simulink model "RB_KAIROS_ImpControl_OpSpace_quat_2020b_safety"  (R2020b)
(part 4 of 17)

t4722 = t17.*(t71-t391).*(-5.48359106408232e-4);
t4725 = t8.*(t71-t391).*(-5.187945860934245e-5);
t4740 = t16.*(t71-t391).*(-4.67845486573025e-5);
t4762 = t8.*t17.*(t71-t391).*(-2.74179553204116e-4);
t4779 = t3296.*(t386+t16.*(t69-t347)).*(-1.0./4.0);
t4788 = ((t395+t9.*(t48-t349)).*(t689-t740))./4.0;
t4790 = -t4761;
t4794 = t3286.*(t386+t16.*(t69-t347)).*(-1.0./4.0);
t4798 = t155+t255+t480+t841+t1384;
t4802 = t618.*(-8.36241330891889e-4);
t4803 = (t3296.*(t386+t16.*(t69-t347)))./4.0;
t4804 = t16.*(t71-t391).*(-2.454825983680473e-3);
t4807 = -t4789;
t4813 = (t3286.*(t386+t16.*(t69-t347)))./4.0;
t4817 = (t395+t9.*(t48-t349)).*(t1130-t16.*t17.*1.2516e-2).*(-1.0./4.0);
t4821 = t618.*8.36241330891889e-4;
t4829 = -t4815;
t4831 = -t4816;
t4832 = ((t395+t9.*(t48-t349)).*(t1130-t16.*t17.*1.2516e-2))./4.0;
t4837 = t1073+t1266+t2236;
t4848 = -t4839;
t4849 = t479+t534+t941+t1285;
t4883 = t1475+t3915;
t4888 = -t4878;
t4889 = t17.*(t380-t392).*(-2.74179553204116e-4);
t4901 = -t4886;
t4903 = t9.*(t380-t392).*(-8.36241330891889e-4);
t4904 = t17.*(t380-t392).*2.74179553204116e-4;
t4909 = -t4895;
t4910 = -t4897;
t4911 = -t4898;
t4921 = t3239.*(t383+t9.*(t380-t392)).*(-1.0./4.0);
t4929 = -t4915;
t4933 = -t4919;
t4935 = (t3239.*(t383+t9.*(t380-t392)))./4.0;
t4963 = (t454.*t4415)./4.0;
t4965 = -t4954;
t4967 = (t440.*t4432)./4.0;
t4968 = -t4957;
t4969 = -t4958;
t4971 = -t4961;
t4975 = t439.*t4533;
t4977 = t6.*t3270.*2.46255173325e-2;
t4985 = (t454.*t4495)./4.0;
t4988 = (t439.*t4476)./4.0;
t4991 = -t4979;
t4995 = t4383.*(t71-t391).*(-1.0./4.0);
t5000 = t4410.*(t77-t390).*(-1.0./4.0);
t5007 = t469+t897+t1178+t1491;
t5013 = -t4993;
t5017 = (t4383.*(t71-t391))./4.0;
t5020 = (t440.*t4515)./4.0;
t5032 = t3624.*(-3.867742437e-3);
t5035 = (t540.*t4410)./4.0;
t5036 = (t440.*t4551)./4.0;
t5037 = t4471.*(t71-t391).*(-1.0./4.0);
t5040 = (t439.*t4527)./4.0;
t5049 = (t439.*t4532)./4.0;
t5055 = t3624.*3.867742437e-3;
t5057 = (t4471.*(t71-t391))./4.0;
t5058 = t439.*t4689;
t5063 = t4477.*(t60-t394).*(-1.0./4.0);
t5071 = t4510.*(t71-t391).*(-1.0./4.0);
t5075 = (t4477.*(t60-t394))./4.0;
t5084 = t4506.*3.587895;
t5085 = t4507.*3.587895;
t5089 = (t4510.*(t71-t391))./4.0;
t5090 = (t539.*t4477)./4.0;
t5091 = (t439.*t4635)./4.0;
t5094 = t16.*t4477.*(t71-t391).*(-1.0./2.0);
t5096 = t4506.*3.228604;
t5097 = t4507.*3.228604;
t5102 = t4531.*(t71-t391).*(-1.0./4.0);
t5103 = t4534.*(t60-t394).*(-1.0./4.0);
t5109 = t4537.*1.225946;
t5110 = t4542.*1.225946;
t5112 = t4544.*1.225946;
t5114 = (t4531.*(t71-t391))./4.0;
t5120 = t4537.*3.587895;
t5123 = t4541.*3.587895;
t5124 = t4542.*3.587895;
t5126 = t4544.*3.587895;
t5129 = t8.*t4527.*(t71-t391).*(-1.0./4.0);
t5133 = (t539.*t4534)./4.0;
t5134 = (t439.*t4711)./4.0;
t5136 = t16.*t4534.*(t71-t391).*(-1.0./4.0);
t5143 = t4619.*(t71-t391).*(-1.0./4.0);
t5144 = t4582.*1.666555;
t5148 = t4716.*(t71-t391);
t5149 = t4581.*1.225946;
t5150 = t4582.*1.225946;
t5152 = t4586.*1.225946;
t5157 = t4723.*(t71-t391);
t5159 = t4578.*3.587895;
t5162 = t4581.*3.587895;
t5171 = (t4619.*(t71-t391))./4.0;
t5216 = t611+t2361+t2731;
t5218 = t613+t2365+t2733;
t5222 = (t6.*t5118)./4.0;
t5239 = (t14.*t5139)./4.0;
t5241 = -t5229;
t5244 = (t7.*t5163)./4.0;
t5256 = (t13.*t14.*t5118)./2.0;
t5263 = t4541.*1.8732399795e-1;
t5264 = t4544.*1.8732399795e-1;
t5265 = t4537.*9.5384188575e-2;
t5266 = t4542.*9.5384188575e-2;
t5269 = (t6.*t13.*t5139)./4.0;
t5271 = (t14.*t15.*t5163)./4.0;
t5276 = t4527.*(t380-t392).*(-1.0./2.0);
t5278 = t5.*t14.*t5139.*(-1.0./4.0);
t5280 = t4578.*1.8732399795e-1;
t5284 = t4581.*9.5384188575e-2;
t5288 = (t13.*t42.*t5139)./2.0;
t5294 = (t17.*t5233)./4.0;
t5298 = -t5282;
t5300 = -t5285;
t5306 = (t15.*t5254)./4.0;
t5310 = (t9.*t16.*t5233)./4.0;
t5317 = t16.*t4024.*4.38178973375e-3;
t5328 = (t5.*t5270)./4.0;
t5329 = t1097+t4772;
t5333 = t4432.*(t395+t9.*(t48-t349)).*(-1.0./4.0);
t5335 = (t7.*t14.*t5254)./4.0;
t5339 = -t5326;
t5341 = (t223.*t5118)./2.0;
t5346 = (t4432.*(t395+t9.*(t48-t349)))./4.0;
t5349 = (t12.*t13.*t5270)./2.0;
t5350 = (t9.*t5291)./4.0;
t5356 = t4477.*(t386+t16.*(t69-t347)).*(-1.0./4.0);
t5367 = -t5355;
t5368 = (t4477.*(t386+t16.*(t69-t347)))./4.0;
t5372 = (t7.*t5307)./4.0;
t5373 = (t16.*t17.*t5291)./4.0;
t5374 = (t6.*t5309)./4.0;
t5377 = (t319.*t5139)./2.0;
t5378 = (t320.*t5139)./2.0;
t5380 = t4515.*(t395+t9.*(t48-t349)).*(-1.0./4.0);
t5383 = -t5370;
t5387 = t4551.*(t395+t9.*(t48-t349)).*(-1.0./4.0);
t5389 = (t321.*t5163)./2.0;
t5394 = (t4515.*(t395+t9.*(t48-t349)))./4.0;
t5397 = t4534.*(t386+t16.*(t69-t347)).*(-1.0./4.0);
t5400 = (t14.*t15.*t5307)./2.0;
t5401 = (t13.*t14.*t5309)./2.0;
t5402 = (t4551.*(t395+t9.*(t48-t349)))./4.0;
t5406 = (t4534.*(t386+t16.*(t69-t347)))./4.0;
t5407 = -t5399;
t5410 = t6.*t4252.*2.46255173325e-2;
t5413 = -t5392;
t5414 = -t5393;
t5420 = -t5412;
t5426 = -t5416;
t5427 = (t325.*t5233)./2.0;
t5429 = (t225.*t5254)./2.0;
t5435 = -t5421;
t5447 = -t5432;
t5464 = -t5453;
t5473 = t4410.*(t383+t9.*(t380-t392)).*(-1.0./4.0);
t5483 = -t5462;
t5492 = (t4410.*(t383+t9.*(t380-t392)))./4.0;
t5497 = t3757+t3812;
t5504 = (t229.*t5291)./2.0;
t5506 = -t5498;
t5513 = (t223.*t5309)./4.0;
t5514 = t4506.*4.4422362436e-2;
t5515 = t3774+t3836;
t5516 = t4507.*6.3364582104e-2;
t5518 = t1458+t1480+t1953+t2002;
t5523 = t2079+t2253+t3330;
t5529 = -t5521;
t5532 = t744+t1015+t2242+t2264;
t5536 = t12.*t4507.*4.4422362436e-2;
t5542 = t12.*t4506.*6.3364582104e-2;
t5545 = (t321.*t5307)./4.0;
t5548 = t5163.*(t71-t391).*(-1.0./4.0);
t5551 = -t5533;
t5552 = t1576+t1660+t1996+t2021;
t5556 = -t5537;
t5561 = t1141+t1500+t2016+t2266;
t5564 = (t440.*t5233)./4.0;
t5566 = (t5163.*(t71-t391))./4.0;
t5573 = (t7.*t5494)./2.0;
t5580 = t1651+t1698+t2029+t2136;
t5581 = t4586.*2.5171736245e-2;
t5582 = t1371+t1797+t1969+t2179;
t5592 = t4582.*7.326866269e-3;
t5600 = t12.*t583.*t4507.*8.9697375e-1;
t5603 = (t15.*t5508)./2.0;
t5604 = t851+t1215+t2293+t2350;
t5606 = (t6.*t5517)./4.0;
t5609 = t1275+t1634+t2173+t2231;
t5614 = (t14.*t15.*t5494)./4.0;
t5625 = t1426+t1865+t1986+t2171;
t5628 = t1303+t5064;
t5634 = t951+t5095;
t5636 = (t7.*t14.*t5508)./4.0;
t5637 = t14.*t4557.*2.46255173325e-2;
t5640 = t987+t1598+t2244+t2344;
t5644 = t1348+t1686+t2218+t2340;
t5645 = (t13.*t14.*t5517)./4.0;
t5667 = -t5653;
t5680 = -t5669;
t5688 = (t439.*t5312)./4.0;
t5691 = (t439.*t5314)./4.0;
t5693 = t5291.*(t79-t358).*(-1.0./4.0);
t5699 = t571+t886+t1106+t1441+t1467;
t5705 = (t5291.*(t79-t358))./4.0;
t5712 = t5285.*1.225946;
t5720 = t5282.*3.587895;
t5721 = t5285.*3.587895;
t5730 = t17.*t4772.*1.13264871585e-2;
t5731 = -t5722;
t5736 = t5307.*(t71-t391).*(-1.0./4.0);
t5747 = (t225.*t5508)./4.0;
t5757 = (t321.*t5494)./4.0;
t5767 = (t223.*t5517)./2.0;
t5788 = -t5780;
t5793 = t6.*t5780;
t5800 = -t5790;
t5808 = t5282.*1.8732399795e-1;
t5812 = t5285.*9.5384188575e-2;
t5822 = t5392.*1.666555;
t5827 = t5392.*1.225946;
t5828 = t5393.*1.225946;
t5849 = -t5835;
t5850 = -t5836;
t5856 = -t5839;
t5857 = -t5840;
t5861 = t8.*t5835;
t5870 = (t6.*t5783)./4.0;
t5876 = t6.*t5839;
t5878 = -t5868;
t5881 = (t14.*t5807)./4.0;
t5883 = -t5872;
t5891 = (t13.*t14.*t5783)./4.0;
t5898 = -t5885;
t5899 = (t16.*t5810)./4.0;
t5904 = (t6.*t13.*t5807)./2.0;
t5906 = t5233.*(t395+t9.*(t48-t349)).*(-1.0./4.0);
t5917 = (t7.*t5829)./4.0;
t5922 = (t13.*t35.*t5783)./2.0;
t5924 = -t5903;
t5927 = (t5233.*(t395+t9.*(t48-t349)))./4.0;
t5930 = (t7.*t16.*t5810)./2.0;
t5931 = (t8.*t15.*t5810)./2.0;
t5934 = -t5913;
t5937 = -t5918;
t5938 = t5494.*(t71-t391).*(-1.0./2.0);
t5944 = -t5920;
t5945 = -t5921;
t5948 = (t16.*t5866)./4.0;
t5950 = (t15.*t16.*t5821)./2.0;
t5954 = (t14.*t15.*t5829)./2.0;
t5959 = (t5494.*(t71-t391))./2.0;
t5960 = -t5940;
t5962 = -t5942;
t5964 = t8.*t5903;
t5968 = (t8.*t5875)./4.0;
t5970 = (t16.*t5877)./4.0;
t5972 = (t15.*t44.*t5810)./4.0;
t5980 = t223.*t5780;
t5983 = -t5956;
t5984 = -t5957;
t5985 = -t5958;
t5987 = -t5965;
t5989 = (t8.*t5879)./4.0;
t5991 = (t17.*t5888)./4.0;
t6004 = (t8.*t15.*t5866)./4.0;
t6013 = (t15.*t5894)./4.0;
t6017 = -t6000;
t6020 = t7.*t16.*t5866.*(-1.0./4.0);
t6023 = (t15.*t16.*t5879)./4.0;
t6026 = (t3720.*t4681)./4.0;
t6027 = -t6008;
t6034 = -t6015;
t6037 = (t15.*t44.*t5866)./2.0;
t6039 = t7.*t8.*t5879.*(-1.0./4.0);
t6044 = (t7.*t14.*t5894)./2.0;
t6049 = -t6033;
t6051 = t7.*t5064.*1.059103943995e-1;
t6056 = (t15.*t39.*t5879)./2.0;
t6057 = -t6042;
t6061 = t223.*t5839;
t6065 = -t6050;
t6073 = (t223.*t5783)./2.0;
t6074 = (t224.*t5783)./2.0;
t6076 = t323.*t5835;
t6081 = (t8.*(t1254+t1943+t9.*t439.*1.196e-3+t439.*t1083))./4.0;
t6082 = t15.*t5095.*1.059103943995e-1;
t6086 = (t227.*t5810)./4.0;
t6087 = (t6.*t5988)./2.0;
t6089 = (t9.*t5990)./4.0;
t6100 = (t15.*t16.*(t1254+t1943+t9.*t439.*1.196e-3+t439.*t1083))./4.0;
t6111 = (t319.*t5807)./2.0;
t6113 = (t15.*t16.*t5981)./4.0;
t6115 = -t6098;
t6118 = (t13.*t14.*t5988)./4.0;
t6120 = -t6099;
t6121 = (t454.*t5709)./2.0;
t6122 = (t8.*t6029)./4.0;
t6128 = (t14.*t15.*t6005)./4.0;
t6129 = (t321.*t5829)./4.0;
t6132 = -t6119;
t6141 = (t227.*t5866)./2.0;
t6142 = (t228.*t5866)./2.0;
t6144 = (t323.*t5821)./4.0;
t6147 = t1422+t1647+t1671+t1848+t2236;
t6151 = t223.*t5942;
t6156 = -t6136;
t6161 = -t6139;
t6162 = -t6140;
t6164 = (t227.*t5877)./2.0;
t6165 = (t16.*t6064)./4.0;
t6171 = -t6152;
t6174 = t9.*t5213.*1.13264871585e-2;
t6176 = t323.*t5903;
t6179 = -t6163;
t6180 = t17.*t5217.*1.13264871585e-2;
t6184 = t16.*t321.*t5810.*(-1.0./4.0);
t6186 = (t225.*t5894)./4.0;
t6189 = -t6172;
t6192 = t5723.*(t71-t391).*(-1.0./4.0);
t6194 = (t323.*t5875)./2.0;
t6200 = -t6181;
t6201 = (t440.*t5761)./4.0;
t6202 = -t6185;
t6208 = (t325.*t5888)./4.0;
t6209 = (t323.*t5879)./2.0;
t6210 = (t324.*t5879)./2.0;
t6212 = -t6199;
t6219 = t16.*t321.*t5866.*(-1.0./4.0);
t6220 = t439.*t5835;
t6229 = -t6215;
t6232 = (t404.*t5866)./4.0;
t6235 = (t370.*t5879)./4.0;
t6238 = t9.*t439.*t5763.*(-1.0./4.0);
t6245 = -t6233;
t6247 = -t6234;
t6254 = t5777.*(t71-t391).*(-1.0./4.0);
t6258 = -t6249;
t6260 = (t223.*t5988)./2.0;
t6262 = (t229.*t5990)./4.0;
t6264 = (t323.*(t1254+t1943+t9.*t439.*1.196e-3+t439.*t1083))./4.0;
t6265 = (t440.*t5837)./4.0;
t6266 = (t5777.*(t71-t391))./4.0;
t6267 = t12.*t3350.*t4507.*8.07151e-1;
t6269 = (t323.*t5981)./2.0;
t6272 = (t439.*t5821)./4.0;
t6287 = t12.*t3405.*t4506.*8.07151e-1;
t6290 = t5810.*(t48-t349).*(-1.0./4.0);
t6291 = (t454.*t5847)./4.0;
t6293 = -t6277;
t6295 = t439.*t5903;
t6298 = (t3270.*t5137)./2.0;
t6303 = (t321.*t6005)./2.0;
t6307 = -t6292;
t6308 = -t6294;
t6311 = t17.*t439.*t5837.*(-1.0./4.0);
t6313 = (t323.*t6029)./4.0;
t6314 = (t439.*t5875)./4.0;
t6315 = (t227.*t6064)./4.0;
t6320 = t5810.*(t60-t394).*(-1.0./4.0);
t6332 = t5866.*(t48-t349).*(-1.0./4.0);
t6334 = (t440.*t5888)./2.0;
t6335 = -t6318;
t6336 = (t439.*t5879)./4.0;
t6340 = (t2008.*t5509)./4.0;
t6343 = t5829.*(t71-t391).*(-1.0./2.0);
t6348 = (t5866.*(t48-t349))./4.0;
t6349 = (t539.*t5810)./4.0;
t6351 = t5877.*(t48-t349).*(-1.0./4.0);
t6353 = t3720+t5080;
t6354 = t16.*t5810.*(t71-t391).*(-1.0./4.0);
t6358 = (t2087.*t5509)./4.0;
t6361 = t5845.*(t71-t391).*(-1.0./4.0);
t6362 = (t5829.*(t71-t391))./2.0;
t6365 = t5393.*2.5171736245e-2;
t6366 = (t5877.*(t48-t349))./4.0;
t6373 = t5392.*7.326866269e-3;
t6381 = (t5845.*(t71-t391))./4.0;
t6385 = t1023+t2359+t3051+t3184;
t6401 = t16.*t5866.*(t71-t391).*(-1.0./4.0);
t6408 = t1570+t2432+t2918+t3015;
t6410 = (t539.*t5866)./2.0;
t6413 = (t439.*t5981)./4.0;
t6417 = (t439.*(t1254+t1943+t9.*t439.*1.196e-3+t439.*t1083))./2.0;
t6422 = t8.*t5879.*(t71-t391).*(-1.0./4.0);
t6427 = t12.*t4507.*(t85+t338+t362+t375+t408+t5.*t12.*(7.9e+1./2.5e+2)).*8.9697375e-1;
t6430 = t4506+t4588;
t6433 = t5879.*(t113-t409).*(-1.0./2.0);
t6436 = t5990.*(t79-t358).*(-1.0./2.0);
t6438 = (t439.*t6029)./2.0;
t6441 = (t5879.*(t113-t409))./2.0;
t6442 = t4537+t4581;
t6447 = t4507+t4656;
t6454 = t6005.*(t71-t391).*(-1.0./4.0);
t6455 = t4541+t4651;
t6463 = (t6005.*(t71-t391))./4.0;
t6473 = t6064.*(t48-t349).*(-1.0./2.0);
t6503 = (t12.*t4507.*t4681)./4.0;
t6509 = t5879.*(t380-t392).*(-1.0./4.0);
t6511 = t5761.*(t395+t9.*(t48-t349)).*(-1.0./4.0);
t6518 = (t5879.*(t380-t392))./4.0;
t6522 = (t5761.*(t395+t9.*(t48-t349)))./4.0;
t6523 = -t6512;
t6527 = (t4024.*t5083)./2.0;
t6546 = t2436+t2455+t2857+t2929;
t6558 = -t6551;
t6563 = t5810.*(t386+t16.*(t69-t347)).*(-1.0./4.0);
t6566 = t5837.*(t395+t9.*(t48-t349)).*(-1.0./4.0);
t6567 = t7.*t5613.*1.059103943995e-1;
t6570 = -t6560;
t6571 = (t5810.*(t386+t16.*(t69-t347)))./4.0;
t6577 = -t6569;
t6581 = t15.*t5648.*1.059103943995e-1;
t6584 = t5866.*(t386+t16.*(t69-t347)).*(-1.0./4.0);
t6590 = t655+t1385+t1708+t1730+t1883+t2023;
t6594 = (t5866.*(t386+t16.*(t69-t347)))./4.0;
t6598 = -t6591;
t6600 = -t6592;
t6605 = t5888.*(t395+t9.*(t48-t349)).*(-1.0./4.0);
t6615 = t946+t1120+t1676+t1696+t1911+t2015;
t6617 = (t5888.*(t395+t9.*(t48-t349)))./4.0;
t6624 = (t12.*t4507.*t4916)./4.0;
t6625 = (t12.*t4506.*t4936)./4.0;
t6631 = t5763.*(t383+t9.*(t380-t392)).*(-1.0./2.0);
t6633 = t1185+t1248+t1522+t1561+t1945+t2035;
t6649 = t6.*t6223.*6.8635e-3;
t6656 = t15.*t6175.*8.639075e-2;
t6659 = t7.*t6196.*8.639075e-2;
t6663 = -t6651;
t6673 = t1025+t1195+t1726+t1732+t2037+t2117;
t6675 = t836+t1398+t1617+t1705+t2042+t2103;
t6687 = t1413+t1536+t1622+t1642+t2006+t2055;
t6726 = t7.*t5806.*1.059103943995e-1;
t6735 = (t4774.*(t2821-t2864))./4.0;
t6767 = t1902+t6223;
t6772 = t15.*t5860.*1.059103943995e-1;
t6781 = t724+t1606+t2375+t2945+t3128;
t6803 = t1324+t1498+t1852+t1856+t2081+t2326;
t6821 = (t4557.*t5115)./4.0;
t6822 = (t3270.*t5755)./2.0;
t6850 = -t6823;
t6873 = (t4024.*t5441)./2.0;
t6890 = -t6861;
t6951 = t1213+t1742+t1859+t1870+t2346+t2378;
t6983 = t1755+t1790+t1829+t1842+t2322+t2352;
t6992 = (t3270.*t5826)./4.0;
t7001 = (t3275.*t5843)./4.0;
t7113 = t722+t2456+t2481+t2925+t2947;
t7124 = t849+t2478+t2484+t2828+t2942;
t7132 = t5012+t5065;
t7133 = t6.*t7108;
t7134 = t14.*t7108;
t7178 = (t4517.*t5433)./4.0;
t7186 = (t536.*t6713)./4.0;
t7200 = -t7191;
t7215 = t3095+t3159+t3371+t3376;
t7217 = t3049+t3183+t3382+t3417;
t7220 = (t554.*t6713)./4.0;
t7238 = (t583.*t6693)./4.0;
t7242 = -t7228;
t7253 = (t3270.*t6222)./4.0;
t7255 = (t3275.*t6223)./4.0;
t7262 = (t4772.*t5433)./4.0;
t7265 = (t4252.*t5750)./4.0;
t7268 = -t7256;
t7276 = -t7254;
t7289 = t14.*t6750.*6.8635e-3;
t7303 = -t7275;
t7305 = -t7278;
t7306 = -t7279;
t7317 = -t7293;
t7320 = t5168+t5219;
t7323 = -t7302;
t7393 = (t1490.*t6713)./4.0;
t7423 = -t7399;
t7424 = -t7401;
t7436 = -t7429;
t7450 = (t1920.*t6713)./2.0;
t7453 = (t4557.*t5739)./4.0;
t7454 = t298+t7252;
t7459 = -t7452;
t7466 = (t4884.*t5543)./4.0;
t7477 = (t4959.*t5478)./4.0;
t7481 = -t7.*(t263-t7252);
t7483 = -t15.*(t263-t7252);
t7493 = t5478.*(t2959-t2967).*(-1.0./4.0);
t7504 = (t5478.*(t2959-t2967))./4.0;
t7519 = t5509.*(t2959-t2967).*(-1.0./4.0);
t7527 = -t7.*(-t262+t5078+t5282);
t7528 = -t15.*(-t262+t5078+t5282);
t7532 = (t5509.*(t2959-t2967))./4.0;
t7543 = (t3738.*t6397)./4.0;
t7558 = t7.*(-t262+t5078+t5282);
t7559 = t15.*(-t262+t5078+t5282);
t7563 = (t4557.*t5843)./2.0;
t7573 = (t5062.*t5478)./4.0;
t7591 = t189+t248+t7254;
t7604 = (t4896.*t5696)./4.0;
t7625 = (t4879.*t5713)./4.0;
t7628 = -t7606;
t7639 = t188+t247+t5044+t5285;
t7651 = -t7632;
t7655 = -t7637;
t7657 = (t4938.*t5696)./4.0;
t7668 = (t5696.*(t2889-t2921))./4.0;
t7674 = (t4917.*t5713)./4.0;
t7676 = t2354+t2896+t2939+t3103+t3145;
t7687 = (t5713.*(t2812-t2860))./4.0;
t7694 = (t2561.*t6750)./4.0;
t7697 = t7254.*1.225946;
t7699 = -t7680;
t7703 = t7252.*3.587895;
t7705 = t7254.*3.587895;
t7708 = (t2701.*t6713)./2.0;
t7709 = (t2701.*t6713)./4.0;
t7731 = t7275.*1.225946;
t7732 = t7277.*1.225946;
t7735 = t7278.*1.225946;
t7736 = t7279.*1.225946;
t7743 = t7275.*3.587895;
t7745 = t7278.*3.587895;
t7748 = t7277.*1.666555;
t7831 = t7399.*1.666555;
t7832 = t7401.*1.666555;
t7833 = t7399.*1.225946;
t7834 = t7254.*9.5384188575e-2;
t7835 = t7401.*1.225946;
t7845 = t7252.*1.8732399795e-1;
t7888 = (t3254.*t6750)./4.0;
t7907 = (t4557.*t6223)./2.0;
t7943 = -t7927;
t7952 = t5439+t5461;
t7955 = t15.*(t263-t7252).*(-1.666555);
t7959 = t7.*(t263-t7252).*(-1.225946);
t7960 = t15.*(t263-t7252).*(-1.225946);
t7970 = (t5365.*t5524)./4.0;
t8002 = t6750.*(t263-t283-t310+t1265).*(-1.0./2.0);
t8007 = (t5450.*t5478)./4.0;
t8008 = (t6693.*(t85+t338+t362+t375+t408+t5.*t12.*(7.9e+1./2.5e+2)))./2.0;
t8009 = (t3720.*t6713)./2.0;
t8020 = (t6750.*(t263-t283-t310+t1265))./2.0;
t8033 = (t4884.*(-t1272-t1479+t1647+t1848+t2236))./4.0;
t8035 = -t8019;
t8046 = t5.*t7108.*2.01382560198e-1;
t8047 = t721+t2454+t2483+t2911+t2924+t2948;
t8048 = -t8036;
t8053 = t823+t2477+t2485+t2814+t2856+t2951;
t8072 = t917+t1776+t2469+t2475+t3495+t3591;
t8081 = -t8061;
t8082 = -t8064;
t8084 = (t5331.*t5716)./4.0;
t8089 = -t8069;
t8095 = t9.*t7538.*1.539925e-2;
t8096 = t17.*t7540.*1.539925e-2;
t8110 = -t8093;
t8142 = -t8125;
t8147 = -t8130;
t8153 = -t8137;
t8204 = t7277.*7.326866269e-3;
t8217 = t7279.*2.5171736245e-2;
t8231 = -t8206;
t8232 = -t8210;
t8233 = -t8211;
t8256 = t1004+t2355+t2882+t2931+t3036+t3178;
t8261 = (t5064.*t6175)./4.0;
t8267 = (t5509.*t5681)./4.0;
t8272 = t248+t364+t1259+t7254;
t8278 = t4660+t6538;
t8297 = t3742+t4992+t5045;
t8299 = (t5331.*t5884)./4.0;
t8303 = t4721+t6539;
t8305 = (t5095.*t6196)./4.0;
t8333 = (t4252.*t6750)./2.0;
t8349 = -t8337;
t8394 = t7.*(t263-t7252).*(-2.5171736245e-2);
t8398 = t15.*(t263-t7252).*(-7.326866269e-3);
t8412 = t15.*(t263-t7252).*7.326866269e-3;
t8431 = (t12.*t4507.*t6713)./4.0;
t8441 = -t8435;
t8447 = t12.*t13.*t6713.*(t2425-t2468).*(-1.0./4.0);
t8448 = t583.*(t5453+t5.*(t2959-t2967).*3.587895).*(-1.0./4.0);
t8454 = (t12.*t13.*t6713.*(t2425-t2468))./4.0;
t8455 = (t583.*(t5453+t5.*(t2959-t2967).*3.587895))./4.0;
t8468 = t13.*(t5462+t5.*(t2959-t2967).*3.228604).*(-6.23745e-2);
t8475 = -t8465;
t8478 = -t8466;
t8482 = t13.*(t5462+t5.*(t2959-t2967).*3.228604).*6.23745e-2;
t8484 = (t4569.*t6750)./2.0;
t8485 = (t4557.*t6762)./2.0;
t8491 = -t8479;
t8492 = -t8480;
t8537 = t1572.*(t5453+t5.*(t2959-t2967).*3.587895).*(-1.0./4.0);
t8548 = (t1572.*(t5453+t5.*(t2959-t2967).*3.587895))./4.0;
t8606 = t2433+t2449+t3153+t3171+t3223+t3232;
t8634 = t8331.*(-7.35522e-1);
t8638 = t8331.*(-1.666555);
t8643 = t8331.*7.35522e-1;
t8646 = t8331.*1.666555;
t8651 = t8350.*(-7.35522e-1);
t8658 = t8350.*7.35522e-1;
t8670 = (t5696.*t6104)./2.0;
t8674 = (t5713.*t6092)./2.0;
t8675 = t7.*t8285.*8.639075e-2;
t8690 = t297+t309+t1056+t1250+t5078+t5282;
t8692 = t15.*t8310.*8.639075e-2;
t8784 = -t8768;
t8836 = -t8819;
t8841 = -t8823;
t8842 = -t8824;
t8874 = t5713.*(t985+t3399-t13.*t42.*1.01140545e-1-t7.*t223.*5.034347249e-2).*(-1.0./4.0);
t8898 = (t5713.*(t985+t3399-t13.*t42.*1.01140545e-1-t7.*t223.*5.034347249e-2))./4.0;
t8917 = t5193+t6984;
t8922 = t5210+t6985;
t8927 = t5201+t6981;
t8928 = -t8921;
t8942 = (t3489.*t7980)./4.0;
t8952 = t8331.*(-5.01208083475e-2);
t8962 = t8331.*5.01208083475e-2;
t8971 = t8350.*(-3.867742437e-3);
t8995 = t5490+t6693;
t9016 = (t3752.*(t917-t1669+t2469+t2475+t3495+t3591))./4.0;
t9055 = t5.*t8728.*6.23745e-2;
t9061 = t13.*t8734.*6.23745e-2;
t9072 = t264+t5048+t7278;
t9095 = (t3266.*t8437)./4.0;
t9099 = -t7.*(-t211+t5081+t7275);
t9101 = -t8.*(-t211+t5081+t7275);
t9102 = -t15.*(-t211+t5081+t7275);
t9103 = -t16.*(-t211+t5081+t7275);
t9119 = t7.*(-t211+t5081+t7275);
t9121 = t15.*(-t211+t5081+t7275);
t9122 = (t3362.*t8437)./4.0;
t9130 = (t8437.*(t923-t1076))./4.0;
t9133 = t8477.*(t701-t775).*(-1.0./4.0);
t9135 = (t3424.*t8438)./4.0;
t9141 = (t8477.*(t701-t775))./4.0;
t9143 = (t5696.*t6966)./2.0;
t9146 = (t5713.*t6928)./2.0;
t9157 = (t3365.*t8477)./4.0;
t9161 = (t3455.*t8477)./4.0;
t9168 = (t3249.*(t2433+t2449-t3048-t3102+t3223+t3232))./4.0;
t9184 = t6.*(-t262+t1056+t1250+t5078+t5282+t4.*t13.*1.0442e-1).*2.46255173325e-2;
t9201 = (t3424.*t8609)./4.0;
t9228 = t4936+t5438+t5482;
t9303 = (t4265.*t8437)./2.0;
t9315 = (t4152.*t8477)./2.0;
t9316 = t8.*(-t211+t5081+t7275).*(-7.35522e-1);
t9318 = t8.*(-t211+t5081+t7275).*(-1.666555);
t9320 = t16.*(-t211+t5081+t7275).*(-1.666555);
t9380 = (t3350.*t8734)./4.0;
t9384 = (t3405.*t8728)./4.0;
t9515 = t12.*t4507.*t8156.*8.07151e-1;
t9523 = t12.*t4506.*(-t3405+t4994+t5076).*(-8.07151e-1);
t9526 = t6750.*(t4650+t34.*(t2425-t2468)).*(-1.0./4.0);
t9527 = (t4774.*t8437)./4.0;
t9531 = (t6750.*(t4650+t34.*(t2425-t2468)))./4.0;
t9571 = t5.*t9218.*6.23745e-2;
t9583 = t12.*t13.*t9218.*6.23745e-2;
t9586 = t13.*(t2720-t8734).*6.23745e-2;
t9602 = t5.*t12.*(t2720-t8734).*6.23745e-2;
t9611 = t8.*(-t211+t5081+t7275).*(-5.01208083475e-2);
t9616 = (t1572.*t9215)./4.0;
t9619 = t16.*(-t211+t5081+t7275).*(-1.17633784675e-2);
t9621 = t8.*(-t211+t5081+t7275).*5.01208083475e-2;
t9628 = t16.*(-t211+t5081+t7275).*1.17633784675e-2;
t9643 = -t9638;
t9644 = -t9639;
t9686 = t269+t865+t1258+t5081+t7275;
t9702 = (t5696.*t7980)./2.0;
t9755 = (t5277.*t8437)./2.0;
t9812 = (t5290.*t8477)./2.0;
t9912 = (t3396.*t9218)./4.0;
t9914 = t5750.*(t263+t1265-t7252-t5.*t12.*1.0442e-1).*(-1.0./4.0);
t9915 = (t3356.*(t2720-t8734))./4.0;
t9934 = (t5524.*t8477)./2.0;
t9940 = (t9215.*(t85+t338+t362+t375+t408+t5.*t12.*(7.9e+1./2.5e+2)))./4.0;
t9976 = (t5713.*t8438)./2.0;
t9977 = (t5716.*t8437)./2.0;
t10108 = t6175.*(t7.*(t4650+t34.*(t2425-t2468))+t47.*(t2425-t2468)).*(-1.0./4.0);
t10109 = (t5713.*t8609)./4.0;
t10110 = (t5884.*t8437)./4.0;
t10114 = (t6175.*(t7.*(t4650+t34.*(t2425-t2468))+t47.*(t2425-t2468)))./4.0;
t10123 = t6196.*(t4654+t15.*(t4650+t34.*(t2425-t2468))).*(-1.0./4.0);
t10129 = (t6196.*(t4654+t15.*(t4650+t34.*(t2425-t2468))))./4.0;
t10143 = (t6713.*t7734)./4.0;
t10151 = (t12.*t4507.*t9218)./4.0;
t10156 = t12.*t13.*t9218.*(t2425-t2468).*(-1.0./4.0);
t10162 = (t12.*t4506.*(t2720-t8734))./4.0;
t10165 = (t12.*t13.*t9218.*(t2425-t2468))./4.0;
t10175 = t5.*t12.*(t2425-t2468).*(t2720-t8734).*(-1.0./4.0);
t10181 = (t5.*t12.*(t2425-t2468).*(t2720-t8734))./4.0;
t10201 = t5423+t5465+t6713;
t10249 = t6515+t8312;
t10270 = t6514+t8331;
t10406 = t6750.*(t263+t1265-t7252-t5.*t12.*1.0442e-1).*(-1.0./4.0);
t10411 = (t6750.*(t263+t1265-t7252-t5.*t12.*1.0442e-1))./4.0;
t10566 = -t8.*(-t244+t7279+t15.*(t257+t269)+t7.*(t263-t7252));
t10568 = -t16.*(-t244+t7279+t15.*(t257+t269)+t7.*(t263-t7252));
t10703 = t6955+t8635;
t10722 = (t6750.*(-t262+t1056+t1250+t5078+t5282+t4.*t13.*1.0442e-1))./4.0;
t10750 = t16.*(t8315+t8.*(t30.*(t2425-t2468)+t68.*(t2425-t2468))).*(-4.38178973375e-3);
t10752 = t16.*(t8315+t8.*(t30.*(t2425-t2468)+t68.*(t2425-t2468))).*4.38178973375e-3;
t10794 = t16.*(-t244+t7279+t15.*(t257+t269)+t7.*(t263-t7252)).*(-7.35522e-1);
t10797 = t8.*(-t244+t7279+t15.*(t257+t269)+t7.*(t263-t7252)).*(-1.666555);
t10798 = t16.*(-t244+t7279+t15.*(t257+t269)+t7.*(t263-t7252)).*(-1.666555);
t10840 = (t6216.*t9218)./2.0;
t10842 = (t6205.*(t2720-t8734))./2.0;
t10862 = t8156.*(t5462+t5.*(t2959-t2967).*3.228604).*(-1.0./2.0);
t10868 = (t8156.*(t5462+t5.*(t2959-t2967).*3.228604))./2.0;
t10940 = t16.*(-t244+t7279+t15.*(t257+t269)+t7.*(t263-t7252)).*(-5.01208083475e-2);
t10946 = t16.*(-t244+t7279+t15.*(t257+t269)+t7.*(t263-t7252)).*5.01208083475e-2;
t10950 = t8.*(-t244+t7279+t15.*(t257+t269)+t7.*(t263-t7252)).*(-1.17633784675e-2);
t10954 = t8.*(-t244+t7279+t15.*(t257+t269)+t7.*(t263-t7252)).*1.17633784675e-2;
t11140 = (t2904-t2927).*(t8315+t8.*(t30.*(t2425-t2468)+t68.*(t2425-t2468))).*(-1.0./4.0);
t11146 = ((t2904-t2927).*(t8315+t8.*(t30.*(t2425-t2468)+t68.*(t2425-t2468))))./4.0;
t11227 = t9218.*(t5026+t5.*(t2959-t2967)).*(-1.0./2.0);
t11231 = (t7108.*(t2720-t8734))./2.0;
t11237 = (t9218.*(t5026+t5.*(t2959-t2967)))./2.0;
t11262 = t4024.*(t16.*(t30.*(t2425-t2468)+t68.*(t2425-t2468)).*1.666555+t8.*(t7.*(t4650+t34.*(t2425-t2468))+t47.*(t2425-t2468)).*1.666555).*(-1.0./4.0);
t11301 = t3398+t3403+t3536+t3550+t6154+t6533;
t11315 = (t8156.*t8734)./2.0;
t11333 = t8728.*(-t3405+t4994+t5076).*(-1.0./2.0);
t11346 = t5365.*(t8315+t8.*(t30.*(t2425-t2468)+t68.*(t2425-t2468))).*(-1.0./4.0);
t11478 = (t7620.*(t2720-t8734))./2.0;
t11480 = (t7656.*t9218)./2.0;
t11620 = t6069.*(t8315+t8.*(t30.*(t2425-t2468)+t68.*(t2425-t2468))).*(-1.0./4.0);
t11622 = (t6069.*(t8315+t8.*(t30.*(t2425-t2468)+t68.*(t2425-t2468))))./4.0;
t12382 = t8332+t10271;
t12386 = t8350+t10272;
t12445 = t8477.*(t8315+t8.*(t30.*(t2425-t2468)+t68.*(t2425-t2468))).*(-1.0./4.0);
t12450 = (t8477.*(t8315+t8.*(t30.*(t2425-t2468)+t68.*(t2425-t2468))))./4.0;
t12562 = t8653+t10488;
t12569 = t17.*(t8329+t17.*(t16.*(t30.*(t2425-t2468)+t68.*(t2425-t2468))+t8.*(t7.*(t4650+t34.*(t2425-t2468))+t47.*(t2425-t2468)))).*(-1.13264871585e-2);
t13022 = t5433.*(t8329+t17.*(t16.*(t30.*(t2425-t2468)+t68.*(t2425-t2468))+t8.*(t7.*(t4650+t34.*(t2425-t2468))+t47.*(t2425-t2468)))).*(-1.0./4.0);
t13029 = (t5433.*(t8329+t17.*(t16.*(t30.*(t2425-t2468)+t68.*(t2425-t2468))+t8.*(t7.*(t4650+t34.*(t2425-t2468))+t47.*(t2425-t2468)))))./4.0;
t14553 = t3709+t3714+t3788+t4573+t4755+t5781+t5784+t6182+t6183+t6253+t6278;
t15781 = t3620+t3645+t3651+t3671+t4572+t4608+t4649+t4657+t4714+t4737+t6024+t6025+t6197+t6198+t6698+t6699+t6715+t6716;
t15891 = t2963+t3167+t3446+t3512+t3617+t3632+t3653+t3702+t3744+t4080+t4094+t4130+t4504+t4508+t4533+t4689+t5021+t5028+t5180+t5181+t5971+t5975+t6116+t6117+t6203+t6554;
t15892 = t3026+t3220+t3446+t3512+t3617+t3632+t3653+t3702+t3744+t4071+t4103+t4163+t4504+t4508+t4533+t4689+t5021+t5028+t5180+t5181+t5971+t5975+t6116+t6117+t6203+t6554;
t425 = -t415;
t460 = -t448;
t519 = t9.*t483;
t520 = t8.*t470;
t522 = t9.*t470;
t524 = t17.*t483;
t525 = t16.*t470;
t526 = t17.*t470;
t560 = t8.*t542;
t561 = t8.*t543;
t582 = -t563;
t605 = t356+t412;
t688 = -t598;
t718 = t9.*t586;
t729 = t17.*t586;
t753 = t392+t411;
t767 = t9.*t614;
t771 = t17.*t614;
t778 = t9.*t622;
t786 = t8.*t599;
t787 = t9.*t598;
t792 = -t616;
t793 = t17.*t598;
t797 = -t623;
t799 = t279+t451;
t1217 = -t9.*(t236-t451);
t1237 = -t17.*(t236-t451);
t1625 = t17.*(t236-t451);
t1818 = t9.*t1309;
t1824 = t17.*t1309;
t1913 = t443+t447;
t1933 = t417+t521;
t1934 = t418+t523;
t1940 = -t1919;
t1961 = t9.*t1904;
t1965 = t17.*t1904;
t2030 = -t1966;
t2069 = -t1981;
t2072 = -t1984;
t2082 = t412.*1.2516e-2;
t2129 = -t2061;
t2131 = -t2064;
t2144 = -t2073;
t2153 = -t2080;
t2226 = -t2121;
t2234 = -t2128;
t2245 = -t2141;
t2246 = -t2148;
t2248 = -t2151;
t2249 = -t2152;
t2250 = -t2155;
t2252 = -t2158;
t2256 = -t2165;
t2260 = -t2174;
t2265 = -t2185;
t2268 = -t2189;
t2269 = -t2191;
t2273 = -t2196;
t2275 = -t2199;
t2276 = -t2201;
t2277 = -t2204;
t2278 = -t2205;
t2282 = -t2209;
t2283 = -t2210;
t2285 = -t2212;
t2286 = t412.*6.1597e-2;
t2288 = -t2107;
t2289 = -t2108;
t2296 = t415.*6.1597e-2;
t2298 = -t2114;
t2299 = -t2115;
t2302 = -t2220;
t2303 = -t2221;
t2306 = -t2232;
t2311 = -t2235;
t2317 = -t2241;
t2318 = -t2243;
t2324 = t412.*4.28e-4;
t2329 = t412.*1.196e-3;
t2330 = t415.*4.28e-4;
t2332 = -t2251;
t2337 = t415.*1.0517e-2;
t2348 = -t2272;
t2356 = t415.*1.0027e-2;
t2358 = -t2300;
t2368 = -t2314;
t2369 = t412.*4.252e-3;
t2371 = -t2323;
t2381 = -t2341;
t2382 = -t2345;
t2392 = t415.*7.41e-4;
t2415 = -t2386;
t2428 = -t2372;
t2429 = -t2400;
t2435 = -t2412;
t2444 = t486.*1.2516e-2;
t2482 = t382+t1316;
t2490 = t532.*7.35522e-1;
t2494 = t485.*6.1597e-2;
t2495 = t486.*6.1597e-2;
t2504 = t531.*7.35522e-1;
t2506 = t485.*1.0517e-2;
t2507 = t486.*1.196e-3;
t2512 = t485.*1.0027e-2;
t2519 = t416+t1302;
t2524 = t486.*4.252e-3;
t2527 = t485.*4.28e-4;
t2528 = t486.*4.28e-4;
t2542 = -t9.*(t448+t16.*(t69-t347).*(1.1e+1./1.25e+2));
t2548 = -t17.*(t448+t16.*(t69-t347).*(1.1e+1./1.25e+2));
t2553 = t485.*7.41e-4;
t2646 = t9.*(t448+t16.*(t69-t347).*(1.1e+1./1.25e+2));
t2649 = t17.*(t448+t16.*(t69-t347).*(1.1e+1./1.25e+2));
t2660 = t562.*7.35522e-1;
t2663 = t563.*7.35522e-1;
t2665 = t578.*(-1.2516e-2);
t2698 = t578.*(-6.1597e-2);
t2699 = t8.*t2650;
t2717 = t578.*6.1597e-2;
t2718 = t8.*t2679;
t2724 = t578.*(-4.252e-3);
t2732 = t578.*(-4.28e-4);
t2734 = t578.*(-1.196e-3);
t2735 = t8.*t2670;
t2742 = t615.*7.35522e-1;
t2745 = t616.*7.35522e-1;
t2746 = t617.*7.35522e-1;
t2750 = t622.*7.35522e-1;
t2751 = t623.*7.35522e-1;
t2753 = t598.*7.35522e-1;
t2754 = t599.*7.35522e-1;
t2756 = t614.*1.666555;
t2758 = t616.*1.666555;
t2760 = t8.*t2704;
t2763 = t622.*1.666555;
t2767 = t598.*1.666555;
t2770 = t578.*4.252e-3;
t2783 = t578.*1.196e-3;
t2804 = -t2752;
t2815 = -t2764;
t3168 = t9.*(t236-t451).*(-7.35522e-1);
t3231 = -t3195;
t3234 = -t3205;
t3237 = -t3213;
t3384 = -t3333;
t3391 = -t3336;
t3428 = t9.*t3341;
t3429 = t587.*t1904;
t3433 = t17.*t3341;
t3439 = -t3341;
t3440 = -t3342;
t3500 = -t3436;
t3548 = -t3461;
t3549 = -t3464;
t3551 = -t3468;
t3552 = -t3471;
t3555 = -t3479;
t3559 = t412.*4.5305948634e-2;
t3562 = t2107.*1.666555;
t3563 = t2108.*1.666555;
t3565 = -t3486;
t3566 = t415.*4.5305948634e-2;
t3567 = t2114.*1.666555;
t3571 = -t3496;
t3574 = t2107.*1.225946;
t3575 = t2108.*1.225946;
t3577 = t2114.*1.225946;
t3578 = t2115.*1.225946;
t3583 = -t3517;
t3585 = -t3522;
t3590 = -t3528;
t3593 = -t3533;
t3594 = -t3535;
t3595 = -t3539;
t3596 = -t3543;
t3598 = -t3546;
t3607 = t798.*t1904;
t3613 = t687.*t1904;
t3616 = t689.*t1904;
t3623 = t701.*t1904;
t3626 = -t3573;
t3635 = t751.*t1904;
t3649 = t412.*3.127439544e-3;
t3657 = t775.*t1904;
t3658 = t415.*7.735484874e-3;
t3670 = t510+t2427;
t3680 = t906.*t1904;
t3682 = t8.*t3519;
t3686 = t16.*t3519;
t3693 = -t3666;
t3715 = t2372.*7.35522e-1;
t3718 = t2374.*7.35522e-1;
t3724 = -t9.*(t547+t2287);
t3728 = -t17.*(t547+t2287);
t3762 = t2467.*(-7.35522e-1);
t3768 = t2467.*(-1.666555);
t3785 = t2467.*7.35522e-1;
t3786 = -t3764;
t3790 = t2467.*1.666555;
t3793 = t485.*4.5305948634e-2;
t3796 = t486.*4.5305948634e-2;
t3803 = -t3775;
t3807 = t486.*3.127439544e-3;
t3809 = t485.*7.735484874e-3;
t3855 = -t3825;
t3902 = -t3853;
t3970 = t578.*(-4.5305948634e-2);
t3972 = t8.*t3901;
t3978 = t578.*(-3.127439544e-3);
t3991 = t578.*4.5305948634e-2;
t3995 = t562.*3.867742437e-3;
t4006 = t578.*3.127439544e-3;
t4013 = t563.*1.563719772e-3;
t4055 = t623.*3.867742437e-3;
t4059 = t616.*5.01208083475e-2;
t4068 = -t4048;
t4070 = t614.*1.17633784675e-2;
t4075 = t599.*1.563719772e-3;
t4089 = (t470.*t3173)./4.0;
t4134 = (t470.*t3230)./4.0;
t4205 = t9.*(t236-t451).*(-3.867742437e-3);
t4219 = t484.*(t689-t740).*(-1.0./4.0);
t4230 = -t4201;
t4236 = -t4204;
t4247 = (t484.*(t689-t740))./4.0;
t4250 = t470.*(t733-t806).*(-1.0./2.0);
t4254 = -t4226;
t4256 = (t483.*t3307)./4.0;
t4276 = (t470.*(t1165-t14.*t15.*3.5549e-2))./4.0;
t4282 = -t4258;
t4289 = -t4269;
t4299 = -t4277;
t4317 = -t4309;
t4327 = t3343.*7.35522e-1;
t4328 = t3347.*7.35522e-1;
t4329 = t3348.*7.35522e-1;
t4330 = t3349.*7.35522e-1;
t4332 = t3341.*1.666555;
t4333 = t3342.*1.666555;
t4334 = t3347.*1.666555;
t4335 = t3348.*1.666555;
t4385 = t3502.*7.35522e-1;
t4386 = t3503.*7.35522e-1;
t4389 = t3507.*7.35522e-1;
t4390 = t3508.*7.35522e-1;
t4400 = t3502.*1.666555;
t4402 = t3507.*1.666555;
t4404 = -t4373;
t4405 = t2107.*5.034347249e-2;
t4408 = -t4379;
t4409 = -t4380;
t4427 = -t4399;
t4431 = t2115.*2.5171736245e-2;
t4435 = -t4414;
t4439 = t2108.*7.326866269e-3;
t4440 = -t4416;
t4441 = -t4417;
t4442 = t412.*8.36241330891889e-4;
t4444 = t2114.*1.4653732538e-2;
t4449 = t415.*2.74179553204116e-4;
t4454 = -t4430;
t4458 = (t604.*t3296)./4.0;
t4463 = -t4438;
t4468 = (t604.*t3286)./4.0;
t4489 = t616+t1078+t1545;
t4498 = t622+t1333+t1544;
t4500 = t9.*(t547+t2287).*(-7.35522e-1);
t4501 = t17.*(t547+t2287).*(-7.35522e-1);
t4503 = -t4484;
t4505 = t620+t3507;
t4509 = t614+t1105+t1718;
t4520 = t2372.*3.867742437e-3;
t4539 = t2374.*1.563719772e-3;
t4545 = t800+t3502;
t4564 = t2467.*(-5.01208083475e-2);
t4574 = t243+t515+t548+t2115;
t4576 = t486.*8.36241330891889e-4;
t4580 = t485.*2.74179553204116e-4;
t4585 = t292+t499+t552+t2114;
t4589 = -t4540;
t4599 = t2467.*5.01208083475e-2;
t4618 = t210+t495+t572+t2107;
t4620 = -t4593;
t4629 = -t9.*(t624-t3502);
t4633 = -t17.*(t624-t3502);
t4639 = (t1907.*t3239)./4.0;
t4640 = t3887.*7.35522e-1;
t4643 = t3890.*7.35522e-1;
t4704 = t17.*(t624-t3502);
t4717 = (t1907.*t3280)./4.0;
t4757 = t578.*(-8.36241330891889e-4);
t4766 = (t1904.*t3307)./4.0;
t4785 = t578.*8.36241330891889e-4;
t4806 = -t4788;
t4823 = (t1907.*t3447)./4.0;
t4880 = (t2458.*t3239)./4.0;
t4902 = t2418.*(t689-t740).*(-1.0./4.0);
t4913 = (t2418.*(t689-t740))./4.0;
t4918 = t7.*t2966.*1.059103943995e-1;
t4920 = t15.*t2980.*1.059103943995e-1;
t4927 = t9.*t4883;
t4928 = t17.*t4883;
t4964 = t622+t2206+t2247;
t4972 = -t4963;
t4973 = t3347.*5.01208083475e-2;
t4974 = t3348.*5.01208083475e-2;
t4976 = -t4967;
t4982 = (t470.*t4415)./4.0;
t4984 = (t470.*t4451)./4.0;
t4986 = -t4977;
t4989 = t3341.*1.17633784675e-2;
t4990 = t3342.*1.17633784675e-2;
t4999 = -t4985;
t5003 = -t4988;
t5019 = (t470.*t4495)./4.0;
t5031 = t3503.*3.867742437e-3;
t5041 = -t5020;
t5050 = t497+t1104+t1154+t1513;
t5053 = t3508.*1.563719772e-3;
t5056 = -t5036;
t5060 = (t484.*t4515)./4.0;
t5061 = -t5040;
t5067 = -t5049;
t5073 = (t483.*t4527)./4.0;
t5098 = (t470.*t4587)./4.0;
t5100 = t9.*(t547+t2287).*(-3.867742437e-3);
t5108 = t17.*(t547+t2287).*(-1.563719772e-3);
t5116 = t4536.*3.228604;
t5117 = t4540.*3.228604;
t5119 = t4536.*3.587895;
t5122 = t4540.*3.587895;
t5131 = -t5110;
t5142 = -t5124;
t5155 = -t5134;
t5172 = -t5144;
t5176 = t9.*(t624-t3502).*(-7.35522e-1);
t5177 = -t5150;
t5183 = -t5159;
t5202 = (t604.*t4477)./4.0;
t5206 = t3887.*3.867742437e-3;
t5225 = t3890.*1.563719772e-3;
t5237 = -t5222;
t5246 = -t5239;
t5251 = (t604.*t4534)./2.0;
t5258 = -t5244;
t5268 = t5.*t5239;
t5272 = -t5264;
t5273 = -t5266;
t5279 = -t5269;
t5289 = -t5280;
t5302 = -t5294;
t5303 = (t1907.*t4410)./4.0;
t5316 = -t5306;
t5327 = -t5317;
t5340 = -t5328;
t5344 = (t1907.*t4499)./4.0;
t5345 = t955+t4798;
t5358 = -t5349;
t5363 = -t5350;
t5364 = (t1904.*t4527)./4.0;
t5388 = -t5374;
t5391 = -t5377;
t5404 = -t5389;
t5418 = (t1907.*t4701)./4.0;
t5419 = -t5410;
t5425 = (t2458.*t4410)./4.0;
t5474 = (t2418.*t4515)./4.0;
t5481 = t932+t1536+t1939+t2006;
t5511 = -t5504;
t5520 = -t5513;
t5522 = -t5514;
t5527 = -t5516;
t5534 = t4540.*4.4422362436e-2;
t5541 = t4536.*6.3364582104e-2;
t5553 = t1396+t1505+t2052+t2090;
t5555 = -t5536;
t5560 = -t5542;
t5563 = -t5545;
t5578 = -t5564;
t5583 = t1455+t1502+t2088+t2142;
t5586 = t1366+t1722+t2048+t2195;
t5605 = -t5581;
t5612 = -t5592;
t5619 = -t5600;
t5623 = -t5603;
t5626 = -t5606;
t5627 = (t470.*t5254)./4.0;
t5631 = -t5614;
t5635 = t2394+t2728+t2730;
t5646 = t2388+t2727+t2747;
t5654 = (t8.*t5532)./4.0;
t5655 = -t5636;
t5656 = -t5637;
t5660 = -t5645;
t5672 = t6.*t4611.*2.46255173325e-2;
t5678 = (t15.*t16.*t5532)./4.0;
t5689 = (t7.*t5604)./4.0;
t5690 = (t8.*t5580)./4.0;
t5692 = (t8.*t5582)./4.0;
t5697 = (t9.*t16.*t5561)./4.0;
t5704 = -t5691;
t5710 = (t14.*t15.*t5604)./4.0;
t5711 = (t15.*t16.*t5580)./4.0;
t5714 = (t15.*t16.*t5582)./4.0;
t5715 = (t16.*t5625)./4.0;
t5725 = -t5712;
t5726 = (t16.*t17.*t5609)./4.0;
t5729 = -t5721;
t5732 = (t8.*t15.*t5640)./4.0;
t5733 = (t8.*t15.*t5625)./4.0;
t5737 = t9.*t4798.*1.13264871585e-2;
t5741 = -t5730;
t5743 = t15.*t5218.*8.639075e-2;
t5746 = (t15.*t16.*t5644)./4.0;
t5753 = t7.*t5216.*8.639075e-2;
t5762 = -t5747;
t5771 = -t5757;
t5774 = -t5767;
t5796 = (t323.*t5532)./2.0;
t5816 = (t325.*t5561)./4.0;
t5817 = (t229.*t5609)./4.0;
t5819 = -t5808;
t5825 = -t5812;
t5848 = (t227.*t5640)./4.0;
t5851 = (t321.*t5604)./2.0;
t5852 = (t323.*t5580)./2.0;
t5854 = (t227.*t5625)./4.0;
t5855 = (t323.*t5582)./4.0;
t5880 = -t5870;
t5886 = (t323.*t5644)./4.0;
t5890 = t5.*t5870;
t5892 = -t5881;
t5905 = (t470.*t5508)./2.0;
t5907 = -t5891;
t5910 = -t5899;
t5925 = -t5904;
t5928 = t1124+t1306+t1950+t3519;
t5929 = t895+t1270+t2190+t3347;
t5936 = -t5917;
t5941 = (t439.*t5532)./4.0;
t5946 = -t5922;
t5949 = (t440.*t5561)./2.0;
t5951 = t508+t1293+t1542+t1779+t2467;
t5955 = t1711+t2011+t2445+t2509;
t5969 = -t5948;
t5973 = t1254+t1943+t2508+t2610;
t5974 = -t5950;
t5979 = -t5954;
t5992 = -t5972;
t5993 = t16.*t5007.*4.38178973375e-3;
t5995 = (t439.*t5580)./4.0;
t5996 = (t439.*t5582)./2.0;
t5999 = t547+t1070+t1648+t1929+t2287;
t6001 = (t1907.*t5291)./4.0;
t6003 = t7.*t5948;
t6006 = -t5989;
t6007 = -t5991;
t6021 = -t6004;
t6022 = t7.*t5989;
t6040 = -t6023;
t6041 = t1649+t2238+t2515+t2529;
t6043 = -t6026;
t6047 = (t439.*t5644)./2.0;
t6052 = t5609.*(t79-t358).*(-1.0./2.0);
t6055 = -t6037;
t6058 = t5640.*(t48-t349).*(-1.0./2.0);
t6059 = t5604.*(t71-t391).*(-1.0./4.0);
t6060 = -t6044;
t6063 = t5625.*(t48-t349).*(-1.0./2.0);
t6068 = -t6051;
t6070 = (t5609.*(t79-t358))./2.0;
t6077 = (t5640.*(t48-t349))./2.0;
t6078 = (t5604.*(t71-t391))./4.0;
t6080 = (t5625.*(t48-t349))./2.0;
t6083 = -t6073;
t6095 = -t6082;
t6114 = t156+t285+t332+t1318+t1418+t1991+t2003;
t6127 = -t6113;
t6134 = -t6121;
t6143 = t1244+t2124+t2677+t2697;
t6148 = -t6128;
t6153 = -t6129;
t6157 = (t470.*t5709)./4.0;
t6166 = t321.*t5899;
t6167 = -t6144;
t6188 = t1962+t2185+t2493+t2667;
t6191 = -t6174;
t6195 = -t6180;
t6207 = t321.*t5948;
t6211 = t1373+t2214+t2681+t2738;
t6214 = -t6201;
t6221 = -t6208;
t6224 = -t6209;
t6227 = t1720+t2270+t2642+t2786;
t6231 = (t470.*t5776)./4.0;
t6237 = t321.*t5989;
t6244 = -t6232;
t6248 = -t6235;
t6276 = t2172+t2230+t2567+t2644;
t6279 = -t6262;
t6282 = -t6264;
t6283 = -t6265;
t6286 = -t6269;
t6289 = -t6272;
t6305 = -t6291;
t6322 = (t470.*t5847)./4.0;
t6329 = -t6313;
t6330 = -t6314;
t6331 = -t6315;
t6339 = t17.*t5329.*1.13264871585e-2;
t6352 = -t6336;
t6356 = (t2008.*t5515)./4.0;
t6357 = -t6340;
t6368 = t5561.*(t395+t9.*(t48-t349)).*(-1.0./4.0);
t6369 = t5899.*(t71-t391);
t6371 = (t2087.*t5515)./4.0;
t6372 = -t6358;
t6383 = -t6365;
t6388 = (t5561.*(t395+t9.*(t48-t349)))./4.0;
t6391 = -t6373;
t6393 = (t470.*t5894)./2.0;
t6398 = (t1907.*t5609)./4.0;
t6407 = t8.*(-t2182+t2241+t696.*(t48-t349)+t891.*(t48-t349)).*(-1.0./4.0);
t6415 = t5948.*(t71-t391);
t6419 = (t8.*(-t2182+t2241+t696.*(t48-t349)+t891.*(t48-t349)))./4.0;
t6421 = -t6413;
t6425 = t15.*t16.*(-t2182+t2241+t696.*(t48-t349)+t891.*(t48-t349)).*(-1.0./4.0);
t6428 = t5989.*(t71-t391);
t6431 = t4536+t4547;
t6432 = (t604.*t5810)./2.0;
t6445 = -t6438;
t6449 = t15.*t6430;
t6452 = t7.*t6430;
t6458 = (t604.*t5866)./4.0;
t6460 = t14.*t6447;
t6461 = -t15.*(t4540+t5.*(t2425-t2468));
t6462 = t15.*t6447;
t6466 = t8.*t6442;
t6469 = t16.*t6442;
t6472 = t39.*t6430;
t6474 = t44.*t6430;
t6475 = t6.*t6447;
t6476 = -t7.*(t4540+t5.*(t2425-t2468));
t6477 = t7.*t6447;
t6491 = (t1907.*t5763)./4.0;
t6492 = t7.*t6455;
t6497 = t15.*t6455;
t6501 = -t39.*(t4540+t5.*(t2425-t2468));
t6504 = -t44.*(t4540+t5.*(t2425-t2468));
t6505 = t7.*(t4540+t5.*(t2425-t2468));
t6510 = -t6503;
t6517 = t39.*(t4540+t5.*(t2425-t2468));
t6525 = t323.*(-t2182+t2241+t696.*(t48-t349)+t891.*(t48-t349)).*(-1.0./4.0);
t6526 = t462+t493+t504+t1154+t1391+t1513+t2123;
t6534 = (t323.*(-t2182+t2241+t696.*(t48-t349)+t891.*(t48-t349)))./4.0;
t6540 = t466+t506+t535+t1085+t1197+t1433+t2127;
t6548 = (t1907.*t5834)./4.0;
t6552 = t2439+t2479+t2819+t2933;
t6574 = t7.*t5628.*1.059103943995e-1;
t6579 = t15.*t5634.*1.059103943995e-1;
t6585 = (t1904.*t5879)./4.0;
t6589 = t1288+t1494+t1957+t2084+t3268;
t6604 = (t2458.*t5763)./4.0;
t6607 = t439.*(-t2182+t2241+t696.*(t48-t349)+t891.*(t48-t349)).*(-1.0./2.0);
t6637 = t1113+t1142+t1485+t1499+t1964+t2187;
t6644 = (t2418.*t5837)./4.0;
t6645 = (t1907.*t5990)./4.0;
t6648 = (t7.*t6590)./4.0;
t6653 = t736+t1246+t1560+t1643+t2012+t2137;
t6662 = -t6649;
t6665 = -t6656;
t6667 = -t6659;
t6669 = (t14.*t15.*t6590)./4.0;
t6671 = (t9.*t6615)./4.0;
t6679 = (t4255.*t5216)./2.0;
t6681 = t2416+t2936+t2998+t3031;
t6686 = (t15.*t6633)./4.0;
t6690 = (t16.*t17.*t6615)./4.0;
t6697 = (t4286.*t5218)./2.0;
t6703 = t8.*t9.*t6615.*(-1.0./4.0);
t6709 = t852+t1214+t1364+t1805+t2216+t2281;
t6720 = t1192+t1363+t1444+t1797+t2071+t2179;
t6722 = (t16.*t41.*t6615)./4.0;
t6727 = t1334+t1359+t1808+t1814+t1972+t2259;
t6728 = (t7.*t14.*t6633)./4.0;
t6745 = (t6.*t6673)./4.0;
t6746 = (t15.*t6675)./4.0;
t6749 = -t6735;
t6773 = (t17.*t6687)./4.0;
t6776 = (t13.*t14.*t6673)./2.0;
t6778 = (t7.*t14.*t6675)./4.0;
t6780 = t712+t1593+t2408+t2838+t3121;
t6790 = t6.*t15.*t6675.*(-1.0./4.0);
t6797 = (t9.*t16.*t6687)./4.0;
t6814 = (t14.*t43.*t6675)./2.0;
t6816 = (t229.*t6615)./4.0;
t6817 = (t230.*t6615)./4.0;
t6819 = t8.*t17.*t6687.*(-1.0./4.0);
t6827 = (t321.*t6590)./2.0;
t6842 = (t16.*t45.*t6687)./4.0;
t6845 = -t6821;
t6849 = -t6822;
t6855 = t15.*(t4540+t5.*(t2425-t2468)).*(-1.666555);
t6863 = t15.*(t4540+t5.*(t2425-t2468)).*(-1.225946);
t6886 = (t225.*t6633)./2.0;
t6897 = (t4298.*t5329)./4.0;
t6909 = (t4611.*t5137)./4.0;
t6910 = t44.*(t4540+t5.*(t2425-t2468)).*(-1.666555);
t6917 = t1013+t1623+t1802+t1843+t2325+t2421;
t6924 = (t9.*t323.*t6615)./2.0;
t6961 = (t17.*t6803)./4.0;
t6967 = t515+t548+t939+t1484+t1830+t1951+t2115;
t6970 = t1646+t1770+t2312+t2370+t3784;
t6971 = (t223.*t6673)./2.0;
t6972 = (t225.*t6675)./2.0;
t6973 = (t226.*t6675)./2.0;
t6978 = (t405.*t6615)./2.0;
t6989 = (t9.*t16.*t6803)./4.0;
t6999 = t6.*t6430.*1.8732399795e-1;
t7004 = t14.*t6430.*9.5384188575e-2;
t7010 = t1737+t1761+t1819+t1885+t2391+t2399;
t7013 = t15.*t223.*t6675.*(-1.0./4.0);
t7022 = t1684+t1715+t1887+t1888+t2267+t2426;
t7024 = (t325.*t6687)./4.0;
t7025 = (t326.*t6687)./4.0;
t7036 = t6.*(t4540+t5.*(t2425-t2468)).*(-1.8732399795e-1);
t7041 = t14.*(t4540+t5.*(t2425-t2468)).*(-9.5384188575e-2);
t7048 = (t7.*t6951)./4.0;
t7054 = t6.*(t4540+t5.*(t2425-t2468)).*1.8732399795e-1;
t7056 = t14.*(t4540+t5.*(t2425-t2468)).*9.5384188575e-2;
t7059 = (t403.*t6675)./4.0;
t7060 = (t371.*t6687)./2.0;
t7061 = (t17.*t323.*t6687)./2.0;
t7065 = (t14.*t15.*t6951)./2.0;
t7068 = t6590.*(t71-t391).*(-1.0./2.0);
t7070 = (t9.*t6983)./4.0;
t7074 = t6615.*(t79-t358).*(-1.0./2.0);
t7086 = t9.*t439.*t6615.*(-1.0./4.0);
t7092 = (t470.*t6633)./2.0;
t7095 = (t16.*t17.*t6983)./4.0;
t7098 = t6615.*(t77-t390).*(-1.0./2.0);
t7115 = (t454.*t6675)./2.0;
t7119 = (t540.*t6615)./4.0;
t7130 = t207+t508+t1766+t1793+t2366+t2377+t2467;
t7136 = (t470.*t6675)./4.0;
t7138 = (t440.*t6687)./2.0;
t7146 = (t4453.*t5443)./4.0;
t7157 = (t484.*t6687)./2.0;
t7167 = t17.*t439.*t6687.*(-1.0./4.0);
t7170 = (t2966.*t6175)./2.0;
t7175 = (t2980.*t6196)./2.0;
t7184 = (t321.*t6951)./4.0;
t7193 = -t7186;
t7202 = t6687.*(t106-t414).*(-1.0./4.0);
t7209 = (t440.*t6803)./4.0;
t7212 = (t6687.*(t106-t414))./4.0;
t7223 = t5096+t5161;
t7226 = t5084+t5167;
t7234 = -t7220;
t7236 = t5097+t5182;
t7241 = t5085+t5185;
t7245 = t3021+t3084+t3425+t3513;
t7246 = t5109+t5149;
t7247 = t5120+t5162;
t7250 = -t7238;
t7266 = -t7253;
t7267 = -t7255;
t7271 = (t4798.*t5434)./4.0;
t7272 = -t7262;
t7273 = -t7265;
t7295 = (t1907.*t6615)./4.0;
t7301 = -t7289;
t7307 = t6.*t6767.*6.8635e-3;
t7309 = t15.*(t4540+t5.*(t2425-t2468)).*(-2.5171736245e-2);
t7316 = t14.*t6442.*2.46255173325e-2;
t7328 = t15.*(t4540+t5.*(t2425-t2468)).*2.5171736245e-2;
t7332 = t13.*t6430.*2.01382560198e-1;
t7337 = t17.*t6781.*1.539925e-2;
t7350 = t6951.*(t71-t391).*(-1.0./2.0);
t7359 = t6983.*(t79-t358).*(-1.0./4.0);
t7361 = t6.*t15.*(t4540+t5.*(t2425-t2468)).*(-7.326866269e-3);
t7363 = t6.*t6455.*2.46255173325e-2;
t7368 = t44.*(t4540+t5.*(t2425-t2468)).*(-1.17633784675e-2);
t7374 = t5.*t6447.*2.01382560198e-1;
t7376 = t13.*(t4540+t5.*(t2425-t2468)).*(-2.01382560198e-1);
t7378 = (t6983.*(t79-t358))./4.0;
t7381 = t44.*(t4540+t5.*(t2425-t2468)).*1.17633784675e-2;
t7385 = t12.*t13.*t6430.*(-2.01382560198e-1);
t7388 = t13.*(t4540+t5.*(t2425-t2468)).*2.01382560198e-1;
t7402 = t1268+t1462+t1760+t1807+t2373+t3841;
t7406 = -t7393;
t7434 = t1666+t1767+t1778+t1791+t2335+t3839;
t7446 = t1031+t1948+t2200+t2315+t2633+t2658;
t7451 = t6687.*(t395+t9.*(t48-t349)).*(-1.0./4.0);
t7457 = (t6687.*(t395+t9.*(t48-t349)))./4.0;
t7460 = (t4884.*t5518)./4.0;
t7462 = (t2458.*t6615)./2.0;
t7463 = -t7453;
t7478 = (t4611.*t5755)./4.0;
t7479 = t9.*(t1528+t1966+t2026-t2172+t587.*(t48-t349)+t689.*(t48-t349)).*(-1.0./4.0);
t7488 = t6615.*(t383+t9.*(t380-t392)).*(-1.0./4.0);
t7489 = t262+t5047+t5298;
t7492 = (t4959.*t5497)./4.0;
t7494 = (t9.*(t1528+t1966+t2026-t2172+t587.*(t48-t349)+t689.*(t48-t349)))./4.0;
t7500 = (t6615.*(t383+t9.*(t380-t392)))./4.0;
t7503 = t5497.*(t2959-t2967).*(-1.0./4.0);
t7506 = t16.*t17.*(t1528+t1966+t2026-t2172+t587.*(t48-t349)+t689.*(t48-t349)).*(-1.0./4.0);
t7507 = t1683+t2101+t2105+t2343+t2585+t2688;
t7512 = t7133.*3.587895;
t7513 = t7134.*3.587895;
t7516 = (t16.*t17.*(t1528+t1966+t2026-t2172+t587.*(t48-t349)+t689.*(t48-t349)))./4.0;
t7518 = (t4035.*t6175)./2.0;
t7520 = t7134.*1.225946;
t7521 = t1736+t2118+t2146+t2339+t2609+t2708;
t7522 = t6803.*(t395+t9.*(t48-t349)).*(-1.0./2.0);
t7524 = (t2418.*t6687)./2.0;
t7526 = t16.*t41.*(t1528+t1966+t2026-t2172+t587.*(t48-t349)+t689.*(t48-t349)).*(-1.0./4.0);
t7531 = t5515.*(t2959-t2967).*(-1.0./4.0);
t7535 = (t5552.*(t2904-t2927))./4.0;
t7539 = (t16.*t41.*(t1528+t1966+t2026-t2172+t587.*(t48-t349)+t689.*(t48-t349)))./4.0;
t7544 = (t4064.*t6196)./2.0;
t7548 = t7.*(t1212+t1980-t2222+t2272+t726.*(t69-t347)+t818.*(t69-t347)).*(-1.0./4.0);
t7560 = (t3752.*t6385)./4.0;
t7562 = (t3743.*t6408)./4.0;
t7564 = (t7.*(t1212+t1980-t2222+t2272+t726.*(t69-t347)+t818.*(t69-t347)))./4.0;
t7567 = (t4611.*t5826)./2.0;
t7579 = -t7563;
t7589 = (t5062.*t5497)./4.0;
t7590 = -t7573;
t7593 = t14.*t15.*(t1212+t1980-t2222+t2272+t726.*(t69-t347)+t818.*(t69-t347)).*(-1.0./4.0);
t7607 = (t14.*t15.*(t1212+t1980-t2222+t2272+t726.*(t69-t347)+t818.*(t69-t347)))./4.0;
t7608 = (t1907.*t6983)./2.0;
t7614 = (t4900.*t5699)./4.0;
t7616 = (t16.*(-t1595+t2118+t2146+t2339+t16.*(t69-t347).*1.09e-4-t768.*(t69-t347)))./4.0;
t7621 = t7.*t7113.*8.639075e-2;
t7623 = t6430.*(t1748-t1821).*(-1.0./4.0);
t7624 = -t7604;
t7633 = t229.*(t1528+t1966+t2026-t2172+t587.*(t48-t349)+t689.*(t48-t349)).*(-1.0./4.0);
t7634 = t230.*(t1528+t1966+t2026-t2172+t587.*(t48-t349)+t689.*(t48-t349)).*(-1.0./4.0);
t7641 = t15.*t7124.*8.639075e-2;
t7642 = t8.*t7591;
t7643 = -t7625;
t7645 = t16.*t7591;
t7648 = t7134.*9.5384188575e-2;
t7649 = (t8.*t15.*(-t1595+t2118+t2146+t2339+t16.*(t69-t347).*1.09e-4-t768.*(t69-t347)))./4.0;
t7652 = (t229.*(t1528+t1966+t2026-t2172+t587.*(t48-t349)+t689.*(t48-t349)))./4.0;
t7653 = (t230.*(t1528+t1966+t2026-t2172+t587.*(t48-t349)+t689.*(t48-t349)))./4.0;
t7658 = ((t4540+t5.*(t2425-t2468)).*(t1748-t1821))./4.0;
t7661 = t7133.*1.8732399795e-1;
t7666 = (t3833.*t6430)./4.0;
t7672 = -t7657;
t7678 = (t4939.*t5699)./4.0;
t7688 = -t7674;
t7690 = t8.*t7639;
t7693 = t16.*t7639;
t7700 = t3833.*(t4540+t5.*(t2425-t2468)).*(-1.0./4.0);
t7704 = -t7687;
t7714 = -t7694;
t7715 = -t7697;
t7718 = (t2568.*t6767)./4.0;
t7720 = (t3833.*(t4540+t5.*(t2425-t2468)))./4.0;
t7726 = -t7709;
t7733 = t405.*(t1528+t1966+t2026-t2172+t587.*(t48-t349)+t689.*(t48-t349)).*(-1.0./4.0);
t7749 = -t7731;
t7750 = -t7735;
t7751 = -t7736;
t7764 = t321.*(t1212+t1980-t2222+t2272+t726.*(t69-t347)+t818.*(t69-t347)).*(-1.0./2.0);
t7779 = (t321.*(t1212+t1980-t2222+t2272+t726.*(t69-t347)+t818.*(t69-t347)))./2.0;
t7793 = (t227.*(-t1595+t2118+t2146+t2339+t16.*(t69-t347).*1.09e-4-t768.*(t69-t347)))./4.0;
t7796 = t2912+t6781;
t7800 = t1394+t2224+t2404+t2442+t2871+t2932;
t7841 = t9.*t439.*(t1528+t1966+t2026-t2172+t587.*(t48-t349)+t689.*(t48-t349)).*(-1.0./2.0);
t7844 = ((t79-t358).*(t1528+t1966+t2026-t2172+t587.*(t48-t349)+t689.*(t48-t349)))./4.0;
t7846 = -t7833;
t7847 = -t7834;
t7848 = -t7835;
t7853 = (t9.*t439.*(t1528+t1966+t2026-t2172+t587.*(t48-t349)+t689.*(t48-t349)))./2.0;
t7854 = (t5329.*t5449)./4.0;
t7861 = t17.*(t1788+t2251+t2331-t2398+t587.*(t113-t409)+t689.*(t113-t409)).*(-1.0./4.0);
t7862 = (t5218.*t5628)./4.0;
t7863 = (t5216.*t5634)./4.0;
t7864 = t6.*t7320.*6.8635e-3;
t7866 = ((t77-t390).*(t1528+t1966+t2026-t2172+t587.*(t48-t349)+t689.*(t48-t349)))./4.0;
t7873 = (t17.*(t1788+t2251+t2331-t2398+t587.*(t113-t409)+t689.*(t113-t409)))./4.0;
t7886 = t9.*t16.*(t1788+t2251+t2331-t2398+t587.*(t113-t409)+t689.*(t113-t409)).*(-1.0./4.0);
t7893 = t540.*(t1528+t1966+t2026-t2172+t587.*(t48-t349)+t689.*(t48-t349)).*(-1.0./2.0);
t7902 = (t9.*t16.*(t1788+t2251+t2331-t2398+t587.*(t113-t409)+t689.*(t113-t409)))./4.0;
t7904 = -t7888;
t7917 = t6.*t3275.*t6430.*8.9697375e-1;
t7918 = t14.*t3270.*t6430.*8.9697375e-1;
t7926 = (t4611.*t6222)./2.0;
t7930 = (t3292.*t6767)./4.0;
t7932 = t2007+t2157+t2163+t2180+t3166+t3258;
t7938 = t9.*(t618.*4.28e-4-t1841-t2389+t2400-t2414+t17.*(t113-t409).*1.0027e-2).*(-1.0./4.0);
t7939 = ((t71-t391).*(t1212+t1980-t2222+t2272+t726.*(t69-t347)+t818.*(t69-t347)))./2.0;
t7944 = t6.*t3275.*(t4540+t5.*(t2425-t2468)).*(-8.9697375e-1);
t7945 = t14.*t3270.*(t4540+t5.*(t2425-t2468)).*(-8.9697375e-1);
t7950 = (t9.*(t618.*4.28e-4-t1841-t2389+t2400-t2414+t17.*(t113-t409).*1.0027e-2))./4.0;
t7957 = t6.*t3275.*(t4540+t5.*(t2425-t2468)).*8.9697375e-1;
t7958 = t14.*t3270.*(t4540+t5.*(t2425-t2468)).*8.9697375e-1;
t7962 = t16.*t17.*(t618.*4.28e-4-t1841-t2389+t2400-t2414+t17.*(t113-t409).*1.0027e-2).*(-1.0./4.0);
t7963 = t5452+t5483;
t7967 = (t48-t349).*(-t1595+t2118+t2146+t2339+t16.*(t69-t347).*1.09e-4-t768.*(t69-t347)).*(-1.0./2.0);
t7968 = t5440+t5464;
t7973 = (t16.*t17.*(t618.*4.28e-4-t1841-t2389+t2400-t2414+t17.*(t113-t409).*1.0027e-2))./4.0;
t7978 = ((t48-t349).*(-t1595+t2118+t2146+t2339+t16.*(t69-t347).*1.09e-4-t768.*(t69-t347)))./2.0;
t7983 = -t7970;
t7985 = t14.*t3424.*t6430.*3.064865e-1;
t7992 = (t5365.*t5552)./4.0;
t7996 = t7559.*(-1.666555);
t7998 = t7558.*(-1.225946);
t8000 = t7559.*(-1.225946);
t8003 = t2053+t2059+t2263+t2363+t3257+t3287;
t8006 = t14.*t3424.*(t4540+t5.*(t2425-t2468)).*(-3.064865e-1);
t8011 = (t4849.*t6175)./4.0;
t8012 = (t4837.*t6196)./4.0;
t8013 = t7559.*1.666555;
t8016 = t7559.*1.225946;
t8022 = t14.*t3424.*(t4540+t5.*(t2425-t2468)).*3.064865e-1;
t8023 = (t5450.*t5497)./4.0;
t8024 = -t8007;
t8025 = (t3643.*t6767)./2.0;
t8026 = -t8008;
t8027 = -t8009;
t8038 = t325.*(t1788+t2251+t2331-t2398+t587.*(t113-t409)+t689.*(t113-t409)).*(-1.0./4.0);
t8043 = -t8033;
t8044 = t2541+t2909+t2982+t3312+t3576;
t8050 = t2825+t7124;
t8051 = (t325.*(t1788+t2251+t2331-t2398+t587.*(t113-t409)+t689.*(t113-t409)))./4.0;
t8054 = t2964+t7113;
t8055 = t2164+t2294+t2308+t2313+t3278+t3282;
t8056 = (t5443.*t5523)./4.0;
t8057 = -t8046;
t8058 = (t5443.*t5518)./4.0;
t8060 = (t4681.*t6353)./4.0;
t8062 = t2473+t3064+t3151+t3207+t3766;
t8078 = (t8.*(t2053+t2059-t2177+t2363+t3257+t3287))./4.0;
t8088 = (t4286.*t6546)./4.0;
t8091 = t229.*(t618.*4.28e-4-t1841-t2389+t2400-t2414+t17.*(t113-t409).*1.0027e-2).*(-1.0./4.0);
t8103 = (t3743.*t6781)./4.0;
t8111 = -t8095;
t8112 = -t8096;
t8124 = (t15.*t16.*(t2053+t2059-t2177+t2363+t3257+t3287))./2.0;
t8127 = t1907.*(t1528+t1966+t2026-t2172+t587.*(t48-t349)+t689.*(t48-t349)).*(-1.0./2.0);
t8144 = (t1907.*(t1528+t1966+t2026-t2172+t587.*(t48-t349)+t689.*(t48-t349)))./2.0;
t8161 = (t4681.*t6430)./4.0;
t8163 = t440.*(t1788+t2251+t2331-t2398+t587.*(t113-t409)+t689.*(t113-t409)).*(-1.0./2.0);
t8175 = (t440.*(t1788+t2251+t2331-t2398+t587.*(t113-t409)+t689.*(t113-t409)))./2.0;
t8193 = t4681.*(t4540+t5.*(t2425-t2468)).*(-1.0./4.0);
t8207 = (t4681.*(t4540+t5.*(t2425-t2468)))./4.0;
t8228 = -t8204;
t8235 = (t5442.*t5699)./4.0;
t8236 = -t8217;
t8249 = (t2904-t2927).*(-t2149+t2205+t693.*(t48-t349)+t784.*(t48-t349)).*(-1.0./4.0);
t8265 = ((t2904-t2927).*(-t2149+t2205+t693.*(t48-t349)+t784.*(t48-t349)))./4.0;
t8273 = t310+t1415+t7454;
t8279 = (t4841.*t6430)./4.0;
t8280 = (t5515.*t5681)./4.0;
t8281 = -t8267;
t8282 = (t4843.*t6430)./4.0;
t8287 = ((t79-t358).*(t618.*4.28e-4-t1841-t2389+t2400-t2414+t17.*(t113-t409).*1.0027e-2))./2.0;
t8291 = (t323.*(t2053+t2059-t2177+t2363+t3257+t3287))./4.0;
t8304 = t4841.*(t4540+t5.*(t2425-t2468)).*(-1.0./4.0);
t8306 = t4843.*(t4540+t5.*(t2425-t2468)).*(-1.0./4.0);
t8307 = (t4843.*t6447)./4.0;
t8311 = t2458.*(t1528+t1966+t2026-t2172+t587.*(t48-t349)+t689.*(t48-t349)).*(-1.0./4.0);
t8313 = (t4843.*(t4540+t5.*(t2425-t2468)))./4.0;
t8322 = (t2458.*(t1528+t1966+t2026-t2172+t587.*(t48-t349)+t689.*(t48-t349)))./4.0;
t8335 = ((t383+t9.*(t380-t392)).*(t1528+t1966+t2026-t2172+t587.*(t48-t349)+t689.*(t48-t349)))./4.0;
t8336 = (t4905.*t6430)./4.0;
t8339 = (t3249.*t7217)./4.0;
t8340 = (t4916.*t6430)./4.0;
t8344 = (t4251.*t6767)./2.0;
t8353 = (t4930.*t6430)./4.0;
t8356 = (t4936.*t6430)./4.0;
t8358 = t4905.*(t4540+t5.*(t2425-t2468)).*(-1.0./4.0);
t8363 = t4916.*(t4540+t5.*(t2425-t2468)).*(-1.0./4.0);
t8364 = (t4916.*t6447)./4.0;
t8367 = (t4922.*t6447)./4.0;
t8368 = (t4905.*(t4540+t5.*(t2425-t2468)))./4.0;
t8372 = (t4916.*(t4540+t5.*(t2425-t2468)))./4.0;
t8374 = t4930.*(t4540+t5.*(t2425-t2468)).*(-1.0./4.0);
t8375 = (t439.*(t2053+t2059-t2177+t2363+t3257+t3287))./4.0;
t8378 = (t2904-t2927).*(t624+t2511-t3502-t9.*t439.*4.252e-3).*(-1.0./4.0);
t8379 = t4936.*(t4540+t5.*(t2425-t2468)).*(-1.0./4.0);
t8380 = (t4936.*t6447)./4.0;
t8381 = (t6442.*(t2821-t2864))./4.0;
t8382 = (t4930.*(t4540+t5.*(t2425-t2468)))./4.0;
t8386 = (t4936.*(t4540+t5.*(t2425-t2468)))./4.0;
t8397 = (t3421.*t7215)./4.0;
t8404 = (t3489.*t7215)./4.0;
t8430 = t7558.*(-2.5171736245e-2);
t8432 = t7559.*(-7.326866269e-3);
t8436 = t7558.*2.5171736245e-2;
t8456 = ((t395+t9.*(t48-t349)).*(t1788+t2251+t2331-t2398+t587.*(t113-t409)+t689.*(t113-t409)))./4.0;
t8457 = t5.*t7952.*6.23745e-2;
t8459 = (t3752.*t7217)./4.0;
t8490 = t6.*t4557.*t6430.*8.9697375e-1;
t8499 = -t8484;
t8500 = -t8485;
t8503 = t1907.*(t618.*4.28e-4-t1841-t2389+t2400-t2414+t17.*(t113-t409).*1.0027e-2).*(-1.0./4.0);
t8508 = (t4604.*t6767)./2.0;
t8509 = (t4611.*t6763)./2.0;
t8513 = t6.*t4557.*(t4540+t5.*(t2425-t2468)).*(-8.9697375e-1);
t8514 = t14.*t4611.*t6430.*8.9697375e-1;
t8534 = t14.*t4611.*(t4540+t5.*(t2425-t2468)).*(-8.9697375e-1);
t8541 = t7.*t8047.*8.639075e-2;
t8556 = t15.*t8053.*8.639075e-2;
t8565 = (t4255.*t7113)./4.0;
t8573 = t5365.*(-t2149+t2205+t693.*(t48-t349)+t784.*(t48-t349)).*(-1.0./4.0);
t8581 = (t4286.*t7124)./4.0;
t8596 = (t5365.*(-t2149+t2205+t693.*(t48-t349)+t784.*(t48-t349)))./4.0;
t8619 = (t5329.*t6397)./2.0;
t8628 = t233+t359+t1462+t2395+t2401+t2837+t2894+t3841;
t8660 = (t5331.*t6442)./4.0;
t8661 = (t14.*t5331.*t6430)./4.0;
t8665 = (t3249.*t7676)./4.0;
t8672 = t14.*t5331.*(t4540+t5.*(t2425-t2468)).*(-1.0./4.0);
t8678 = (t14.*t5331.*(t4540+t5.*(t2425-t2468)))./4.0;
t8689 = t757+t1209+t1252+t2989+t3132+t3366+t3400;
t8697 = t285+t339+t882+t1241+t5077+t5300;
t8769 = (t5598.*t6430)./4.0;
t8799 = t5598.*(t4540+t5.*(t2425-t2468)).*(-1.0./4.0);
t8803 = t3421.*(t3479-t3544+t2772.*(t48-t349)+t2775.*(t48-t349)).*(-1.0./4.0);
t8809 = (t5699.*t6385)./2.0;
t8818 = (t3421.*(t3479-t3544+t2772.*(t48-t349)+t2775.*(t48-t349)))./4.0;
t8825 = t3489.*(t3479-t3544+t2772.*(t48-t349)+t2775.*(t48-t349)).*(-1.0./4.0);
t8843 = (t3489.*(t3479-t3544+t2772.*(t48-t349)+t2775.*(t48-t349)))./4.0;
t8849 = (t4557.*t7320)./4.0;
t8869 = t4611.*(t30.*(t2425-t2468).*3.587895+t68.*(t2425-t2468).*3.587895).*(-1.0./4.0);
t8931 = t5029+t7133;
t8946 = (t14.*t5740.*t6430)./4.0;
t8948 = -t8942;
t8950 = t5066+t7134;
t8954 = (t6.*t5750.*t6430)./4.0;
t8968 = t14.*t5740.*(t4540+t5.*(t2425-t2468)).*(-1.0./4.0);
t8974 = t6.*t5750.*(t4540+t5.*(t2425-t2468)).*(-1.0./4.0);
t8977 = (t14.*t5740.*(t4540+t5.*(t2425-t2468)))./4.0;
t8978 = (t5628.*t6546)./2.0;
t8982 = -t8.*(t5027-t7134);
t8985 = -t16.*(t5027-t7134);
t8987 = (t6.*t5750.*(t4540+t5.*(t2425-t2468)))./4.0;
t8998 = t16.*(t5027-t7134);
t9015 = (t3265.*t8256)./4.0;
t9020 = -t9016;
t9027 = (t3360.*t8256)./4.0;
t9048 = t2406+t2463+t2465+t2900+t3006+t3055+t3445;
t9049 = t2402+t2447+t2489+t2916+t3076+t3126+t3438;
t9065 = (t3771.*t8256)./4.0;
t9082 = t14.*t5713.*t6430.*3.064865e-1;
t9083 = t8297.*(t1748-t1821).*(-1.0./4.0);
t9086 = t211+t5052+t7303;
t9087 = (t8297.*(t1748-t1821))./4.0;
t9090 = t7.*t9072;
t9091 = t15.*t9072;
t9092 = t14.*t5713.*(t4540+t5.*(t2425-t2468)).*(-3.064865e-1);
t9105 = (t3833.*t8297)./4.0;
t9108 = -t9095;
t9132 = -t9122;
t9137 = -t9130;
t9140 = t8.*(t5027-t7134).*(-1.666555);
t9144 = t8.*(t5027-t7134).*(-7.35522e-1);
t9150 = (t5699.*t6969)./2.0;
t9152 = -t9146;
t9156 = t197+t9072;
t9159 = t15.*t8922.*8.639075e-2;
t9163 = -t9157;
t9169 = (t5634.*t7113)./2.0;
t9170 = (t583.*t8995)./4.0;
t9176 = -t9168;
t9181 = (t5628.*t7124)./2.0;
t9190 = -t9184;
t9232 = (t4453.*t8256)./2.0;
t9263 = t1772+t1899+t2970+t7705;
t9270 = (t5329.*t7538)./2.0;
t9271 = (t5696.*t7215)./4.0;
t9273 = t1854+t1892+t3037+t7703;
t9275 = t3098+t3199+t3211+t3241+t3678+t4612;
t9278 = t935+t1664+t2450+t2472+t3065+t3109+t3389+t3457;
t9279 = (t5699.*t7217)./4.0;
t9285 = t157+t286+t1319+t1419+t1663+t1846+t7276;
t9317 = t9119.*(-1.666555);
t9319 = t9121.*(-1.666555);
t9322 = t9119.*(-1.225946);
t9323 = t9121.*(-1.225946);
t9327 = t9119.*1.666555;
t9331 = t9119.*1.225946;
t9332 = t9121.*1.225946;
t9350 = (t6353.*t6713)./4.0;
t9387 = t8.*(t5027-t7134).*(-5.01208083475e-2);
t9393 = t14.*(t5027-t7134).*(-2.46255173325e-2);
t9397 = t8.*(t5027-t7134).*5.01208083475e-2;
t9410 = t14.*(t5027-t7134).*2.46255173325e-2;
t9417 = (t6430.*t6693)./4.0;
t9435 = (t6430.*t6713)./4.0;
t9439 = (t4841.*t8297)./4.0;
t9450 = t6693.*(t4540+t5.*(t2425-t2468)).*(-1.0./4.0);
t9464 = t6713.*(t4540+t5.*(t2425-t2468)).*(-1.0./4.0);
t9465 = (t6447.*t6713)./4.0;
t9477 = (t6713.*(t4540+t5.*(t2425-t2468)))./4.0;
t9494 = (t6.*t6430.*t6750)./4.0;
t9496 = (t4905.*t8297)./4.0;
t9499 = t156+t285+t1318+t1418+t1991+t2003+t5077+t5300;
t9500 = (t3249.*t8927)./4.0;
t9502 = (t6442.*t6767)./4.0;
t9504 = (t14.*t6430.*t6767)./4.0;
t9509 = (t6455.*t6750)./4.0;
t9510 = t6.*t6750.*(t4540+t5.*(t2425-t2468)).*(-1.0./4.0);
t9514 = t14.*t6767.*(t4540+t5.*(t2425-t2468)).*(-1.0./4.0);
t9520 = t6767.*(t30.*(t2425-t2468)+t68.*(t2425-t2468)).*(-1.0./4.0);
t9525 = t1314+t1847+t2578+t2581+t3208+t3222+t3603+t3677;
t9536 = -t9527;
t9569 = t12.*t4507.*t8297.*8.9697375e-1;
t9573 = (t3752.*t8927)./4.0;
t9574 = t12.*t13.*t8297.*(t2425-t2468).*(-8.9697375e-1);
t9576 = (t5699.*t7676)./2.0;
t9577 = -t9571;
t9578 = t12.*t13.*t8297.*(t2425-t2468).*8.9697375e-1;
t9604 = t16.*(t3098+t3199+t3211-t3221+t3678+t4612).*2.62925e-3;
t9618 = (t8995.*(t85+t338+t362+t375+t408+t5.*t12.*(7.9e+1./2.5e+2)))./4.0;
t9637 = (t5275.*t8256)./2.0;
t9677 = t5696.*(t3479-t3544+t2772.*(t48-t349)+t2775.*(t48-t349)).*(-1.0./4.0);
t9685 = t872+t1404+t9072;
t9693 = (t4286.*t8922)./4.0;
t9712 = -t9702;
t9713 = (t5634.*t8047)./2.0;
t9722 = (t5628.*t8053)./2.0;
t9764 = -t9755;
t9774 = (t5699.*(t917-t1669+t2469+t2475+t3495+t3591))./4.0;
t9785 = (t5523.*t8256)./4.0;
t9792 = (t5518.*t8256)./4.0;
t9801 = t6430.*(-t2715+t3105+t5080.*3.228604).*(-1.0./4.0);
t9805 = (t5543.*t8256)./2.0;
t9815 = (t6430.*(-t2715+t3105+t5080.*3.228604))./4.0;
t9817 = (t6447.*t7422)./4.0;
t9825 = ((t4540+t5.*(t2425-t2468)).*(-t2715+t3105+t5080.*3.228604))./4.0;
t9830 = t314+t9686;
t9848 = t291+t2108+t5413+t7528;
t9855 = t243+t2115+t5414+t7558;
t9863 = (t5598.*t8297)./2.0;
t9864 = (t5598.*t8297)./4.0;
t9872 = (t5634.*t8285)./4.0;
t9898 = (t5628.*t8310)./4.0;
t9909 = (t5740.*t8272)./4.0;
t9919 = t3275.*(t1786+t2973-t7703-t5.*t12.*3.746479959e-1).*(-1.0./4.0);
t9939 = -t9934;
t9944 = (t5552.*t8477)./4.0;
t9959 = (t2821-t2864).*(t5027-t7134).*(-1.0./4.0);
t9965 = ((t2821-t2864).*(t5027-t7134))./4.0;
t10071 = t6430.*(t5462+t5.*(t2959-t2967).*3.228604).*(-1.0./4.0);
t10072 = (t8256.*(-t1272-t1479+t1647+t1848+t2236))./4.0;
t10074 = t6430.*(t5453+t5.*(t2959-t2967).*3.587895).*(-1.0./4.0);
t10075 = (t4021.*(t3098+t3199+t3211-t3221+t3678+t4612))./4.0;
t10083 = (t6430.*(t5462+t5.*(t2959-t2967).*3.228604))./4.0;
t10085 = (t6447.*t7952)./4.0;
t10088 = (t6430.*(t5453+t5.*(t2959-t2967).*3.587895))./4.0;
t10092 = t1853+t1891+t2869+t2960+t5489+t5720;
t10093 = (t5699.*(t2433+t2449-t3048-t3102+t3223+t3232))./4.0;
t10100 = ((t4540+t5.*(t2425-t2468)).*(t5462+t5.*(t2959-t2967).*3.228604))./4.0;
t10104 = ((t4540+t5.*(t2425-t2468)).*(t5453+t5.*(t2959-t2967).*3.587895))./4.0;
t10146 = t5331.*(t5027-t7134).*(-1.0./4.0);
t10148 = (t5331.*(t5027-t7134))./4.0;
t10157 = t14.*t9686.*2.46255173325e-2;
t10210 = t4557.*(t1786+t2973-t7703-t5.*t12.*3.746479959e-1).*(-1.0./4.0);
t10214 = (t4557.*(t1786+t2973-t7703-t5.*t12.*3.746479959e-1))./4.0;
t10258 = t8477.*(-t2149+t2205+t693.*(t48-t349)+t784.*(t48-t349)).*(-1.0./4.0);
t10302 = (t5699.*t8927)./4.0;
t10308 = (t14.*t6430.*t8437)./4.0;
t10313 = t6.*(-t1785+t2869+t2960+t5489+t5720+t4.*t13.*3.746479959e-1).*6.8635e-3;
t10319 = t14.*t8437.*(t4540+t5.*(t2425-t2468)).*(-1.0./4.0);
t10328 = t8477.*(t624+t2511-t3502-t9.*t439.*4.252e-3).*(-1.0./4.0);
t10337 = t5740.*(t5027-t7134).*(-1.0./4.0);
t10346 = (t5740.*(t5027-t7134))./4.0;
t10397 = (t6693.*t8297)./4.0;
t10398 = t1566+t1867+t3228+t3700+t3703+t4023+t4038+t4602;
t10416 = (t6767.*t8272)./4.0;
t10437 = (t536.*t10201)./4.0;
t10453 = (t554.*t10201)./4.0;
t10498 = (t1490.*t10201)./4.0;
t10519 = (t6430.*t8734)./4.0;
t10526 = (t6447.*t8728)./4.0;
t10532 = t8734.*(t4540+t5.*(t2425-t2468)).*(-1.0./4.0);
t10537 = (t1920.*t10201)./4.0;
t10538 = (t8734.*(t4540+t5.*(t2425-t2468)))./4.0;
t10542 = t259+t564+t7277+t7483;
t10543 = t244+t546+t7306+t7481;
t10695 = (t6430.*t8995)./4.0;
t10700 = (t2701.*t10201)./2.0;
t10701 = (t2701.*t10201)./4.0;
t10711 = t6952+t8646;
t10712 = t8995.*(t4540+t5.*(t2425-t2468)).*(-1.0./4.0);
t10716 = t6950+t8643;
t10729 = -t10722;
t10754 = t1787+t2799+t3025+t5468+t7745;
t10759 = t1864+t2794+t2969+t5491+t7743;
t10802 = (t3720.*t10201)./4.0;
t10854 = (t4557.*(-t1785+t2869+t2960+t5489+t5720+t4.*t13.*3.746479959e-1))./4.0;
t10870 = t16.*(t8646-t8.*(t30.*(t2425-t2468)+t68.*(t2425-t2468)).*1.666555).*2.62925e-3;
t10873 = t7952.*(-t3405+t4994+t5076).*(-1.0./2.0);
t10892 = (t6430.*t9218)./4.0;
t10898 = (t6430.*t9215)./4.0;
t10901 = t8297.*(t5453+t5.*(t2959-t2967).*3.587895).*(-1.0./2.0);
t10904 = t9218.*(t4540+t5.*(t2425-t2468)).*(-1.0./4.0);
t10905 = (t6447.*t9218)./4.0;
t10906 = (t8297.*(t5453+t5.*(t2959-t2967).*3.587895))./2.0;
t10908 = (t6430.*(t2720-t8734))./4.0;
t10911 = t9215.*(t4540+t5.*(t2425-t2468)).*(-1.0./4.0);
t10913 = (t9218.*(t4540+t5.*(t2425-t2468)))./4.0;
t10919 = (t9215.*(t4540+t5.*(t2425-t2468)))./4.0;
t10924 = (t4540+t5.*(t2425-t2468)).*(t2720-t8734).*(-1.0./4.0);
t10925 = (t6447.*(t2720-t8734))./4.0;
t10934 = ((t4540+t5.*(t2425-t2468)).*(t2720-t8734))./4.0;
t10957 = (t12.*t4507.*t10201)./4.0;
t10976 = t12.*t13.*t10201.*(t2425-t2468).*(-1.0./4.0);
t10985 = (t12.*t13.*t10201.*(t2425-t2468))./4.0;
t10993 = (t5740.*t9686)./4.0;
t11041 = t8256.*(t4654+t15.*(t4650+t34.*(t2425-t2468))).*(-1.0./4.0);
t11046 = (t8256.*(t4654+t15.*(t4650+t34.*(t2425-t2468))))./4.0;
t11154 = (t3421.*(t8643-t8.*(t30.*(t2425-t2468)+t68.*(t2425-t2468)).*7.35522e-1))./4.0;
t11170 = (t3489.*(t8643-t8.*(t30.*(t2425-t2468)+t68.*(t2425-t2468)).*7.35522e-1))./4.0;
t11228 = t546+t1328+t1409+t1831+t7306+t7481;
t11247 = t564+t1629+t1661+t1834+t7277+t7483;
t11279 = (t4021.*(t8646-t8.*(t30.*(t2425-t2468)+t68.*(t2425-t2468)).*1.666555))./4.0;
t11331 = (t943-t1091).*(-t1053-t3327+t5081.*1.225946+t7731+t15.*t223.*1.4653732538e-2).*(-1.0./4.0);
t11335 = ((t943-t1091).*(-t1053-t3327+t5081.*1.225946+t7731+t15.*t223.*1.4653732538e-2))./4.0;
t11461 = (t6767.*t9686)./4.0;
t11473 = (t8297.*t8995)./2.0;
t11519 = t8437.*(t5027-t7134).*(-1.0./4.0);
t11522 = (t8437.*(t5027-t7134))./4.0;
t11651 = -t8.*(t210+t2107+t7423+t9121);
t11652 = -t9.*(t210+t2107+t7423+t9121);
t11653 = -t16.*(t210+t2107+t7423+t9121);
t11654 = -t17.*(t210+t2107+t7423+t9121);
t11671 = t16.*(t210+t2107+t7423+t9121);
t11672 = t17.*(t210+t2107+t7423+t9121);
t11683 = (t6353.*t10201)./2.0;
t11708 = (t6430.*t10201)./4.0;
t11721 = t10201.*(t4540+t5.*(t2425-t2468)).*(-1.0./4.0);
t11722 = (t6447.*t10201)./4.0;
t11730 = (t10201.*(t4540+t5.*(t2425-t2468)))./4.0;
t11759 = (t8297.*t9215)./2.0;
t11846 = t8.*(t210+t2107+t7423+t9121).*(-1.666555);
t11851 = (t5696.*(t8643-t8.*(t30.*(t2425-t2468)+t68.*(t2425-t2468)).*7.35522e-1))./4.0;
t11852 = t9.*(t210+t2107+t7423+t9121).*(-7.35522e-1);
t11980 = t5713.*(-t1053-t3327+t5081.*1.225946+t7731+t15.*t223.*1.4653732538e-2).*(-1.0./4.0);
t11983 = (t5713.*(-t1053-t3327+t5081.*1.225946+t7731+t15.*t223.*1.4653732538e-2))./4.0;
t11988 = t10201.*(t5026+t5.*(t2959-t2967)).*(-1.0./2.0);
t11993 = (t10201.*(t5026+t5.*(t2959-t2967)))./2.0;
t12007 = t8.*(t210+t2107+t7423+t9121).*(-1.17633784675e-2);
t12018 = t8.*t9.*(t210+t2107+t7423+t9121).*(-1.563719772e-3);
t12023 = t8.*t9.*(t210+t2107+t7423+t9121).*1.563719772e-3;
t12146 = (t7734.*t10201)./2.0;
t12185 = t2600+t3092+t3124+t3141+t7732+t7960;
t12563 = t8658+t10489;
t12669 = t1314+t2581+t3208+t3222+t3603+t3677+t7748+t7955;
t13186 = t5329.*(t9.*(t16.*(t30.*(t2425-t2468)+t68.*(t2425-t2468))+t8.*(t7.*(t4650+t34.*(t2425-t2468))+t47.*(t2425-t2468))).*7.35522e-1+t17.*(t4654+t15.*(t4650+t34.*(t2425-t2468))).*7.35522e-1).*(-1.0./4.0);
t14558 = q5d.*t14553;
t15782 = q5d.*t15781;
t15893 = q5d.*t15892;
t579 = t520.*(1.1e+1./1.25e+2);
t581 = t525.*(1.1e+1./1.25e+2);
t754 = t350+t425;
t1108 = -t778;
t1123 = t9.*t688;
t1837 = t351+t524;
t1840 = t354+t520;
t1905 = t396+t519;
t1906 = t387+t525;
t2043 = t9.*t1913;
t2049 = t17.*t1913;
t2096 = -t1965;
t2351 = -t2286;
t2357 = -t2296;
t2380 = -t2337;
t2423 = -t2392;
t2466 = t460+t580;
t2492 = t526.*1.2516e-2;
t2505 = t519.*1.2516e-2;
t2513 = -t2494;
t2514 = -t2495;
t2516 = t520.*4.815e-3;
t2518 = t525.*4.815e-3;
t2522 = t522+t561;
t2534 = t520.*4.354e-3;
t2537 = t525.*4.354e-3;
t2538 = -t2512;
t2539 = t519.*6.1597e-2;
t2543 = t522.*6.1597e-2;
t2545 = t524.*6.1597e-2;
t2550 = t526.*6.1597e-2;
t2557 = t520.*6.0149e-2;
t2559 = t525.*6.0149e-2;
t2560 = -t2527;
t2563 = t520.*1.196e-3;
t2566 = t526.*4.28e-4;
t2569 = t520.*1.0517e-2;
t2571 = t522.*1.0517e-2;
t2573 = t524.*1.0517e-2;
t2574 = t525.*1.196e-3;
t2575 = t526.*1.196e-3;
t2579 = t525.*1.0517e-2;
t2589 = t520.*1.158e-3;
t2593 = t525.*1.158e-3;
t2597 = t522.*1.0027e-2;
t2599 = t524.*1.0027e-2;
t2611 = t520.*1.964e-3;
t2612 = t526+t578;
t2613 = t519.*4.252e-3;
t2615 = t525.*1.964e-3;
t2616 = t520.*4.252e-3;
t2621 = t525.*4.252e-3;
t2622 = t526.*4.252e-3;
t2624 = t520.*1.4117e-2;
t2625 = t519.*4.28e-4;
t2626 = t525.*1.4117e-2;
t2627 = t519.*1.196e-3;
t2628 = t522.*4.28e-4;
t2630 = t524.*4.28e-4;
t2636 = t520.*3.41e-4;
t2640 = t525.*3.41e-4;
t2652 = t520.*7.41e-4;
t2654 = t522.*7.41e-4;
t2656 = t524.*7.41e-4;
t2657 = t525.*7.41e-4;
t2668 = t525.*1.09e-4;
t2683 = -t2663;
t2689 = t520.*1.09e-4;
t2796 = -t2745;
t2803 = -t2751;
t2807 = -t2753;
t2824 = -t2767;
t2850 = t767.*7.35522e-1;
t2853 = t771.*7.35522e-1;
t2862 = t778.*7.35522e-1;
t2865 = t786.*7.35522e-1;
t2866 = t787.*7.35522e-1;
t2867 = t793.*7.35522e-1;
t2923 = t718.*7.35522e-1;
t2928 = t729.*7.35522e-1;
t3175 = t1625.*(-7.35522e-1);
t3225 = t1625.*7.35522e-1;
t3251 = t1818.*7.35522e-1;
t3253 = t1824.*7.35522e-1;
t3284 = t486+t1961;
t3434 = t9.*(t348-t525).*(-1.2516e-2);
t3560 = -t3428;
t3580 = t1961.*6.1597e-2;
t3581 = t9.*(t348-t525).*(-6.1597e-2);
t3582 = t1965.*6.1597e-2;
t3584 = t17.*(t348-t525).*(-6.1597e-2);
t3600 = t9.*(t348-t525).*(-4.252e-3);
t3610 = -t3559;
t3611 = -t3562;
t3612 = -t3563;
t3615 = t9.*(t348-t525).*(-4.28e-4);
t3618 = -t3566;
t3619 = -t3567;
t3621 = t9.*(t348-t525).*(-1.196e-3);
t3622 = t17.*(t348-t525).*(-4.28e-4);
t3625 = t17.*(t348-t525).*(-1.0517e-2);
t3627 = -t3574;
t3628 = -t3575;
t3630 = -t3577;
t3631 = -t3578;
t3638 = t17.*(t348-t525).*(-1.0027e-2);
t3660 = t775.*(t348-t525);
t3668 = t798.*(t348-t525);
t3669 = t1965.*(-1.0517e-2);
t3672 = t701.*(t348-t525);
t3676 = t751.*(t348-t525);
t3684 = t17.*(t348-t525).*(-7.41e-4);
t3688 = -t3658;
t3701 = t1965.*(-7.41e-4);
t3706 = t906.*(t348-t525);
t3723 = -t3682;
t3735 = t9.*t3670;
t3736 = -t3715;
t3739 = t17.*t3670;
t3820 = -t3793;
t3822 = -t3796;
t3823 = t526.*4.5305948634e-2;
t3848 = t519.*4.5305948634e-2;
t3849 = t522.*4.5305948634e-2;
t3851 = t524.*4.5305948634e-2;
t3870 = t520.*2.3526756935e-2;
t3871 = t519.*3.127439544e-3;
t3872 = t520.*1.7527158935e-2;
t3874 = t525.*2.3526756935e-2;
t3875 = t520.*3.127439544e-3;
t3878 = t525.*1.7527158935e-2;
t3879 = t525.*3.127439544e-3;
t3880 = t526.*3.127439544e-3;
t3882 = t520.*7.735484874e-3;
t3884 = t522.*7.735484874e-3;
t3886 = t524.*7.735484874e-3;
t3888 = t525.*7.735484874e-3;
t3894 = t520.*1.00241616695e-1;
t3897 = t525.*1.00241616695e-1;
t3916 = t2646.*(-7.35522e-1);
t3921 = t2649.*(-7.35522e-1);
t3942 = t2646.*7.35522e-1;
t3949 = t2649.*7.35522e-1;
t4014 = -t3995;
t4034 = -t4013;
t4076 = -t4055;
t4083 = -t4059;
t4093 = t771.*3.867742437e-3;
t4099 = t793.*3.867742437e-3;
t4101 = -t4075;
t4112 = -t4089;
t4116 = t767.*1.563719772e-3;
t4125 = t787.*1.563719772e-3;
t4166 = -t4134;
t4237 = t1625.*(-1.563719772e-3);
t4279 = t1818.*3.867742437e-3;
t4280 = -t4256;
t4297 = -t4276;
t4301 = t1824.*1.563719772e-3;
t4351 = -t4332;
t4352 = -t4333;
t4358 = t1961.*4.5305948634e-2;
t4359 = t9.*(t348-t525).*(-4.5305948634e-2);
t4360 = t1965.*4.5305948634e-2;
t4361 = t17.*(t348-t525).*(-4.5305948634e-2);
t4362 = t3428.*7.35522e-1;
t4363 = t3433.*7.35522e-1;
t4382 = (t605.*t3239)./4.0;
t4392 = t1961.*3.127439544e-3;
t4395 = t9.*(t348-t525).*(-3.127439544e-3);
t4398 = t1965.*7.735484874e-3;
t4401 = t17.*(t348-t525).*(-7.735484874e-3);
t4424 = t2769.*(t348-t525);
t4428 = t2778.*(t348-t525);
t4455 = -t4431;
t4457 = t3686.*7.35522e-1;
t4459 = t3682.*1.666555;
t4461 = t3686.*1.666555;
t4464 = -t4439;
t4465 = -t4442;
t4478 = -t4458;
t4492 = -t4468;
t4493 = t603+t3440;
t4514 = t688+t1153+t1514;
t4543 = -t4520;
t4554 = -t9.*(t3682+t16.*(t295-t13.*t42.*(3.3e+1./4.0e+2)));
t4555 = -t17.*(t3682+t16.*(t295-t13.*t42.*(3.3e+1./4.0e+2)));
t4560 = -t4539;
t4565 = t9.*t4505;
t4566 = t17.*t4505;
t4575 = t258+t478+t550+t2289;
t4605 = t17.*(t3682+t16.*(t295-t13.*t42.*(3.3e+1./4.0e+2)));
t4613 = -t4576;
t4616 = -t4580;
t4623 = t525.*1.037589172186849e-4;
t4648 = t519.*8.36241330891889e-4;
t4652 = t526.*8.36241330891889e-4;
t4658 = t522.*2.74179553204116e-4;
t4659 = t524.*2.74179553204116e-4;
t4669 = t3239.*(t357-t519).*(-1.0./4.0);
t4675 = -t4639;
t4684 = t520.*9.3569097314605e-5;
t4692 = t8.*t4574;
t4696 = t16.*t4574;
t4699 = -t8.*(t260+t468+t570+t2298);
t4700 = -t9.*(t260+t468+t570+t2298);
t4702 = -t16.*(t260+t468+t570+t2298);
t4703 = -t17.*(t260+t468+t570+t2298);
t4727 = t8.*t4618;
t4728 = t9.*t4618;
t4729 = t16.*t4618;
t4730 = t17.*t4618;
t4731 = t9.*t3239.*(t348-t525).*(-1.0./2.0);
t4732 = t2646.*(-3.867742437e-3);
t4741 = -t4717;
t4747 = t2649.*(-1.563719772e-3);
t4748 = t16.*(t260+t468+t570+t2298);
t4749 = t2646.*3.867742437e-3;
t4754 = t3317.*(t348-t525).*(-1.0./4.0);
t4758 = t520.*2.454825983680473e-3;
t4768 = t3304.*(t348-t525).*(-1.0./4.0);
t4770 = t3307.*(t348-t525).*(-1.0./4.0);
t4773 = t2649.*1.563719772e-3;
t4783 = (t3317.*(t348-t525))./4.0;
t4787 = (t17.*(t348-t525).*(t689-t740))./2.0;
t4795 = -t4766;
t4796 = (t3304.*(t348-t525))./4.0;
t4797 = (t3307.*(t348-t525))./4.0;
t4825 = t3453.*(t348-t525).*(-1.0./4.0);
t4836 = t3441.*(t348-t525).*(-1.0./4.0);
t4838 = -t4823;
t4840 = (t3453.*(t348-t525))./4.0;
t4846 = (t3441.*(t348-t525))./4.0;
t4893 = -t4880;
t4932 = -t4918;
t4934 = -t4920;
t4940 = t2482.*(t689-t740).*(-1.0./4.0);
t4950 = (t2482.*(t689-t740))./4.0;
t4952 = -t4927;
t4983 = -t4973;
t4996 = -t4982;
t4997 = -t4984;
t5002 = t1961.*8.36241330891889e-4;
t5004 = t9.*(t348-t525).*(-8.36241330891889e-4);
t5005 = -t4989;
t5006 = -t4990;
t5008 = t3433.*3.867742437e-3;
t5010 = t1965.*2.74179553204116e-4;
t5014 = t17.*(t348-t525).*(-2.74179553204116e-4);
t5022 = t3428.*1.563719772e-3;
t5033 = t17.*(t348-t525).*2.74179553204116e-4;
t5038 = -t5019;
t5074 = t3686.*5.01208083475e-2;
t5086 = t3682.*1.17633784675e-2;
t5104 = -t5098;
t5132 = t9.*(t3682+t16.*(t295-t13.*t42.*(3.3e+1./4.0e+2))).*(-7.35522e-1);
t5138 = -t5117;
t5141 = -t5122;
t5178 = t4704.*(-7.35522e-1);
t5192 = t4704.*7.35522e-1;
t5203 = t8.*(t260+t468+t570+t2298).*(-7.35522e-1);
t5204 = t9.*(t260+t468+t570+t2298).*(-7.35522e-1);
t5208 = t17.*(t260+t468+t570+t2298).*(-7.35522e-1);
t5211 = t8.*(t260+t468+t570+t2298).*(-1.666555);
t5223 = -t5202;
t5235 = t1117+t4498;
t5261 = -t5251;
t5301 = t4410.*(t357-t519).*(-1.0./4.0);
t5311 = (t4410.*(t357-t519))./4.0;
t5313 = -t5303;
t5318 = t9.*t4410.*(t348-t525).*(-1.0./4.0);
t5330 = t4533.*(t348-t525);
t5336 = t4476.*(t348-t525).*(-1.0./4.0);
t5347 = (t4476.*(t348-t525))./4.0;
t5354 = -t5344;
t5361 = t4927.*7.35522e-1;
t5362 = t4928.*7.35522e-1;
t5366 = t4527.*(t348-t525).*(-1.0./4.0);
t5369 = t4532.*(t348-t525).*(-1.0./4.0);
t5375 = -t5364;
t5376 = t17.*t4515.*(t348-t525).*(-1.0./4.0);
t5379 = (t4527.*(t348-t525))./4.0;
t5381 = (t4532.*(t348-t525))./4.0;
t5390 = t4689.*(t348-t525);
t5403 = t4635.*(t348-t525).*(-1.0./4.0);
t5411 = (t4635.*(t348-t525))./4.0;
t5428 = -t5418;
t5431 = t4711.*(t348-t525).*(-1.0./4.0);
t5444 = (t4711.*(t348-t525))./4.0;
t5472 = t675+t1554+t1914+t2282;
t5493 = -t5474;
t5512 = (t2482.*t4515)./4.0;
t5546 = t1035+t1580+t2131+t2196;
t5547 = (t17.*t5481)./4.0;
t5554 = -t5534;
t5559 = -t5541;
t5590 = t9.*(t3682+t16.*(t295-t13.*t42.*(3.3e+1./4.0e+2))).*(-1.563719772e-3);
t5595 = t16.*t4498.*4.38178973375e-3;
t5602 = (t9.*t16.*t5481)./4.0;
t5647 = -t5627;
t5649 = t9.*(t260+t468+t570+t2298).*(-3.867742437e-3);
t5661 = t17.*(t260+t468+t570+t2298).*(-1.563719772e-3);
t5668 = t1586+t1614+t2285+t2291;
t5670 = -t5654;
t5671 = (t9.*t5553)./4.0;
t5679 = t531+t615+t786+t1238+t1975;
t5683 = -t5672;
t5694 = (t7.*t5586)./4.0;
t5695 = (t16.*t17.*t5553)./4.0;
t5702 = -t5689;
t5703 = -t5690;
t5708 = -t5697;
t5718 = (t14.*t15.*t5586)./4.0;
t5724 = -t5711;
t5735 = -t5726;
t5742 = -t5732;
t5744 = -t5733;
t5748 = (t325.*t5481)./4.0;
t5751 = -t5737;
t5756 = -t5743;
t5758 = -t5746;
t5760 = t503+t793+t1153+t1514+t2227;
t5769 = -t5753;
t5786 = (t229.*t5553)./4.0;
t5813 = t4928.*3.867742437e-3;
t5824 = t4927.*1.563719772e-3;
t5838 = t464+t555+t1881+t1981+t2288;
t5841 = (t321.*t5586)./2.0;
t5853 = t468+t570+t1835+t1984+t2298;
t5859 = (t440.*t5481)./2.0;
t5863 = -t5848;
t5864 = -t5851;
t5865 = -t5854;
t5867 = -t5855;
t5912 = t2756+t2881+t3162;
t5914 = t2763+t2984+t3061;
t5919 = t2758+t3010+t3062;
t5923 = t1574+t2092+t4505;
t5926 = -t5905;
t5947 = t1543+t2032+t4545;
t5952 = t1493+t1681+t1792+t3670;
t5961 = -t5941;
t6002 = t5553.*(t79-t358).*(-1.0./2.0);
t6010 = -t5993;
t6012 = -t5995;
t6014 = t1102+t1466+t2203+t3439;
t6016 = t361+t599+t767+t1198+t1612+t1668;
t6018 = -t6001;
t6019 = (t5553.*(t79-t358))./2.0;
t6028 = t8.*t5050.*4.38178973375e-3;
t6030 = t5312.*(t348-t525).*(-1.0./4.0);
t6032 = t5314.*(t348-t525).*(-1.0./4.0);
t6038 = t330+t771+t797+t1219+t1575+t1828;
t6045 = (t5312.*(t348-t525))./4.0;
t6048 = (t5314.*(t348-t525))./4.0;
t6062 = -t6047;
t6075 = t5586.*(t71-t391).*(-1.0./4.0);
t6096 = t143+t792+t1450+t1516+t1794+t1845;
t6097 = (t9.*t16.*t5955)./4.0;
t6158 = t142+t469+t1449+t1515+t2207+t2248;
t6173 = (t16.*t17.*t6041)./4.0;
t6177 = -t6157;
t6190 = t169+t299+t303+t1329+t1437+t2085+t2249;
t6228 = (t7.*t6143)./4.0;
t6252 = (t14.*t15.*t6143)./4.0;
t6255 = (t325.*t5955)./4.0;
t6268 = t5481.*(t395+t9.*(t48-t349)).*(-1.0./4.0);
t6270 = (t17.*t6188)./4.0;
t6275 = t2149+t2278+t2572+t2623;
t6281 = (t16.*t6211)./2.0;
t6285 = (t5481.*(t395+t9.*(t48-t349)))./4.0;
t6297 = (t8.*t6227)./2.0;
t6299 = (t9.*t16.*t6188)./4.0;
t6301 = t2182+t2317+t2576+t2655;
t6302 = t162+t688+t1470+t1546+t1989+t2099;
t6304 = t2750+t3480+t3597;
t6306 = (t229.*t6041)./4.0;
t6310 = t5532.*(t348-t525).*(-1.0./4.0);
t6321 = (t8.*t15.*t6211)./4.0;
t6325 = (t5532.*(t348-t525))./4.0;
t6327 = (t1907.*t5553)./4.0;
t6328 = (t15.*t16.*t6227)./4.0;
t6344 = -t6322;
t6355 = -t6339;
t6359 = t9.*t5345.*1.13264871585e-2;
t6364 = (t9.*t6276)./4.0;
t6374 = t5580.*(t348-t525).*(-1.0./4.0);
t6379 = t5582.*(t348-t525).*(-1.0./4.0);
t6386 = (t605.*t5763)./4.0;
t6392 = (t5580.*(t348-t525))./4.0;
t6399 = (t440.*t5955)./4.0;
t6400 = (t16.*t17.*t6276)./4.0;
t6406 = -t6393;
t6409 = -t6398;
t6418 = t5644.*(t348-t525).*(-1.0./4.0);
t6424 = (t321.*t6143)./4.0;
t6426 = (t5644.*(t348-t525))./4.0;
t6434 = (t227.*t6211)./4.0;
t6435 = t2525+t2532+t4545;
t6439 = (t325.*t6188)./4.0;
t6440 = -t6432;
t6446 = t4546+t4589;
t6448 = t14.*t6431;
t6450 = t15.*t6431;
t6451 = t6.*t6431;
t6453 = t7.*t6431;
t6456 = t6041.*(t79-t358).*(-1.0./4.0);
t6459 = (t323.*t6227)./4.0;
t6464 = (t6041.*(t79-t358))./4.0;
t6467 = -t6458;
t6470 = t6.*t6452;
t6471 = t6.*t6449;
t6478 = -t6452;
t6487 = (t229.*t6276)./4.0;
t6490 = t5763.*(t357-t519).*(-1.0./4.0);
t6498 = t6.*t6476;
t6500 = t6.*t6461;
t6502 = -t6472;
t6507 = -t6491;
t6516 = t6.*t6505;
t6521 = t9.*t5763.*(t348-t525).*(-1.0./4.0);
t6532 = t5835.*(t348-t525);
t6535 = t260+t468+t570+t2298+t2684+t2687;
t6537 = (t440.*t6188)./4.0;
t6543 = t6143.*(t71-t391).*(-1.0./2.0);
t6547 = (t6143.*(t71-t391))./2.0;
t6549 = (t439.*t6227)./4.0;
t6553 = t5821.*(t348-t525).*(-1.0./4.0);
t6555 = t6211.*(t48-t349).*(-1.0./4.0);
t6556 = -t6548;
t6562 = (t5821.*(t348-t525))./4.0;
t6564 = (t6211.*(t48-t349))./4.0;
t6565 = t17.*t5837.*(t348-t525).*(-1.0./4.0);
t6573 = t1915+t2082+t2086+t2274+t2330;
t6575 = t5903.*(t348-t525);
t6576 = t5875.*(t348-t525).*(-1.0./4.0);
t6582 = -t6574;
t6583 = (t5875.*(t348-t525))./4.0;
t6587 = t5879.*(t348-t525).*(-1.0./4.0);
t6588 = -t6579;
t6596 = -t6585;
t6601 = t6276.*(t79-t358).*(-1.0./4.0);
t6612 = (t6276.*(t79-t358))./4.0;
t6616 = -t6604;
t6619 = t2057+t2197+t2257+t2271+t2303;
t6628 = t5981.*(t348-t525).*(-1.0./4.0);
t6629 = t2013+t2120+t2239+t2324+t2356;
t6635 = (t348-t525).*(t1254+t1943+t9.*t439.*1.196e-3+t439.*t1083).*(-1.0./4.0);
t6636 = t667+t1190+t1607+t1725+t1940+t2273;
t6638 = t5955.*(t395+t9.*(t48-t349)).*(-1.0./2.0);
t6639 = (t5981.*(t348-t525))./4.0;
t6641 = t2098+t2104+t2208+t2342+t2371;
t6642 = t2045+t2145+t2311+t2328+t2338;
t6650 = (t5955.*(t395+t9.*(t48-t349)))./2.0;
t6654 = t1271+t1478+t2153+t2160+t3331;
t6657 = -t6645;
t6661 = -t6648;
t6666 = t6029.*(t348-t525).*(-1.0./4.0);
t6672 = (t2482.*t5837)./2.0;
t6674 = (t1907.*t6041)./2.0;
t6676 = (t6029.*(t348-t525))./4.0;
t6677 = t2435+t2880+t2891+t3043;
t6678 = -t6669;
t6683 = t1170+t1257+t1554+t1583+t2129+t2282;
t6689 = t8.*t6671;
t6700 = -t6686;
t6702 = (t15.*(t667+t1190-t1580+t1607-t1919+t2273))./4.0;
t6704 = t745+t1014+t1697+t1756+t2184+t2318;
t6705 = (t17.*t6637)./4.0;
t6706 = -t6690;
t6718 = -t6697;
t6729 = t553+t1954+t2161+t2276+t3686;
t6730 = (t16.*t6653)./4.0;
t6734 = (t7.*t14.*(t667+t1190-t1580+t1607-t1919+t2273))./4.0;
t6736 = (t9.*t16.*t6637)./4.0;
t6737 = -t6722;
t6741 = -t6728;
t6743 = t828+t1216+t1608+t1738+t2283+t2358;
t6747 = t6.*t15.*(t667+t1190-t1580+t1607-t1919+t2273).*(-1.0./4.0);
t6752 = t7.*(t495+t572+t1838+t2069+t2107).*(-1.059103943995e-1);
t6754 = (t8.*t15.*t6653)./4.0;
t6755 = -t6745;
t6756 = t988+t1424+t1597+t1780+t2140+t2382;
t6758 = t1276+t1503+t1618+t1633+t2260+t2306;
t6759 = -t6746;
t6760 = (t14.*t43.*(t667+t1190-t1580+t1607-t1919+t2273))./4.0;
t6764 = t7.*(t495+t572+t1838+t2069+t2107).*1.059103943995e-1;
t6765 = t7.*t16.*t6653.*(-1.0./4.0);
t6774 = (t15.*t44.*t6653)./2.0;
t6777 = t6.*t6746;
t6784 = t1349+t1582+t1685+t1861+t2110+t2381;
t6788 = -t6776;
t6789 = (t7.*t6709)./4.0;
t6791 = -t6778;
t6793 = (t16.*t6727)./4.0;
t6796 = t8.*t6773;
t6798 = (t8.*t6720)./4.0;
t6801 = t6452.*1.666555;
t6804 = t6449.*1.666555;
t6806 = t6452.*1.225946;
t6809 = t6449.*1.225946;
t6818 = (t14.*(t828+t1216-t1603+t1608-t2210+t2358))./4.0;
t6820 = -t6797;
t6825 = t6227.*(t348-t525).*(-1.0./2.0);
t6828 = t6188.*(t395+t9.*(t48-t349)).*(-1.0./2.0);
t6830 = -t6814;
t6831 = t6466.*7.35522e-1;
t6832 = -t6816;
t6833 = -t6817;
t6834 = t6472.*7.35522e-1;
t6837 = t6475.*3.587895;
t6838 = t6466.*1.666555;
t6840 = t6460.*3.587895;
t6841 = t6469.*1.666555;
t6843 = (t15.*t16.*t6720)./4.0;
t6847 = t6472.*1.666555;
t6848 = t6474.*1.666555;
t6851 = t6505.*(-1.666555);
t6852 = t6477.*1.666555;
t6854 = (t6227.*(t348-t525))./2.0;
t6857 = t6475.*1.225946;
t6858 = t6505.*(-1.225946);
t6859 = t6477.*1.225946;
t6862 = t6460.*1.225946;
t6864 = t6462.*1.225946;
t6866 = (t6188.*(t395+t9.*(t48-t349)))./2.0;
t6869 = (t8.*t15.*t6727)./4.0;
t6871 = (t6.*t13.*(t828+t1216-t1603+t1608-t2210+t2358))./4.0;
t6877 = t7.*t8.*t6720.*(-1.0./4.0);
t6881 = -t6842;
t6885 = t6505.*1.666555;
t6889 = t6505.*1.225946;
t6892 = t7.*t16.*t6727.*(-1.0./4.0);
t6894 = t5.*t14.*(t828+t1216-t1603+t1608-t2210+t2358).*(-1.0./4.0);
t6898 = (t15.*t39.*t6720)./4.0;
t6900 = t6517.*(-7.35522e-1);
t6902 = t6497.*1.666555;
t6906 = t6.*t6855;
t6907 = t6517.*(-1.666555);
t6908 = t6492.*1.225946;
t6911 = t6497.*1.225946;
t6912 = -t6886;
t6915 = t6.*t6863;
t6918 = (t15.*t44.*t6727)./4.0;
t6920 = (t225.*(t667+t1190-t1580+t1607-t1919+t2273))./4.0;
t6921 = (t226.*(t667+t1190-t1580+t1607-t1919+t2273))./4.0;
t6923 = t16.*t5951.*4.38178973375e-3;
t6927 = t6517.*7.35522e-1;
t6931 = (t227.*t6653)./2.0;
t6932 = (t228.*t6653)./2.0;
t6934 = t6517.*1.666555;
t6935 = (t4300.*t5345)./4.0;
t6936 = -t6909;
t6939 = (t1907.*t6276)./2.0;
t6948 = (t13.*t42.*(t828+t1216-t1603+t1608-t2210+t2358))./2.0;
t6949 = -t6924;
t6962 = (t15.*t223.*(t667+t1190-t1580+t1607-t1919+t2273))./2.0;
t6965 = ((t348-t525).*(-t2182+t2241+t696.*(t48-t349)+t891.*(t48-t349)))./4.0;
t6975 = -t6961;
t6982 = t499+t552+t921+t1317+t1880+t2072+t2114;
t6987 = -t6971;
t6988 = t478+t550+t1296+t1416+t1833+t1930+t2289;
t6991 = -t6972;
t6994 = -t6978;
t6998 = t223.*t6746;
t7009 = t16.*t321.*t6653.*(-1.0./4.0);
t7016 = -t6999;
t7018 = (t403.*(t667+t1190-t1580+t1607-t1919+t2273))./2.0;
t7019 = (t4964.*(t2904-t2927))./4.0;
t7020 = -t7004;
t7023 = (t8.*t6917)./4.0;
t7028 = (t404.*t6653)./4.0;
t7033 = (t227.*t6727)./4.0;
t7034 = (t228.*t6727)./4.0;
t7037 = t6475.*1.8732399795e-1;
t7039 = t495+t572+t1062+t1436+t1838+t2069+t2107;
t7042 = t6460.*9.5384188575e-2;
t7043 = -t7024;
t7044 = -t7025;
t7051 = (t321.*t6709)./2.0;
t7062 = (t323.*t6720)./4.0;
t7063 = (t324.*t6720)./4.0;
t7066 = t602+t896+t1269+t1701+t2269+t3348;
t7071 = t439.*t6671;
t7072 = (t319.*(t828+t1216-t1603+t1608-t2210+t2358))./2.0;
t7073 = (t320.*(t828+t1216-t1603+t1608-t2210+t2358))./2.0;
t7075 = -t7061;
t7080 = t2065+t2074+t2166+t2245+t3637;
t7083 = (t454.*(t667+t1190-t1580+t1607-t1919+t2273))./2.0;
t7084 = (t16.*t321.*t6727)./2.0;
t7085 = -t7070;
t7087 = (t440.*t6637)./2.0;
t7089 = (t370.*t6720)./2.0;
t7090 = (t8.*t321.*t6720)./2.0;
t7093 = (t8.*t7022)./4.0;
t7096 = (t16.*t7010)./4.0;
t7104 = (t404.*t6727)./2.0;
t7106 = (t470.*(t667+t1190-t1580+t1607-t1919+t2273))./2.0;
t7109 = t6653.*(t48-t349).*(-1.0./4.0);
t7112 = (t15.*t16.*t7022)./4.0;
t7118 = (t8.*t15.*t7010)./4.0;
t7122 = (t6653.*(t48-t349))./4.0;
t7127 = -t7119;
t7143 = -t7136;
t7144 = -t7138;
t7155 = t439.*t6773;
t7156 = (t439.*t6720)./2.0;
t7159 = (t539.*t6653)./2.0;
t7162 = -t7146;
t7164 = t16.*t6653.*(t71-t391).*(-1.0./4.0);
t7168 = (t323.*t6917)./4.0;
t7172 = t6727.*(t48-t349).*(-1.0./2.0);
t7174 = (t4255.*t5635)./2.0;
t7176 = (t483.*t6720)./2.0;
t7179 = t6709.*(t71-t391).*(-1.0./4.0);
t7180 = (t605.*t6615)./4.0;
t7181 = -t7175;
t7187 = t6727.*(t60-t394).*(-1.0./2.0);
t7188 = (t4286.*t5646)./2.0;
t7192 = (t227.*t7010)./2.0;
t7201 = t16.*t6727.*(t71-t391).*(-1.0./4.0);
t7203 = t8.*t6720.*(t71-t391).*(-1.0./4.0);
t7208 = (t539.*t6727)./4.0;
t7216 = (t604.*t6653)./4.0;
t7219 = (t323.*t7022)./2.0;
t7221 = -t7209;
t7224 = t5116+t5125;
t7225 = t6720.*(t113-t409).*(-1.0./4.0);
t7227 = t5107+t5119;
t7231 = t16.*t6681.*2.62925e-3;
t7239 = (t6720.*(t113-t409))./4.0;
t7251 = (t439.*t6917)./2.0;
t7259 = t5123+t5183;
t7280 = t6449.*2.5171736245e-2;
t7283 = t6452.*7.326866269e-3;
t7291 = (t604.*t6727)./4.0;
t7304 = t6466.*5.01208083475e-2;
t7310 = t6462.*2.5171736245e-2;
t7311 = t6472.*5.01208083475e-2;
t7314 = t6505.*(-7.326866269e-3);
t7315 = t6477.*7.326866269e-3;
t7318 = t6469.*1.17633784675e-2;
t7319 = -t7295;
t7321 = t6474.*1.17633784675e-2;
t7326 = -t7307;
t7330 = t5.*t6431.*2.01382560198e-1;
t7335 = t9.*t6780.*1.539925e-2;
t7338 = t6505.*7.326866269e-3;
t7339 = -t7316;
t7340 = t6720.*(t380-t392).*(-1.0./4.0);
t7342 = t6492.*2.5171736245e-2;
t7349 = (t439.*t7022)./4.0;
t7351 = t6517.*(-5.01208083475e-2);
t7355 = -t7332;
t7358 = t6497.*7.326866269e-3;
t7360 = -t7337;
t7364 = t9.*t6615.*(t348-t525).*(-1.0./4.0);
t7365 = (t6720.*(t380-t392))./4.0;
t7372 = t12.*t7332;
t7373 = t6517.*5.01208083475e-2;
t7379 = -t7363;
t7387 = -t7374;
t7390 = t7010.*(t48-t349).*(-1.0./4.0);
t7398 = t12.*t7374;
t7400 = t12.*t7376;
t7403 = (t7010.*(t48-t349))./4.0;
t7404 = t6637.*(t395+t9.*(t48-t349)).*(-1.0./4.0);
t7410 = t6653.*(t386+t16.*(t69-t347)).*(-1.0./4.0);
t7412 = t12.*t7388;
t7416 = (t6637.*(t395+t9.*(t48-t349)))./4.0;
t7421 = (t6653.*(t386+t16.*(t69-t347)))./4.0;
t7431 = t17.*t6526.*1.13264871585e-2;
t7433 = t1695+t2030+t2097+t2172+t2491+t2567;
t7441 = t9.*t6540.*1.13264871585e-2;
t7445 = (t1904.*t6720)./2.0;
t7448 = t17.*t6687.*(t348-t525).*(-1.0./4.0);
t7449 = t6720.*(t348-t525).*(-1.0./4.0);
t7461 = t6727.*(t386+t16.*(t69-t347)).*(-1.0./2.0);
t7470 = (t6727.*(t386+t16.*(t69-t347)))./2.0;
t7475 = t1641+t2067+t2225+t2265+t2604+t2629;
t7482 = t1390+t2058+t2222+t2348+t2584+t2637;
t7498 = (t16.*t7446)./4.0;
t7502 = -t7492;
t7505 = t8.*t7479;
t7515 = t8.*t7494;
t7530 = (t8.*t15.*t7446)./4.0;
t7536 = -t7524;
t7545 = t7.*t16.*t7446.*(-1.0./4.0);
t7553 = -t7535;
t7554 = t6917.*(t348-t525).*(-1.0./4.0);
t7555 = (t5583.*(t2821-t2864))./4.0;
t7561 = (t15.*t44.*t7446)./4.0;
t7569 = (t2482.*t6687)./4.0;
t7571 = (t6917.*(t348-t525))./4.0;
t7577 = -t7560;
t7581 = -t7567;
t7592 = (t8.*t7507)./4.0;
t7602 = -t7589;
t7612 = t2815+t3060+t3364+t4400;
t7613 = t2759+t3082+t3459+t4402;
t7622 = t2934+t3100+t3534+t4334;
t7626 = (t15.*t16.*t7507)./4.0;
t7630 = -t7614;
t7635 = -t7616;
t7638 = -t7621;
t7659 = t7022.*(t348-t525).*(-1.0./2.0);
t7660 = -t7641;
t7663 = -t7648;
t7664 = -t7649;
t7669 = (t227.*t7446)./4.0;
t7670 = (t228.*t7446)./4.0;
t7671 = (t536.*t7226)./4.0;
t7673 = (t7022.*(t348-t525))./2.0;
t7675 = -t7661;
t7677 = -t7645;
t7682 = -t7666;
t7686 = t536.*(t5122+t5.*(t2425-t2468).*3.587895).*(-1.0./4.0);
t7695 = -t7678;
t7698 = t323.*t7479;
t7707 = (t4509.*t6046)./4.0;
t7713 = (t4489.*t6069)./4.0;
t7716 = (t4498.*t6069)./4.0;
t7717 = t323.*t7494;
t7719 = (t554.*t7226)./4.0;
t7728 = -t7693;
t7737 = -t7718;
t7740 = t554.*(t5122+t5.*(t2425-t2468).*3.587895).*(-1.0./4.0);
t7741 = (t16.*t321.*t7446)./2.0;
t7753 = (t554.*(t5122+t5.*(t2425-t2468).*3.587895))./4.0;
t7761 = (t404.*t7446)./2.0;
t7763 = (t583.*t7226)./4.0;
t7771 = t1855+t2332+t2376+t2398+t2705+t2833;
t7778 = t583.*(t5122+t5.*(t2425-t2468).*3.587895).*(-1.0./4.0);
t7787 = (t323.*t7507)./4.0;
t7789 = (t583.*(t5122+t5.*(t2425-t2468).*3.587895))./4.0;
t7790 = t14.*t7247.*6.8635e-3;
t7792 = t13.*t7223.*6.23745e-2;
t7797 = t2926+t6780;
t7805 = t5.*t7236.*6.23745e-2;
t7808 = t13.*(t5117+t5.*(t2425-t2468).*3.228604).*(-6.23745e-2);
t7811 = -t7793;
t7823 = t13.*(t5117+t5.*(t2425-t2468).*3.228604).*6.23745e-2;
t7839 = t12.*t13.*t7223.*(-6.23745e-2);
t7855 = -t7844;
t7857 = (t5345.*t5448)./4.0;
t7858 = t7446.*(t48-t349).*(-1.0./2.0);
t7867 = -t7854;
t7868 = t1841+t2389+t2414+t2429+t2790+t2830;
t7874 = (t1490.*t7226)./4.0;
t7876 = (t1572.*t7226)./4.0;
t7879 = -t7864;
t7881 = -t7866;
t7882 = t3544+t3555+t3881+t3885;
t7883 = t7446.*(t60-t394).*(-1.0./2.0);
t7885 = t7.*t6967.*1.059103943995e-1;
t7891 = t1490.*(t5122+t5.*(t2425-t2468).*3.587895).*(-1.0./4.0);
t7892 = (t8.*t7800)./4.0;
t7895 = t1572.*(t5122+t5.*(t2425-t2468).*3.587895).*(-1.0./4.0);
t7896 = (t1572.*t7241)./4.0;
t7908 = (t1572.*(t5122+t5.*(t2425-t2468).*3.587895))./4.0;
t7914 = t16.*t7446.*(t71-t391).*(-1.0./4.0);
t7915 = (t439.*t7507)./2.0;
t7919 = (t15.*t16.*t7800)./4.0;
t7923 = (t539.*t7446)./4.0;
t7928 = -t7917;
t7929 = -t7918;
t7940 = t729+t2226+t2606+t3349+t4629;
t7942 = -t7926;
t7949 = t718+t2125+t2603+t3343+t4704;
t7951 = -t7939;
t7954 = (t1920.*t7226)./4.0;
t7965 = t1920.*(t5122+t5.*(t2425-t2468).*3.587895).*(-1.0./4.0);
t7974 = (t5331.*t5583)./4.0;
t7976 = (t1920.*(t5122+t5.*(t2425-t2468).*3.587895))./4.0;
t7977 = t605.*(t1528+t1966+t2026-t2172+t587.*(t48-t349)+t689.*(t48-t349)).*(-1.0./2.0);
t7995 = -t7985;
t7999 = -t7992;
t8001 = (t604.*t7446)./4.0;
t8005 = (t17.*t7932)./4.0;
t8030 = -t8011;
t8031 = -t8012;
t8037 = (t9.*t16.*t7932)./4.0;
t8039 = -t8023;
t8040 = -t8025;
t8052 = (t323.*t7800)./2.0;
t8065 = t2547+t2854+t3189+t3290+t3626;
t8066 = (t4255.*t6552)./4.0;
t8067 = (t6114.*(t2821-t2864))./4.0;
t8068 = -t8056;
t8070 = t2470+t3059+t3117+t3200+t3790;
t8075 = t2804+t3808+t3840+t4385;
t8079 = -t8060;
t8097 = -t8078;
t8100 = (t3738.*t6780)./4.0;
t8101 = t7642.*7.35522e-1;
t8102 = t7642.*1.666555;
t8106 = -t8088;
t8107 = t7645.*1.666555;
t8116 = -t8103;
t8126 = ((t357-t519).*(t1528+t1966+t2026-t2172+t587.*(t48-t349)+t689.*(t48-t349)))./2.0;
t8140 = -t8124;
t8141 = t4591+t6460;
t8143 = t7690.*7.35522e-1;
t8148 = t7690.*1.666555;
t8149 = t7693.*1.666555;
t8150 = (t9.*t8055)./4.0;
t8165 = t7494.*(t348-t525);
t8166 = t4664+t6475;
t8172 = -t8161;
t8176 = (t16.*t17.*t8055)./4.0;
t8177 = t4586+t6492;
t8184 = t7479.*(t348-t525);
t8189 = t8.*(t6460-t35.*(t2425-t2468));
t8191 = t130+t288+t2156+t2192+t2580+t2662+t4505;
t8192 = t16.*(t6460-t35.*(t2425-t2468));
t8194 = t7446.*(t386+t16.*(t69-t347)).*(-1.0./2.0);
t8195 = (t325.*t7932)./2.0;
t8197 = (t439.*t7800)./4.0;
t8208 = (t7446.*(t386+t16.*(t69-t347)))./2.0;
t8213 = t4655+t6497;
t8221 = t41.*(t6460-t35.*(t2425-t2468));
t8223 = (t2701.*t7226)./4.0;
t8224 = t45.*(t6460-t35.*(t2425-t2468));
t8240 = t2701.*(t5122+t5.*(t2425-t2468).*3.587895).*(-1.0./4.0);
t8248 = -t8235;
t8259 = t7507.*(t348-t525).*(-1.0./2.0);
t8274 = (t7507.*(t348-t525))./2.0;
t8283 = (t4843.*t6431)./4.0;
t8293 = -t8280;
t8294 = -t8282;
t8298 = -t8287;
t8301 = -t8291;
t8309 = (t229.*t8055)./2.0;
t8314 = -t8307;
t8316 = (t440.*t7932)./4.0;
t8320 = t17.*t7796.*1.539925e-2;
t8323 = (t5634.*t5635)./4.0;
t8330 = (t5628.*t5646)./4.0;
t8341 = (t4916.*t6431)./4.0;
t8342 = t16.*t7402.*4.38178973375e-3;
t8346 = -t8335;
t8347 = (t4922.*t6431)./4.0;
t8348 = -t8336;
t8351 = -t8340;
t8355 = -t8344;
t8357 = (t4936.*t6431)./4.0;
t8362 = -t8353;
t8366 = -t8356;
t8373 = -t8364;
t8377 = t8.*t7434.*4.38178973375e-3;
t8384 = -t8375;
t8387 = -t8380;
t8388 = -t8381;
t8389 = (t3350.*t7223)./4.0;
t8391 = (t3405.*t7223)./4.0;
t8392 = (t3356.*t7236)./4.0;
t8400 = (t3396.*t7223)./4.0;
t8401 = t3350.*(t5117+t5.*(t2425-t2468).*3.228604).*(-1.0./4.0);
t8402 = (t3350.*t7236)./4.0;
t8406 = t3405.*(t5117+t5.*(t2425-t2468).*3.228604).*(-1.0./4.0);
t8407 = (t3405.*t7236)./4.0;
t8410 = (t7245.*(t943-t1091))./4.0;
t8411 = -t8397;
t8414 = (t3350.*(t5117+t5.*(t2425-t2468).*3.228604))./4.0;
t8415 = t3396.*(t5117+t5.*(t2425-t2468).*3.228604).*(-1.0./4.0);
t8417 = (t3424.*t7245)./4.0;
t8418 = -t8404;
t8419 = (t3405.*(t5117+t5.*(t2425-t2468).*3.228604))./4.0;
t8421 = (t7246.*(t943-t1091))./4.0;
t8424 = (t3396.*(t5117+t5.*(t2425-t2468).*3.228604))./4.0;
t8427 = (t3424.*t7246)./4.0;
t8429 = (t5331.*t6114)./4.0;
t8433 = t428+t553+t2143+t2169+t3259+t3274+t3686;
t8434 = t8055.*(t79-t358).*(-1.0./4.0);
t8440 = (t8055.*(t79-t358))./4.0;
t8443 = t7.*(t2437+t2648+t3129+t3384+t3574).*(-8.639075e-2);
t8449 = t7.*(t2437+t2648+t3129+t3384+t3574).*8.639075e-2;
t8452 = (t3720.*t7226)./4.0;
t8458 = t7800.*(t348-t525).*(-1.0./2.0);
t8461 = (t7226.*(t85+t338+t362+t375+t408+t5.*t12.*(7.9e+1./2.5e+2)))./4.0;
t8462 = t3720.*(t5122+t5.*(t2425-t2468).*3.587895).*(-1.0./4.0);
t8467 = -t8457;
t8469 = (t7800.*(t348-t525))./2.0;
t8472 = (t5122+t5.*(t2425-t2468).*3.587895).*(t85+t338+t362+t375+t408+t5.*t12.*(7.9e+1./2.5e+2)).*(-1.0./4.0);
t8473 = (t7241.*(t85+t338+t362+t375+t408+t5.*t12.*(7.9e+1./2.5e+2)))./4.0;
t8487 = ((t5122+t5.*(t2425-t2468).*3.587895).*(t85+t338+t362+t375+t408+t5.*t12.*(7.9e+1./2.5e+2)))./4.0;
t8495 = (t2044.*t7796)./4.0;
t8496 = (t4900.*t6589)./4.0;
t8501 = t7642.*5.01208083475e-2;
t8507 = t7645.*1.17633784675e-2;
t8524 = (t4939.*t6589)./4.0;
t8528 = t7690.*5.01208083475e-2;
t8529 = t8.*t8062.*2.62925e-3;
t8542 = t7693.*1.17633784675e-2;
t8543 = t15.*t8050.*8.639075e-2;
t8547 = t969+t2409+t3069+t3078+t3481+t3598;
t8559 = t7.*t8054.*8.639075e-2;
t8575 = t7932.*(t395+t9.*(t48-t349)).*(-1.0./4.0);
t8598 = (t7932.*(t395+t9.*(t48-t349)))./4.0;
t8623 = (t348-t525).*(t2053+t2059-t2177+t2363+t3257+t3287).*(-1.0./2.0);
t8629 = ((t348-t525).*(t2053+t2059-t2177+t2363+t3257+t3287))./2.0;
t8633 = (t5345.*t6408)./2.0;
t8649 = (t1907.*t8055)./4.0;
t8667 = -t8661;
t8700 = (t4884.*t6970)./4.0;
t8711 = t763+t1225+t1260+t2997+t3137+t3422+t3583;
t8757 = (t5433.*t6526)./4.0;
t8764 = (t5434.*t6540)./4.0;
t8765 = (t5929.*t6069)./4.0;
t8766 = t6175.*(t495+t572+t1838+t2069+t2107).*(-1.0./4.0);
t8778 = (t6175.*(t495+t572+t1838+t2069+t2107))./4.0;
t8796 = (t4611.*t7247)./4.0;
t8837 = t15.*(t6460-t35.*(t2425-t2468)).*7.326866269e-3;
t8839 = (t2966.*t8050)./4.0;
t8844 = t14.*(t6460-t35.*(t2425-t2468)).*2.46255173325e-2;
t8846 = t7.*(t6460-t35.*(t2425-t2468)).*2.5171736245e-2;
t8852 = (t3763.*t7796)./4.0;
t8853 = (t2980.*t8054)./4.0;
t8868 = -t8849;
t8873 = (t5928.*t6175)./4.0;
t8884 = (t5442.*t6589)./4.0;
t8888 = (t7130.*(t2904-t2927))./4.0;
t8937 = (t5999.*t6196)./4.0;
t8956 = -t8946;
t8960 = t7.*t8931;
t8963 = t15.*t8931;
t8966 = -t8954;
t8970 = (t5329.*t6780)./2.0;
t8976 = (t5634.*t6552)./2.0;
t8983 = (t5345.*t6781)./2.0;
t8996 = t3421.*(t2752+t3814-t4385-t9.*t439.*3.127439544e-3).*(-1.0./4.0);
t9019 = -t9015;
t9032 = -t9027;
t9041 = (t5443.*t6970)./4.0;
t9043 = t4255.*(t2437+t2648+t3129+t3384+t3574).*(-1.0./4.0);
t9045 = (t4035.*t8050)./4.0;
t9046 = (t4474.*t7796)./2.0;
t9047 = (t4255.*(t2437+t2648+t3129+t3384+t3574))./4.0;
t9059 = (t4064.*t8054)./4.0;
t9068 = (t5365.*t7130)./4.0;
t9071 = -t9065;
t9093 = (t4255.*t8044)./4.0;
t9098 = t2773+t2935+t3099+t3156+t3594+t4335;
t9100 = -t9091;
t9104 = t2586+t3476+t3487+t3540+t3561+t3585;
t9113 = -t9105;
t9123 = (t4798.*t7796)./2.0;
t9142 = t8998.*(-1.666555);
t9147 = t8998.*1.666555;
t9151 = t15.*t3249.*(t6460-t35.*(t2425-t2468)).*4.1663875e-1;
t9165 = t8.*t9156;
t9166 = t16.*t9156;
t9177 = -t9169;
t9178 = -t9170;
t9195 = t14.*t8697.*2.46255173325e-2;
t9209 = t2459+t2590+t2817+t3066+t3114+t3313+t3578;
t9217 = t2440+t2601+t2810+t2988+t3187+t3391+t3577;
t9233 = t1791+t1818+t2335+t2387+t2789+t3887+t4928;
t9236 = t2437+t2648+t2851+t3129+t3136+t3384+t3574;
t9260 = (t6385.*t6589)./4.0;
t9261 = (t4849.*t8050)./2.0;
t9262 = (t4837.*t8054)./2.0;
t9269 = t3148+t3202+t3206+t3234+t3646+t4609;
t9276 = -t9271;
t9277 = (t5345.*t7540)./2.0;
t9280 = t9.*t9048.*1.539925e-2;
t9282 = t17.*t9049.*1.539925e-2;
t9286 = -t9279;
t9297 = (t5713.*t7245)./4.0;
t9298 = t9091.*1.666555;
t9300 = t9090.*1.225946;
t9301 = t9091.*1.225946;
t9302 = (t8689.*(t943-t1091))./4.0;
t9310 = t1605+t2464+t3212+t3216+t3644+t3685+t3785;
t9312 = (t5213.*t7796)./2.0;
t9313 = (t3424.*t8689)./4.0;
t9325 = t5456+t7512;
t9333 = t1137+t1657+t2448+t2499+t3047+t3101+t3530+t3571;
t9336 = t5476+t7520;
t9337 = t5467+t7513;
t9348 = (t4879.*(t6460-t35.*(t2425-t2468)))./4.0;
t9366 = t6.*t8931.*2.46255173325e-2;
t9367 = -t9350;
t9369 = (t15.*t4884.*(t6460-t35.*(t2425-t2468)))./4.0;
t9381 = (t6175.*t6967)./4.0;
t9389 = t7.*t4255.*(t6460-t35.*(t2425-t2468)).*3.064865e-1;
t9391 = (t4917.*(t6460-t35.*(t2425-t2468)))./4.0;
t9402 = ((t6460-t35.*(t2425-t2468)).*(t2812-t2860))./4.0;
t9406 = ((t6460-t35.*(t2425-t2468)).*(t2821-t2864))./4.0;
t9414 = t8998.*(-1.17633784675e-2);
t9415 = t15.*t4286.*(t6460-t35.*(t2425-t2468)).*3.064865e-1;
t9432 = t8998.*1.17633784675e-2;
t9436 = (t6431.*t6713)./4.0;
t9446 = (t5064.*t8050)./2.0;
t9448 = -t9435;
t9455 = -t9439;
t9478 = -t9465;
t9481 = (t5095.*t8054)./2.0;
t9508 = -t9500;
t9511 = -t9502;
t9521 = t2113+t9090;
t9529 = (t5137.*(t6460-t35.*(t2425-t2468)))./4.0;
t9591 = (t6216.*t7223)./4.0;
t9593 = (t6205.*t7236)./4.0;
t9594 = t9090.*2.5171736245e-2;
t9597 = (t6069.*t7402)./4.0;
t9599 = t9091.*7.326866269e-3;
t9601 = t6216.*(t5117+t5.*(t2425-t2468).*3.228604).*(-1.0./4.0);
t9608 = (t6216.*(t5117+t5.*(t2425-t2468).*3.228604))./4.0;
t9615 = (t6046.*t7434)./4.0;
t9626 = (t5331.*(t6460-t35.*(t2425-t2468)))./4.0;
t9627 = -t9618;
t9646 = (t4964.*t8477)./4.0;
t9657 = (t6353.*t7226)./4.0;
t9660 = (t6589.*t6969)./4.0;
t9661 = t14.*(t5454-t7513).*(-6.8635e-3);
t9666 = t6353.*(t5122+t5.*(t2425-t2468).*3.587895).*(-1.0./4.0);
t9669 = t14.*(t5454-t7513).*6.8635e-3;
t9676 = t5634.*(t2437+t2648+t3129+t3384+t3574).*(-1.0./4.0);
t9682 = (t5634.*(t2437+t2648+t3129+t3384+t3574))./4.0;
t9700 = -t9693;
t9704 = (t5613.*t8050)./2.0;
t9710 = (t5634.*t8044)./4.0;
t9715 = (t8628.*(t2904-t2927))./4.0;
t9731 = (t3738.*t9048)./4.0;
t9734 = (t5648.*t8054)./2.0;
t9735 = (t3743.*t9049)./4.0;
t9773 = t5696.*(t2752+t3814-t4385-t9.*t439.*3.127439544e-3).*(-1.0./4.0);
t9786 = -t9774;
t9791 = (t6431.*t7422)./4.0;
t9798 = -t9785;
t9807 = -t9792;
t9828 = t367+t9685;
t9829 = -t9817;
t9831 = (t6589.*t7217)./2.0;
t9838 = -t9825;
t9860 = (t5806.*t8050)./4.0;
t9862 = (t5740.*(t6460-t35.*(t2425-t2468)))./4.0;
t9873 = (t5750.*(t6460-t35.*(t2425-t2468)))./4.0;
t9875 = -t9864;
t9876 = (t5755.*(t6460-t35.*(t2425-t2468)))./4.0;
t9877 = -t9.*(t258+t2289+t5392+t7559);
t9879 = -t17.*(t258+t2289+t5392+t7559);
t9883 = t8050.*(t495+t572+t1838+t2069+t2107).*(-1.0./4.0);
t9884 = t1958+t2077+t9086;
t9891 = t8.*t9855;
t9892 = t16.*t9855;
t9894 = (t8050.*(t495+t572+t1838+t2069+t2107))./4.0;
t9902 = (t5860.*t8054)./4.0;
t9910 = (t5928.*t8050)./4.0;
t9911 = (t5826.*(t6460-t35.*(t2425-t2468)))./4.0;
t9917 = (t3270.*t9263)./4.0;
t9924 = (t3265.*t9278)./4.0;
t9925 = (t5999.*t8054)./4.0;
t9933 = (t5583.*t8437)./4.0;
t9935 = (t3360.*t9278)./4.0;
t9936 = (t5365.*t8628)./4.0;
t9950 = -t9944;
t9951 = t3270.*(t5454-t7513).*(-1.0./4.0);
t9957 = (t3270.*(t5454-t7513))./4.0;
t9971 = (t943-t1091).*(t5457-t7520).*(-1.0./4.0);
t9974 = ((t943-t1091).*(t5457-t7520))./4.0;
t9975 = t3424.*(t5457-t7520).*(-1.0./4.0);
t9983 = (t3424.*(t5457-t7520))./4.0;
t9988 = (t6092.*(t6460-t35.*(t2425-t2468)))./4.0;
t9993 = t15.*t5628.*(t6460-t35.*(t2425-t2468)).*3.064865e-1;
t9994 = t7.*t5634.*(t6460-t35.*(t2425-t2468)).*3.064865e-1;
t9996 = (t3771.*t9278)./4.0;
t10033 = (t6589.*t7676)./4.0;
t10040 = t15.*t5699.*(t6460-t35.*(t2425-t2468)).*4.1663875e-1;
t10049 = (t7.*t6175.*(t6460-t35.*(t2425-t2468)))./4.0;
t10055 = (t6222.*(t6460-t35.*(t2425-t2468)))./4.0;
t10060 = (t15.*t6196.*(t6460-t35.*(t2425-t2468)))./4.0;
t10064 = (t6431.*t7952)./4.0;
t10070 = (t7108.*t7236)./4.0;
t10078 = t9.*(t258+t2289+t5392+t7559).*(-7.35522e-1);
t10079 = t17.*(t258+t2289+t5392+t7559).*(-7.35522e-1);
t10084 = t7223.*(t5026+t5.*(t2959-t2967)).*(-1.0./4.0);
t10087 = -t10072;
t10089 = t7226.*(t5026+t5.*(t2959-t2967)).*(-1.0./4.0);
t10094 = t1850+t1871+t2805+t2956+t5503+t5729;
t10097 = (t7223.*(t5026+t5.*(t2959-t2967)))./4.0;
t10098 = ((t5026+t5.*(t2959-t2967)).*(t5117+t5.*(t2425-t2468).*3.228604))./4.0;
t10099 = -t10085;
t10102 = (t7226.*(t5026+t5.*(t2959-t2967)))./4.0;
t10103 = ((t5026+t5.*(t2959-t2967)).*(t5122+t5.*(t2425-t2468).*3.587895))./4.0;
t10105 = (t3249.*t9525)./4.0;
t10107 = -t10093;
t10141 = t1175+t1729+t2749+t3469+t3472+t3889+t3912+t4389;
t10142 = (t6460-t35.*(t2425-t2468)).*(t985+t3399-t13.*t42.*1.01140545e-1-t7.*t223.*5.034347249e-2).*(-1.0./4.0);
t10150 = t6.*t9685.*2.46255173325e-2;
t10155 = (t3752.*t9525)./4.0;
t10166 = -t10157;
t10168 = (t4453.*t9278)./4.0;
t10215 = (t4611.*t9263)./4.0;
t10219 = (t6589.*(t917-t1669+t2469+t2475+t3495+t3591))./2.0;
t10269 = t14.*t9830.*2.46255173325e-2;
t10280 = t9.*(t258+t2289+t5392+t7559).*(-3.867742437e-3);
t10284 = t17.*(t258+t2289+t5392+t7559).*(-1.563719772e-3);
t10285 = t9.*(t258+t2289+t5392+t7559).*3.867742437e-3;
t10292 = t17.*(t258+t2289+t5392+t7559).*1.563719772e-3;
t10304 = -t10302;
t10320 = -t10313;
t10327 = (t5750.*t8931)./4.0;
t10331 = (t7236.*t7620)./4.0;
t10339 = (t7223.*t7656)./4.0;
t10340 = (t6750.*(t6460-t35.*(t2425-t2468)))./4.0;
t10349 = t7656.*(t5117+t5.*(t2425-t2468).*3.228604).*(-1.0./4.0);
t10350 = (t6763.*(t6460-t35.*(t2425-t2468)))./4.0;
t10353 = (t6767.*(t6460-t35.*(t2425-t2468)))./4.0;
t10356 = (t7656.*(t5117+t5.*(t2425-t2468).*3.228604))./4.0;
t10373 = (t7226.*t7734)./4.0;
t10392 = t7734.*(t5122+t5.*(t2425-t2468).*3.587895).*(-1.0./4.0);
t10401 = (t7734.*(t5122+t5.*(t2425-t2468).*3.587895))./4.0;
t10404 = -t10397;
t10422 = (t6928.*(t6460-t35.*(t2425-t2468)))./4.0;
t10425 = -t10416;
t10441 = t1070+t1648+t1929+t2287+t9091;
t10444 = -t10437;
t10461 = -t10453;
t10477 = t15.*t6589.*(t6460-t35.*(t2425-t2468)).*4.1663875e-1;
t10478 = (t9499.*(t2821-t2864))./4.0;
t10492 = (t5275.*t9278)./4.0;
t10496 = (t6589.*(t2433+t2449-t3048-t3102+t3223+t3232))./2.0;
t10500 = -t10498;
t10501 = t169+t299+t1329+t1437+t2085+t2249+t5079+t7305;
t10512 = (t6431.*t8728)./4.0;
t10524 = (t5331.*t9285)./4.0;
t10527 = -t10519;
t10547 = (t7223.*t8156)./4.0;
t10551 = (t7245.*(t6460-t35.*(t2425-t2468)))./4.0;
t10557 = t8156.*(t5117+t5.*(t2425-t2468).*3.228604).*(-1.0./4.0);
t10558 = (t7236.*t8156)./4.0;
t10567 = t9.*t10542;
t10569 = t17.*t10542;
t10571 = (t8156.*(t5117+t5.*(t2425-t2468).*3.228604))./4.0;
t10574 = t7223.*(-t3405+t4994+t5076).*(-1.0./4.0);
t10582 = (t7223.*(-t3405+t4994+t5076))./4.0;
t10583 = ((t5117+t5.*(t2425-t2468).*3.228604).*(-t3405+t4994+t5076))./4.0;
t10584 = t7236.*(-t3405+t4994+t5076).*(-1.0./4.0);
t10626 = (t5518.*t9278)./2.0;
t10633 = (t5523.*t9278)./2.0;
t10634 = (t7226.*t8297)./4.0;
t10647 = (t5543.*t9278)./4.0;
t10649 = t8297.*(t5122+t5.*(t2425-t2468).*3.587895).*(-1.0./4.0);
t10650 = (t7241.*t8297)./4.0;
t10670 = (t8297.*(t5122+t5.*(t2425-t2468).*3.587895))./4.0;
t10686 = (t5331.*t9499)./4.0;
t10704 = -t10695;
t10709 = -t10701;
t10740 = (t6767.*t8697)./4.0;
t10766 = t5713.*(t5457-t7520).*(-1.0./4.0);
t10768 = (t5713.*(t5457-t7520))./4.0;
t10769 = t758+t1253+t2990+t3133+t3149+t3244+t7715;
t10807 = -t10802;
t10820 = t1053+t3327+t3449+t5479+t7749;
t10825 = (t5115.*t9830)./4.0;
t10849 = (t9278.*(-t1272-t1479+t1647+t1848+t2236))./2.0;
t10850 = t1125+t1305+t1877+t1932+t2299+t5393+t7527;
t10858 = t1296+t1416+t1833+t1930+t2289+t5392+t7559;
t10859 = -t10854;
t10874 = -t10870;
t10881 = (t3421.*t10398)./4.0;
t10884 = (t3489.*t10398)./4.0;
t10887 = (t7.*t8050.*(t6460-t35.*(t2425-t2468)))./4.0;
t10893 = (t6431.*t9218)./4.0;
t10897 = (t15.*t8054.*(t6460-t35.*(t2425-t2468)))./4.0;
t10899 = -t10892;
t10903 = -t10898;
t10909 = (t6431.*(t2720-t8734))./4.0;
t10912 = t6.*t10754.*6.8635e-3;
t10914 = -t10905;
t10916 = -t10908;
t10922 = t14.*t10759.*6.8635e-3;
t10964 = t1895+t10759;
t10966 = t1902+t10754;
t10978 = (t5750.*t9685)./4.0;
t10992 = (t15.*t8256.*(t6460-t35.*(t2425-t2468)))./4.0;
t11001 = -t10993;
t11023 = t757+t1252+t2989+t3132+t3366+t3400+t5495+t5725;
t11075 = (t5739.*t9830)./4.0;
t11077 = (t8438.*(t6460-t35.*(t2425-t2468)))./4.0;
t11080 = (t8437.*(t6460-t35.*(t2425-t2468)))./4.0;
t11116 = (t5843.*t9830)./4.0;
t11155 = (t8609.*(t6460-t35.*(t2425-t2468)))./4.0;
t11167 = -t11154;
t11184 = (t3275.*t10754)./4.0;
t11191 = (t3270.*t10759)./4.0;
t11206 = (t6589.*t9525)./4.0;
t11213 = (t6970.*t9278)./4.0;
t11244 = (t8689.*(t6460-t35.*(t2425-t2468)))./4.0;
t11266 = t258+t2075+t2167+t2289+t2614+t2620+t5392+t7559;
t11269 = (t6223.*t9830)./4.0;
t11288 = -t11279;
t11381 = (t8477.*t8628)./4.0;
t11458 = (t6750.*t9685)./4.0;
t11463 = (t4557.*t10754)./4.0;
t11474 = (t4611.*t10759)./4.0;
t11476 = -t11473;
t11523 = (t6762.*t9830)./4.0;
t11526 = t6.*t6430.*t9830.*8.9697375e-1;
t11539 = t6.*t9830.*(t4540+t5.*(t2425-t2468)).*(-8.9697375e-1);
t11568 = (t5696.*t10398)./4.0;
t11626 = t266+t2288+t7399+t9102;
t11633 = t260+t2298+t7401+t9119;
t11650 = t7.*t11228.*1.059103943995e-1;
t11667 = t9.*t11651;
t11668 = t17.*t11651;
t11676 = t15.*t11247.*1.059103943995e-1;
t11685 = -t11683;
t11709 = (t6431.*t10201)./4.0;
t11712 = -t11708;
t11720 = t1646+t1770+t2312+t2370+t10542;
t11731 = -t11722;
t11732 = (t9263.*(t6460-t35.*(t2425-t2468)))./4.0;
t11767 = (t15.*t9278.*(t6460-t35.*(t2425-t2468)))./4.0;
t11791 = (t6460-t35.*(t2425-t2468)).*(t5457-t7520).*(-1.0./4.0);
t11793 = (t6460-t35.*(t2425-t2468)).*(t5454-t7513).*(-1.0./4.0);
t11801 = ((t6460-t35.*(t2425-t2468)).*(t5457-t7520))./4.0;
t11803 = ((t6460-t35.*(t2425-t2468)).*(t5454-t7513))./4.0;
t11809 = (t7320.*t9830)./4.0;
t11848 = t11671.*(-1.666555);
t11854 = t11671.*(-7.35522e-1);
t11855 = t11672.*(-7.35522e-1);
t11859 = -t11851;
t11862 = t11671.*7.35522e-1;
t11864 = t11672.*7.35522e-1;
t11870 = t8.*t11852;
t11893 = (t8437.*t9285)./4.0;
t11907 = t763+t1260+t2997+t3137+t3422+t3583+t5496+t7750;
t11997 = t11671.*(-5.01208083475e-2);
t12002 = t11671.*5.01208083475e-2;
t12013 = t8.*t11672.*(-3.867742437e-3);
t12049 = t1881+t1981+t2288+t7399+t9102;
t12053 = t1835+t1984+t2298+t7401+t9119;
t12163 = t2546+t2996+t2999+t3115+t7751+t7959;
t12379 = t15.*t12185.*8.639075e-2;
t12385 = t921+t1317+t1880+t2072+t2114+t7424+t9099;
t12388 = t1457+t2144+t2671+t11653;
t12392 = t1492+t2158+t2696+t11651;
t12396 = t1062+t1436+t1838+t2069+t2107+t7423+t9121;
t12397 = -t9.*(t7645+t8.*(-t244+t7279+t15.*(t257+t269)+t7.*(t263-t7252)));
t12398 = -t17.*(t7645+t8.*(-t244+t7279+t15.*(t257+t269)+t7.*(t263-t7252)));
t12407 = t17.*(t7645+t8.*(-t244+t7279+t15.*(t257+t269)+t7.*(t263-t7252)));
t12485 = t9.*(t7645+t8.*(-t244+t7279+t15.*(t257+t269)+t7.*(t263-t7252))).*(-7.35522e-1);
t12533 = t9830.*(t1786+t2973-t7703-t5.*t12.*3.746479959e-1).*(-1.0./2.0);
t12538 = (t9830.*(t1786+t2973-t7703-t5.*t12.*3.746479959e-1))./2.0;
t12553 = (t10759.*(t6460-t35.*(t2425-t2468)))./4.0;
t12578 = t9.*(t7645+t8.*(-t244+t7279+t15.*(t257+t269)+t7.*(t263-t7252))).*(-1.563719772e-3);
t12600 = (t6460-t35.*(t2425-t2468)).*(-t1053-t3327+t5081.*1.225946+t7731+t15.*t223.*1.4653732538e-2).*(-1.0./4.0);
t12690 = t17.*t12563.*1.539925e-2;
t12746 = t7.*(t3129+t3384+t3574+t7846+t9332).*(-8.639075e-2);
t12753 = t7.*(t3129+t3384+t3574+t7846+t9332).*8.639075e-2;
t12792 = t3063+t3528+t3966+t11846;
t12869 = (t8050.*t11228)./4.0;
t12882 = (t8054.*t11247)./4.0;
t12891 = (t5628.*t12185)./4.0;
t12911 = (t3743.*t12563)./4.0;
t12915 = (t9830.*(-t1785+t2869+t2960+t5489+t5720+t4.*t13.*3.746479959e-1))./2.0;
t13002 = (t3249.*t12669)./4.0;
t13019 = t1268+t1760+t1807+t2373+t7642+t10568;
t13025 = t4255.*(t3129+t3384+t3574+t7846+t9332).*(-1.0./4.0);
t13032 = (t4255.*(t3129+t3384+t3574+t7846+t9332))./4.0;
t13052 = (t3752.*t12669)./4.0;
t13134 = t2810+t2988+t3187+t3391+t3577+t7848+t9322;
t13140 = t2851+t3129+t3136+t3384+t3574+t7846+t9332;
t13162 = t6069.*(t1292+t2073+t2694+t11671).*(-1.0./4.0);
t13164 = (t6069.*(t1292+t2073+t2694+t11671))./4.0;
t13171 = t4021.*(t3116+t3486+t3963+t11671.*1.666555).*(-1.0./4.0);
t13173 = (t4021.*(t3116+t3486+t3963+t11671.*1.666555))./4.0;
t13190 = (t5345.*t12563)./4.0;
t13242 = (t9830.*t10754)./2.0;
t13285 = t5634.*(t3129+t3384+t3574+t7846+t9332).*(-1.0./4.0);
t13290 = (t5634.*(t3129+t3384+t3574+t7846+t9332))./4.0;
t13313 = t233+t359+t2395+t2401+t2837+t2894+t7642+t10568;
t13582 = t7796.*(t9.*(t16.*(t30.*(t2425-t2468)+t68.*(t2425-t2468))+t8.*(t7.*(t4650+t34.*(t2425-t2468))+t47.*(t2425-t2468)))+t17.*(t4654+t15.*(t4650+t34.*(t2425-t2468)))).*(-1.0./4.0);
t13607 = (t6589.*t12669)./4.0;
t1912 = t9.*t1840;
t1918 = t17.*t1840;
t2405 = t430+t579;
t2431 = t436+t581;
t2497 = -t9.*(t426-t581);
t2500 = -t17.*(t426-t581);
t2510 = -t2492;
t2549 = t9.*(t426-t581);
t2554 = -t2518;
t2592 = -t2537;
t2596 = -t2539;
t2602 = -t2543;
t2619 = -t2559;
t2634 = -t2566;
t2638 = -t2574;
t2639 = -t2579;
t2643 = -t2593;
t2659 = -t2613;
t2666 = -t2627;
t2692 = -t2668;
t2962 = -t2862;
t2971 = -t2866;
t3324 = t485+t2096;
t3334 = t587.*t1840;
t3337 = t589.*t1840;
t3465 = t775.*t1840;
t3466 = t2043.*7.35522e-1;
t3473 = t784.*t1840;
t3474 = t2049.*7.35522e-1;
t3483 = t798.*t1840;
t3490 = t687.*t1840;
t3492 = t689.*t1840;
t3497 = t693.*t1840;
t3499 = t696.*t1840;
t3505 = t701.*t1840;
t3515 = t740.*t1840;
t3520 = t751.*t1840;
t3587 = t891.*t1840;
t3589 = t906.*t1840;
t3634 = -t3580;
t3636 = -t3582;
t3846 = t17.*(t426-t581).*(-7.35522e-1);
t3898 = -t3848;
t3899 = -t3849;
t3908 = -t3871;
t3913 = -t3878;
t3917 = -t3888;
t3923 = -t3897;
t4133 = -t4099;
t4149 = -t4116;
t4160 = -t4125;
t4378 = -t4358;
t4381 = -t4360;
t4384 = -t4362;
t4407 = t2043.*3.867742437e-3;
t4411 = -t4382;
t4426 = -t4398;
t4429 = t2049.*1.563719772e-3;
t4479 = -t4459;
t4502 = t754.*(t689-t740).*(-1.0./4.0);
t4511 = t556+t3723;
t4519 = (t754.*(t689-t740))./4.0;
t4522 = t3735.*7.35522e-1;
t4524 = t3739.*7.35522e-1;
t4528 = t9.*t4493;
t4529 = t17.*t4493;
t4630 = -t4565;
t4672 = t17.*(t426-t581).*(-7.735484874e-3);
t4682 = (t1840.*t3296)./4.0;
t4687 = t1837.*(t689-t740).*(-1.0./4.0);
t4688 = -t4648;
t4693 = t9.*t4575;
t4695 = (t1840.*t3286)./2.0;
t4697 = t17.*t4575;
t4743 = -t4692;
t4744 = (t1840.*t3329)./4.0;
t4767 = t9.*t4727;
t4771 = t17.*t4727;
t4808 = (t1840.*t3524)./4.0;
t4947 = (t2612.*t3239)./4.0;
t4962 = t2522.*(t689-t740).*(-1.0./4.0);
t5023 = -t5002;
t5030 = -t5010;
t5042 = -t5022;
t5099 = -t5086;
t5106 = t3739.*3.867742437e-3;
t5128 = t4565.*7.35522e-1;
t5130 = t4566.*7.35522e-1;
t5135 = t4605.*(-7.35522e-1);
t5140 = t3735.*1.563719772e-3;
t5156 = t4605.*7.35522e-1;
t5160 = (t3239.*t3284)./4.0;
t5198 = t4696.*7.35522e-1;
t5205 = t4692.*1.666555;
t5207 = t4748.*(-7.35522e-1);
t5209 = t4696.*1.666555;
t5215 = t4748.*(-1.666555);
t5224 = t4728.*7.35522e-1;
t5227 = t4729.*7.35522e-1;
t5228 = t4730.*7.35522e-1;
t5230 = t4727.*1.666555;
t5232 = t4729.*1.666555;
t5234 = t909+t4514;
t5315 = (t1840.*t4477)./4.0;
t5332 = (t1837.*t4515)./4.0;
t5337 = t1540+t4699;
t5338 = (t1840.*t4534)./4.0;
t5342 = (t1840.*t4526)./4.0;
t5352 = t1777+t4692;
t5357 = t1510+t4748;
t5371 = -t5361;
t5409 = (t1840.*t4726)./4.0;
t5505 = (t2612.*t4410)./2.0;
t5519 = -t5512;
t5528 = (t2522.*t4515)./2.0;
t5549 = (t7.*t5472)./4.0;
t5568 = t4566.*3.867742437e-3;
t5574 = t4605.*(-3.867742437e-3);
t5584 = (t14.*t15.*t5472)./4.0;
t5585 = t4565.*1.563719772e-3;
t5596 = t4605.*3.867742437e-3;
t5617 = -t5595;
t5618 = t8.*t4514.*4.38178973375e-3;
t5621 = -t5602;
t5651 = t4696.*5.01208083475e-2;
t5662 = (t15.*t5546)./4.0;
t5666 = t4729.*5.01208083475e-2;
t5673 = t4692.*1.17633784675e-2;
t5675 = t4727.*1.17633784675e-2;
t5682 = -t5671;
t5686 = (t7.*t14.*t5546)./4.0;
t5706 = -t5694;
t5707 = -t5695;
t5717 = (t3284.*t4410)./4.0;
t5719 = t532+t617+t1108+t1392+t1978;
t5728 = -t5718;
t5738 = (t6.*t5668)./4.0;
t5754 = (t321.*t5472)./4.0;
t5764 = -t5748;
t5768 = (t13.*t14.*t5668)./4.0;
t5782 = t505+t1084+t1123+t1434+t2233;
t5792 = (t225.*t5546)./4.0;
t5797 = -t5786;
t5844 = -t5824;
t5858 = -t5841;
t5869 = -t5859;
t5871 = (t223.*t5668)./2.0;
t5909 = t5472.*(t71-t391).*(-1.0./2.0);
t5915 = t2824+t2890+t3044;
t5932 = (t5472.*(t71-t391))./2.0;
t5994 = (t470.*t5546)./2.0;
t6031 = (t1840.*t5334)./4.0;
t6193 = t1956+t2083+t2557+t2626;
t6206 = t16.*t5235.*4.38178973375e-3;
t6241 = -t6228;
t6250 = t1971+t2258+t2534+t2668;
t6263 = -t6252;
t6271 = t2070+t2178+t2615+t2689;
t6288 = -t6270;
t6316 = -t6299;
t6323 = -t6306;
t6342 = -t6321;
t6346 = -t6327;
t6347 = -t6328;
t6370 = (t1840.*t5640)./4.0;
t6375 = (t1840.*t5625)./4.0;
t6376 = -t6359;
t6382 = -t6364;
t6403 = -t6386;
t6412 = -t6399;
t6414 = -t6400;
t6429 = -t6424;
t6443 = -t6434;
t6457 = (t754.*t5837)./4.0;
t6468 = -t6459;
t6489 = t16.*t5914.*2.62925e-3;
t6494 = -t6487;
t6499 = -t6470;
t6528 = (t1840.*t5810)./4.0;
t6536 = (t1837.*t5837)./4.0;
t6544 = -t6537;
t6550 = (t1840.*t5866)./4.0;
t6557 = -t6549;
t6559 = (t1840.*t5877)./4.0;
t6595 = t9.*t5679.*1.13264871585e-2;
t6630 = (t17.*t6573)./4.0;
t6634 = t2027+t2130+t2134+t2329+t2423;
t6652 = (t2612.*t5763)./4.0;
t6660 = (t1840.*t6064)./4.0;
t6680 = (t7.*t6619)./2.0;
t6682 = -t6674;
t6691 = (t9.*t6629)./4.0;
t6692 = (t2522.*t5837)./4.0;
t6701 = (t14.*t15.*t6619)./4.0;
t6708 = (t8.*t6641)./4.0;
t6714 = (t16.*t6642)./4.0;
t6723 = -t6702;
t6724 = -t6705;
t6733 = t6.*t6702;
t6738 = (t15.*t16.*t6641)./2.0;
t6739 = (t8.*t15.*t6642)./2.0;
t6742 = -t6730;
t6748 = -t6734;
t6753 = t7.*t6730;
t6757 = (t7.*t6683)./4.0;
t6761 = t1134+t1702+t5679;
t6766 = -t6754;
t6768 = t15.*t5853.*1.059103943995e-1;
t6770 = -t6760;
t6771 = (t1840.*t6211)./2.0;
t6779 = (t14.*t15.*t6683)./4.0;
t6783 = -t6774;
t6785 = (t8.*t6704)./4.0;
t6786 = (t325.*t6573)./4.0;
t6794 = t6451.*3.587895;
t6795 = t6448.*3.587895;
t6802 = t6453.*1.666555;
t6805 = t6451.*1.225946;
t6807 = t6453.*1.225946;
t6808 = t6448.*1.225946;
t6810 = t6450.*1.225946;
t6813 = t6.*t7.*t6683.*(-1.0./4.0);
t6815 = -t6793;
t6824 = -t6801;
t6826 = -t6806;
t6829 = (t14.*t37.*t6683)./4.0;
t6835 = -t6818;
t6836 = t7.*t6798;
t6844 = t2025+t2563+t3434+t3622;
t6846 = t6471.*1.666555;
t6853 = t6470.*1.225946;
t6856 = t6471.*1.225946;
t6865 = (t3284.*t5763)./4.0;
t6868 = t7.*t6793;
t6870 = t5.*t6818;
t6872 = t2895+t5914;
t6874 = (t229.*t6629)./4.0;
t6876 = -t6834;
t6880 = (t16.*t6756)./4.0;
t6882 = (t9.*t6758)./4.0;
t6883 = -t6847;
t6888 = t8.*t5923.*4.38178973375e-3;
t6893 = t1947+t2516+t3621+t3706;
t6895 = -t6871;
t6896 = t8.*t5952.*4.38178973375e-3;
t6905 = (t227.*t6642)./4.0;
t6913 = t6516.*(-1.225946);
t6916 = t16.*t5947.*4.38178973375e-3;
t6922 = (t321.*t6619)./4.0;
t6926 = (t8.*t15.*t6756)./4.0;
t6929 = (t16.*t17.*t6758)./4.0;
t6937 = t6516.*1.225946;
t6942 = -t6918;
t6943 = (t8.*t6784)./4.0;
t6945 = -t6920;
t6946 = -t6921;
t6953 = (t323.*t6641)./4.0;
t6956 = -t6935;
t6957 = t1804+t2031+t2569+t4702;
t6958 = -t6939;
t6959 = t9.*t6016.*1.13264871585e-2;
t6976 = -t6962;
t6977 = (t15.*t16.*t6784)./4.0;
t6979 = t17.*t6038.*1.13264871585e-2;
t6986 = (t440.*t6573)./4.0;
t6995 = t1292+t2073+t2694+t4729;
t6997 = t321.*t6730;
t7000 = t6451.*1.8732399795e-1;
t7003 = t2066+t2652+t3668+t3676;
t7005 = t6448.*9.5384188575e-2;
t7012 = (t7.*t223.*t6683)./2.0;
t7014 = (t321.*t6683)./4.0;
t7015 = (t322.*t6683)./4.0;
t7030 = t1673+t2252+t2675+t4727;
t7038 = -t7018;
t7040 = -t7019;
t7047 = -t7028;
t7049 = (t323.*t6704)./2.0;
t7050 = (t369.*t6683)./2.0;
t7052 = -t7033;
t7053 = -t7034;
t7055 = -t7037;
t7057 = -t7042;
t7076 = -t7062;
t7077 = -t7063;
t7079 = t885+t1440+t5923;
t7088 = -t7072;
t7091 = (t439.*t6641)./4.0;
t7094 = -t7083;
t7097 = -t7089;
t7099 = -t7090;
t7100 = t6629.*(t79-t358).*(-1.0./4.0);
t7102 = t6642.*(t48-t349).*(-1.0./4.0);
t7105 = t1103+t1465+t1511+t2277+t4493;
t7107 = t6619.*(t71-t391).*(-1.0./2.0);
t7110 = (t6642.*(t48-t349))./4.0;
t7116 = t1310+t1477+t5947;
t7117 = -t7104;
t7120 = -t7106;
t7121 = (t6619.*(t71-t391))./2.0;
t7126 = -t7118;
t7142 = t6683.*(t69-t347).*(-1.0./2.0);
t7147 = (t439.*t6704)./4.0;
t7152 = (t6683.*(t69-t347))./2.0;
t7165 = t6683.*(t71-t391).*(-1.0./2.0);
t7171 = t6730.*(t71-t391);
t7173 = (t6683.*(t71-t391))./2.0;
t7177 = -t7168;
t7182 = -t7176;
t7194 = (t439.*t6784)./2.0;
t7196 = t6756.*(t48-t349).*(-1.0./2.0);
t7197 = t6758.*(t79-t358).*(-1.0./2.0);
t7205 = (t6758.*(t79-t358))./2.0;
t7211 = t6793.*(t71-t391);
t7214 = t6798.*(t71-t391);
t7222 = t8.*t6677.*2.62925e-3;
t7230 = -t7216;
t7235 = t5121+t5138;
t7240 = t5105+t5141;
t7244 = -t7231;
t7264 = -t7251;
t7281 = t6450.*2.5171736245e-2;
t7282 = t6573.*(t395+t9.*(t48-t349)).*(-1.0./2.0);
t7284 = t6453.*7.326866269e-3;
t7286 = (t754.*t6687)./4.0;
t7290 = -t7280;
t7292 = -t7283;
t7298 = (t5083.*t5235)./4.0;
t7300 = t6470.*2.5171736245e-2;
t7312 = -t7291;
t7313 = t6471.*7.326866269e-3;
t7324 = (t1840.*t6642)./2.0;
t7325 = (t4021.*t5914)./4.0;
t7329 = -t7311;
t7331 = (t4024.*t5912)./4.0;
t7334 = (t4021.*t5919)./4.0;
t7336 = t140+t235+t1994+t2019+t2369+t2380+t3347;
t7341 = (t1907.*t6629)./2.0;
t7343 = -t7321;
t7345 = t6516.*(-2.5171736245e-2);
t7346 = (t1840.*t6653)./4.0;
t7348 = t831+t1717+t2018+t2496+t4566;
t7352 = -t7330;
t7357 = -t7335;
t7366 = -t7342;
t7367 = t6641.*(t348-t525).*(-1.0./2.0);
t7369 = t6516.*2.5171736245e-2;
t7371 = t12.*t7330;
t7377 = -t7358;
t7380 = (t6641.*(t348-t525))./2.0;
t7396 = t1497+t1938+t2005+t2275+t2505+t2630;
t7419 = (t3421.*t6304)./4.0;
t7432 = (t1840.*t6727)./4.0;
t7435 = t6704.*(t348-t525).*(-1.0./4.0);
t7439 = -t7431;
t7442 = (t6704.*(t348-t525))./4.0;
t7447 = -t7441;
t7456 = (t1840.*t6756)./4.0;
t7458 = t1233+t2047+t2194+t2234+t2589+t2640;
t7469 = t1754+t2051+t2089+t2240+t2599+t2625;
t7473 = (t1907.*t6758)./4.0;
t7485 = t2575+t2607+t2654+t2760+t2783;
t7487 = t6784.*(t348-t525).*(-1.0./4.0);
t7491 = t17.*(t578.*1.2516e-2+t2492-t2628+t2673+t1129.*(t71-t391)).*(-1.0./4.0);
t7499 = (t6784.*(t348-t525))./4.0;
t7501 = (t17.*(t578.*1.2516e-2+t2492-t2628+t2673+t1129.*(t71-t391)))./4.0;
t7509 = -t7498;
t7511 = t9.*t16.*(t578.*1.2516e-2+t2492-t2628+t2673+t1129.*(t71-t391)).*(-1.0./2.0);
t7514 = (t2612.*t6615)./4.0;
t7529 = t7.*t7498;
t7557 = (t17.*t7475)./4.0;
t7574 = -t7555;
t7576 = t9.*(t578.*4.28e-4+t2566-t2597+t905.*(t71-t391)+t1021.*(t71-t391)).*(-1.0./4.0);
t7578 = -t7561;
t7584 = -t7569;
t7587 = (t9.*t16.*t7475)./4.0;
t7598 = (t2522.*t6687)./4.0;
t7600 = t8.*t17.*t7475.*(-1.0./4.0);
t7603 = t16.*t17.*(t578.*4.28e-4+t2566-t2597+t905.*(t71-t391)+t1021.*(t71-t391)).*(-1.0./2.0);
t7605 = -t7592;
t7618 = (t16.*t45.*t7475)./4.0;
t7627 = (t1840.*t7010)./2.0;
t7644 = -t7626;
t7646 = t2878+t3035+t3463+t4351;
t7679 = t325.*(t578.*1.2516e-2+t2492-t2628+t2673+t1129.*(t71-t391)).*(-1.0./4.0);
t7684 = -t7669;
t7685 = -t7670;
t7696 = (t325.*(t578.*1.2516e-2+t2492-t2628+t2673+t1129.*(t71-t391)))./4.0;
t7701 = (t5235.*t5441)./4.0;
t7702 = t16.*t6729.*4.38178973375e-3;
t7724 = -t7707;
t7727 = -t7713;
t7729 = (t4514.*t6046)./4.0;
t7739 = -t7719;
t7747 = (t3284.*t6615)./4.0;
t7752 = t229.*(t578.*4.28e-4+t2566-t2597+t905.*(t71-t391)+t1021.*(t71-t391)).*(-1.0./4.0);
t7758 = (t325.*t7475)./4.0;
t7759 = (t326.*t7475)./4.0;
t7760 = (t229.*(t578.*4.28e-4+t2566-t2597+t905.*(t71-t391)+t1021.*(t71-t391)))./4.0;
t7774 = -t7761;
t7777 = -t7763;
t7786 = t475+t2056+t2203+t2351+t3433+t3503;
t7791 = t5.*t7224.*6.23745e-2;
t7794 = (t371.*t7475)./4.0;
t7798 = t17.*t323.*t7475.*(-1.0./4.0);
t7799 = t476+t1973+t2154+t2357+t3508+t3560;
t7801 = -t7787;
t7803 = t6.*t7259.*6.8635e-3;
t7804 = -t7790;
t7807 = -t7792;
t7815 = t3388+t3456+t3874+t3894;
t7819 = t440.*(t578.*1.2516e-2+t2492-t2628+t2673+t1129.*(t71-t391)).*(-1.0./4.0);
t7820 = t12.*t7792;
t7821 = -t7805;
t7828 = t2504+t2742+t2865+t3016+t3340;
t7837 = t12.*t7805;
t7838 = (t440.*(t578.*1.2516e-2+t2492-t2628+t2673+t1129.*(t71-t391)))./4.0;
t7840 = t12.*t7808;
t7851 = t12.*t7823;
t7859 = t16.*(-t1540+t2091+t2579+t8.*(t260+t468+t570+t2298)).*(-4.38178973375e-3);
t7869 = -t7857;
t7871 = t16.*(-t1540+t2091+t2579+t8.*(t260+t468+t570+t2298)).*4.38178973375e-3;
t7875 = t2075+t2167+t2614+t2620+t4575;
t7877 = (t1572.*t7227)./4.0;
t7894 = -t7876;
t7900 = (t440.*t7475)./4.0;
t7901 = t2488+t2867+t2915+t3077+t3501;
t7905 = t15.*(t921+t1317-t5853).*1.059103943995e-1;
t7909 = -t7896;
t7910 = t15.*t6988.*1.059103943995e-1;
t7920 = (t17.*t439.*t7475)./2.0;
t7922 = (t484.*t7475)./4.0;
t7924 = t7498.*(t71-t391);
t7935 = t2417+t2605+t3188+t3333+t3627;
t7936 = ((t79-t358).*(t578.*4.28e-4+t2566-t2597+t905.*(t71-t391)+t1021.*(t71-t391)))./4.0;
t7937 = t2419+t2645+t3125+t3336+t3630;
t7947 = t7.*t7039.*1.059103943995e-1;
t7964 = -t7954;
t7982 = t562+t1512+t1621+t1857+t2284+t2428+t3739;
t7984 = t16.*t7066.*4.38178973375e-3;
t7987 = t582+t1611+t1654+t1764+t2353+t2374+t3735;
t7988 = -t7974;
t7990 = t7475.*(t106-t414).*(-1.0./2.0);
t8018 = -t8001;
t8021 = -t8005;
t8049 = -t8037;
t8059 = (t4879.*t6190)./4.0;
t8077 = t4544+t6451;
t8080 = (t754.*t7475)./2.0;
t8083 = -t8066;
t8087 = -t8067;
t8113 = t4592+t6448;
t8115 = (t6158.*(t2904-t2927))./4.0;
t8117 = -t8107;
t8121 = (t4917.*t6190)./4.0;
t8134 = (t1840.*t7446)./4.0;
t8136 = (t6190.*(t2812-t2860))./4.0;
t8158 = -t8.*(t4542-t6448);
t8160 = -t16.*(t4542-t6448);
t8164 = -t8150;
t8170 = t8.*t7613.*2.62925e-3;
t8173 = t16.*t7612.*2.62925e-3;
t8178 = t1267+t1461+t1955+t2202+t2562+t4696;
t8180 = (t5235.*t5912)./2.0;
t8181 = ((t395+t9.*(t48-t349)).*(t578.*1.2516e-2+t2492-t2628+t2673+t1129.*(t71-t391)))./4.0;
t8183 = (t5434.*t5679)./4.0;
t8187 = -t41.*(t4542-t6448);
t8188 = -t45.*(t4542-t6448);
t8196 = -t8176;
t8203 = (t1837.*t7475)./2.0;
t8209 = -t8195;
t8214 = (t4896.*t6302)./4.0;
t8218 = t7.*t8189;
t8219 = t7.*t8192;
t8220 = t7.*t16.*(t4542-t6448);
t8222 = t41.*(t4542-t6448);
t8225 = t7.*t8166;
t8226 = t8.*t8166;
t8229 = t15.*t8166;
t8230 = t16.*t8166;
t8237 = t8.*t8177;
t8238 = t16.*t8177;
t8241 = t1907.*(t578.*4.28e-4+t2566-t2597+t905.*(t71-t391)+t1021.*(t71-t391)).*(-1.0./4.0);
t8255 = -t8221;
t8257 = (t1907.*(t578.*4.28e-4+t2566-t2597+t905.*(t71-t391)+t1021.*(t71-t391)))./4.0;
t8263 = (t4938.*t6302)./4.0;
t8264 = (t1840.*(-t1595+t2118+t2146+t2339+t16.*(t69-t347).*1.09e-4-t768.*(t69-t347)))./2.0;
t8266 = t9.*t8213;
t8268 = t17.*t7475.*(t348-t525).*(-1.0./4.0);
t8270 = t17.*t8213;
t8271 = t7475.*(t395+t9.*(t48-t349)).*(-1.0./2.0);
t8275 = (t6302.*(t2889-t2921))./4.0;
t8290 = (t5433.*t5760)./4.0;
t8295 = -t8283;
t8318 = -t8309;
t8319 = t9.*t7797.*1.539925e-2;
t8324 = -t8316;
t8326 = -t8320;
t8328 = -t8323;
t8338 = -t8330;
t8345 = (t2418.*t7475)./4.0;
t8352 = -t8341;
t8359 = t2612.*(t1528+t1966+t2026-t2172+t587.*(t48-t349)+t689.*(t48-t349)).*(-1.0./4.0);
t8369 = (t2612.*(t1528+t1966+t2026-t2172+t587.*(t48-t349)+t689.*(t48-t349)))./4.0;
t8376 = (t2482.*t7475)./4.0;
t8383 = (t3356.*t7224)./4.0;
t8390 = (t3350.*t7224)./4.0;
t8393 = (t3405.*t7224)./4.0;
t8396 = (t2522.*t7475)./4.0;
t8399 = -t8389;
t8405 = -t8391;
t8413 = -t8400;
t8416 = -t8402;
t8420 = -t8407;
t8422 = -t8410;
t8425 = -t8417;
t8426 = -t8421;
t8439 = (t5365.*t6096)./4.0;
t8460 = t1868+t2754+t2850+t3007+t3164+t3180;
t8463 = (t7227.*(t85+t338+t362+t375+t408+t5.*t12.*(7.9e+1./2.5e+2)))./4.0;
t8464 = t1812+t2803+t2853+t3012+t3094+t3224;
t8471 = -t8461;
t8476 = (t5365.*t6158)./4.0;
t8483 = (t2054.*t7797)./4.0;
t8488 = -t8473;
t8494 = t3284.*(t1528+t1966+t2026-t2172+t587.*(t48-t349)+t689.*(t48-t349)).*(-1.0./2.0);
t8497 = t970+t2796+t3070+t3079+t3217+t3233;
t8504 = (t3284.*(t1528+t1966+t2026-t2172+t587.*(t48-t349)+t689.*(t48-t349)))./2.0;
t8506 = t2181+t2444+t2560+t2632+t3429+t3616;
t8510 = -t8501;
t8520 = -t8507;
t8532 = t8.*(t4542-t6448).*(-7.35522e-1);
t8533 = t16.*(t4542-t6448).*(-7.35522e-1);
t8536 = t16.*t8070.*2.62925e-3;
t8538 = t8.*(t4542-t6448).*(-1.666555);
t8539 = t16.*(t4542-t6448).*(-1.666555);
t8544 = -t8528;
t8545 = -t8529;
t8549 = -t8542;
t8551 = -t8543;
t8552 = t2060+t2507+t2552+t2553+t3613+t3701;
t8555 = t45.*(t4542-t6448).*(-7.35522e-1);
t8557 = t8189.*7.35522e-1;
t8560 = t8192.*7.35522e-1;
t8564 = t8189.*1.666555;
t8566 = t8192.*1.666555;
t8567 = (t4884.*t6654)./4.0;
t8570 = -t8559;
t8583 = t8221.*7.35522e-1;
t8585 = t8224.*7.35522e-1;
t8615 = t2368+t2528+t2538+t2653+t3607+t3635;
t8636 = t17.*(t2056+t2203+t2351+t3433+t3503+t16.*t389.*(1.1e+1./1.25e+2)).*1.13264871585e-2;
t8640 = t981+t2807+t3087+t3090+t3420+t3426;
t8652 = (t9.*(t1961.*4.28e-4+t1965.*1.0027e-2-t2314+t2528+t2538-t905.*(t69-t347)))./4.0;
t8657 = -t8649;
t8664 = (t16.*t17.*(t1961.*4.28e-4+t1965.*1.0027e-2-t2314+t2528+t2538-t905.*(t69-t347)))./4.0;
t8693 = t206+t446+t2571+t2622+t2736+t2770+t4729;
t8696 = t17.*t7940.*1.13264871585e-2;
t8702 = t9.*t7949.*1.13264871585e-2;
t8709 = t2583+t3386+t3523+t3548+t4461;
t8712 = (t229.*(t1961.*4.28e-4+t1965.*1.0027e-2-t2314+t2528+t2538-t905.*(t69-t347)))./4.0;
t8738 = (t5235.*t6677)./2.0;
t8744 = (t5696.*t6304)./4.0;
t8748 = (t4884.*t7080)./4.0;
t8760 = (t5923.*t6046)./4.0;
t8772 = (t5947.*t6069)./4.0;
t8773 = (t5443.*t6535)./4.0;
t8775 = -t8765;
t8779 = t5153+t6862;
t8780 = t5169+t6840;
t8782 = (t4557.*t7259)./4.0;
t8791 = t1315+t2413+t2641+t3619+t3932+t3973;
t8792 = t5179+t6857;
t8794 = t5187+t6837;
t8800 = (t5853.*t6196)./4.0;
t8802 = t5152+t6908;
t8804 = t15.*(t4542-t6448).*(-7.326866269e-3);
t8805 = (t6014.*t6046)./4.0;
t8806 = t14.*(t4542-t6448).*(-2.46255173325e-2);
t8808 = t7.*(t4542-t6448).*(-2.5171736245e-2);
t8810 = -t8796;
t8812 = t8.*(t4542-t6448).*(-5.01208083475e-2);
t8816 = (t4024.*t7613)./4.0;
t8817 = t5177+t6911;
t8820 = t15.*(t4542-t6448).*7.326866269e-3;
t8821 = (t4021.*t7622)./4.0;
t8826 = t14.*(t4542-t6448).*2.46255173325e-2;
t8828 = t16.*(t4542-t6448).*(-1.17633784675e-2);
t8829 = t7.*(t4542-t6448).*2.5171736245e-2;
t8830 = t5172+t6902;
t8831 = (t4021.*t7612)./4.0;
t8833 = (t3767.*t7797)./4.0;
t8840 = (t79-t358).*(t1961.*4.28e-4+t1965.*1.0027e-2-t2314+t2528+t2538-t905.*(t69-t347)).*(-1.0./4.0);
t8850 = t8189.*5.01208083475e-2;
t8856 = -t8837;
t8857 = t7.*t8.*(t4542-t6448).*(-1.17633784675e-2);
t8858 = ((t79-t358).*(t1961.*4.28e-4+t1965.*1.0027e-2-t2314+t2528+t2538-t905.*(t69-t347)))./4.0;
t8861 = -t8844;
t8862 = t45.*(t4542-t6448).*(-1.563719772e-3);
t8864 = t8192.*1.17633784675e-2;
t8865 = -t8846;
t8872 = -t8852;
t8878 = t6.*t8166.*2.46255173325e-2;
t8883 = t45.*(t4542-t6448).*1.563719772e-3;
t8886 = t8221.*3.867742437e-3;
t8896 = -t8873;
t8906 = t7.*t8177.*1.059103943995e-1;
t8907 = t8224.*1.563719772e-3;
t8908 = -t8884;
t8925 = t15.*t8213.*1.059103943995e-1;
t8929 = t16.*(-t3218+t3458+t3878+t8.*(t260+t468+t570+t2298).*1.666555).*(-2.62925e-3);
t8938 = t16.*(-t3218+t3458+t3878+t8.*(t260+t468+t570+t2298).*1.666555).*2.62925e-3;
t8941 = t16.*(-t1476-t1540+t2091+t2165+t2579+t8.*(t260+t468+t570+t2298)).*(-4.38178973375e-3);
t8945 = -t8937;
t8947 = t16.*(-t1476-t1540+t2091+t2165+t2579+t8.*(t260+t468+t570+t2298)).*4.38178973375e-3;
t8949 = (t5216.*(t921+t1317-t5853))./4.0;
t8967 = (t5443.*t6654)./4.0;
t8979 = t1447+t1993+t7940;
t8981 = t1543+t2032+t7949;
t8984 = -t8963;
t8988 = -t8976;
t8989 = (t5218.*t7039)./4.0;
t8991 = (t6092.*t6190)./4.0;
t8992 = -t8983;
t9018 = (t6104.*t6302)./4.0;
t9024 = (t1907.*(t1961.*4.28e-4+t1965.*1.0027e-2-t2314+t2528+t2538-t905.*(t69-t347)))./2.0;
t9028 = t3201+t4401+t4424+t5203;
t9053 = -t9045;
t9062 = (t4517.*t7797)./2.0;
t9064 = -t9059;
t9069 = t6190.*(t985+t3399-t13.*t42.*1.01140545e-1-t7.*t223.*5.034347249e-2).*(-1.0./2.0);
t9075 = (t6302.*t6304)./2.0;
t9076 = -t9068;
t9079 = (t6190.*(t985+t3399-t13.*t42.*1.01140545e-1-t7.*t223.*5.034347249e-2))./2.0;
t9096 = -t9093;
t9106 = t2776+t2879+t3034+t3041+t3549+t4352;
t9110 = t2930+t3177+t7613;
t9112 = t2977+t3046+t7612;
t9115 = (t4772.*t7797)./2.0;
t9117 = (t5635.*(t921+t1317-t5853))./4.0;
t9118 = t15.*(t5150-t6911).*(-8.639075e-2);
t9120 = (t4286.*t8065)./4.0;
t9125 = t8963.*1.666555;
t9127 = t8960.*1.225946;
t9128 = t8963.*1.225946;
t9138 = t15.*t3249.*(t4542-t6448).*(-4.1663875e-1);
t9145 = t15.*t3249.*(t4542-t6448).*4.1663875e-1;
t9149 = (t5646.*t7039)./4.0;
t9158 = -t9151;
t9172 = -t9165;
t9174 = -t9166;
t9183 = (t3421.*t8547)./4.0;
t9187 = t2049+t2112+t2138+t2147+t3245+t3728+t4554;
t9189 = (t3489.*t8547)./4.0;
t9196 = t232+t429+t1461+t2506+t2524+t3657+t3669+t4696;
t9197 = t2043+t2168+t2188+t2223+t3242+t3724+t4605;
t9200 = -t9195;
t9212 = t6453+t6500;
t9213 = t6471+t6477;
t9216 = t2438+t2594+t2957+t3123+t3130+t3291+t3628;
t9219 = t5434.*(t1468-t1988-t2498+t4565+t17.*(t208-t427)).*(-1.0./4.0);
t9225 = t6450+t6516;
t9231 = (t5235.*t7613)./4.0;
t9252 = t1763+t1824+t2316+t2415+t2791+t3890+t4952;
t9272 = -t9261;
t9281 = t14.*t6190.*t6430.*3.064865e-1;
t9284 = t6069.*(-t1540+t2091+t2579+t8.*(t260+t468+t570+t2298)).*(-1.0./4.0);
t9287 = -t9280;
t9289 = -t9282;
t9291 = (t6069.*(-t1540+t2091+t2579+t8.*(t260+t468+t570+t2298)))./4.0;
t9294 = (t3266.*t8711)./4.0;
t9296 = t14.*t6190.*(t4540+t5.*(t2425-t2468)).*(-3.064865e-1);
t9307 = t14.*t6190.*(t4540+t5.*(t2425-t2468)).*3.064865e-1;
t9308 = -t9297;
t9309 = -t9298;
t9311 = -t9302;
t9314 = (t5217.*t7797)./2.0;
t9321 = t4021.*(-t3218+t3458+t3878+t8.*(t260+t468+t570+t2298).*1.666555).*(-1.0./4.0);
t9326 = t6046.*(t1492+t2158+t2696-t4727).*(-1.0./4.0);
t9330 = (t4021.*(-t3218+t3458+t3878+t8.*(t260+t468+t570+t2298).*1.666555))./4.0;
t9335 = t4879.*(t4542-t6448).*(-1.0./4.0);
t9338 = (t3362.*t8711)./4.0;
t9341 = (t8711.*(t923-t1076))./4.0;
t9343 = t15.*t4884.*(t4542-t6448).*(-1.0./4.0);
t9352 = (t6190.*t6928)./4.0;
t9354 = (t15.*t4884.*(t4542-t6448))./4.0;
t9360 = t7.*t4255.*(t4542-t6448).*(-3.064865e-1);
t9361 = t2923+t3443+t3900+t4327+t5192;
t9362 = t2928+t3500+t3852+t4330+t5176;
t9363 = t4917.*(t4542-t6448).*(-1.0./4.0);
t9364 = t8963.*7.326866269e-3;
t9368 = t8960.*2.5171736245e-2;
t9373 = (t6069.*t7066)./4.0;
t9374 = t7.*t4255.*(t4542-t6448).*3.064865e-1;
t9375 = (t2812-t2860).*(t4542-t6448).*(-1.0./4.0);
t9376 = (t4917.*(t4542-t6448))./4.0;
t9377 = (t2821-t2864).*(t4542-t6448).*(-1.0./4.0);
t9379 = -t9366;
t9382 = t15.*t4286.*(t4542-t6448).*(-3.064865e-1);
t9386 = -t9369;
t9390 = ((t2821-t2864).*(t4542-t6448))./4.0;
t9392 = t16.*t9098.*2.62925e-3;
t9394 = -t9381;
t9401 = -t9389;
t9404 = (t4896.*t8191)./4.0;
t9405 = -t9391;
t9408 = (t6196.*t6988)./4.0;
t9411 = (t4884.*t8213)./4.0;
t9425 = -t9406;
t9440 = t3249.*(t5144-t6902).*(-1.0./4.0);
t9444 = (t8166.*(t2821-t2864))./4.0;
t9449 = -t9436;
t9453 = (t4938.*t8191)./4.0;
t9454 = t9165.*7.35522e-1;
t9456 = (t3249.*(t5144-t6902))./4.0;
t9457 = t9166.*7.35522e-1;
t9458 = t9165.*1.666555;
t9459 = t9166.*1.666555;
t9463 = -t9446;
t9466 = (t8191.*(t2889-t2921))./4.0;
t9492 = (t6302.*t6966)./4.0;
t9505 = t967+t1568+t3369+t3374+t3649+t3688+t4328;
t9518 = t5137.*(t4542-t6448).*(-1.0./4.0);
t9524 = (t5137.*(t4542-t6448))./4.0;
t9533 = (t5235.*t8062)./4.0;
t9534 = t2106+t9100;
t9538 = t2347+t3394+t3477+t3610+t4363+t4386;
t9541 = (t5115.*t8166)./4.0;
t9542 = -t9529;
t9547 = t8.*t9521;
t9549 = t16.*t9521;
t9552 = t3752.*(t5144-t6902).*(-1.0./4.0);
t9555 = t5083.*(-t1476-t1540+t2091+t2165+t2579+t8.*(t260+t468+t570+t2298)).*(-1.0./4.0);
t9558 = (t5083.*(-t1476-t1540+t2091+t2165+t2579+t8.*(t260+t468+t570+t2298)))./4.0;
t9570 = t7.*t9209.*8.639075e-2;
t9579 = (t6190.*t7245)./2.0;
t9580 = (t6190.*t7245)./4.0;
t9582 = (t5433.*t7940)./4.0;
t9584 = (t4265.*t8711)./4.0;
t9585 = (t6205.*t7224)./4.0;
t9587 = t7.*t9236.*8.639075e-2;
t9588 = (t5434.*t7949)./4.0;
t9590 = (t6190.*t7246)./4.0;
t9598 = (t8433.*(t2904-t2927))./4.0;
t9600 = -t9591;
t9603 = -t9593;
t9605 = -t9594;
t9606 = t8.*t9269.*2.62925e-3;
t9610 = t5331.*(t4542-t6448).*(-1.0./4.0);
t9617 = (t5331.*(t4542-t6448))./4.0;
t9623 = t6190.*(t30.*(t2425-t2468).*1.225946+t68.*(t2425-t2468).*1.225946).*(-1.0./4.0);
t9625 = (t5679.*t7796)./4.0;
t9630 = (t6302.*t7215)./2.0;
t9632 = (t6190.*(t30.*(t2425-t2468).*1.225946+t68.*(t2425-t2468).*1.225946))./4.0;
t9635 = -t9626;
t9640 = (t6552.*(t921+t1317-t5853))./4.0;
t9650 = t6.*t9325.*6.8635e-3;
t9658 = (t6546.*t7039)./4.0;
t9665 = -t9657;
t9668 = -t9660;
t9671 = (t5760.*t7797)./4.0;
t9678 = t4286.*(t5150-t6911).*(-1.0./4.0);
t9684 = (t4286.*(t5150-t6911))./4.0;
t9692 = (t3249.*t9104)./4.0;
t9701 = (t5443.*t8213)./4.0;
t9716 = t5441.*(-t1476-t1540+t2091+t2165+t2579+t8.*(t260+t468+t570+t2298)).*(-1.0./4.0);
t9720 = -t9710;
t9723 = (t4774.*t8711)./2.0;
t9725 = (t5628.*t8065)./4.0;
t9782 = (t6016.*t7796)./4.0;
t9793 = t17.*t9233.*1.13264871585e-2;
t9803 = (t6038.*t7797)./4.0;
t9840 = (t5365.*t8433)./4.0;
t9846 = t5740.*(t4542-t6448).*(-1.0./4.0);
t9851 = t5750.*(t4542-t6448).*(-1.0./4.0);
t9852 = (t5740.*(t4542-t6448))./4.0;
t9854 = t5755.*(t4542-t6448).*(-1.0./4.0);
t9861 = (t5750.*(t4542-t6448))./4.0;
t9865 = (t5755.*(t4542-t6448))./4.0;
t9869 = (t2980.*t9236)./4.0;
t9874 = -t9862;
t9886 = -t9873;
t9888 = (t5739.*t8166)./4.0;
t9889 = (t5740.*t8166)./4.0;
t9890 = -t9876;
t9897 = (t5750.*t8166)./4.0;
t9900 = (t5853.*t8054)./4.0;
t9904 = -t9891;
t9906 = t5826.*(t4542-t6448).*(-1.0./4.0);
t9907 = (t4021.*t9098)./4.0;
t9916 = -t9910;
t9921 = (t5843.*t8166)./4.0;
t9927 = (t7113.*(t921+t1317-t5853))./4.0;
t9929 = -t9925;
t9937 = -t9933;
t9938 = (t7039.*t7124)./4.0;
t9941 = -t9936;
t9946 = (t3275.*t9325)./4.0;
t9947 = (t3249.*t9333)./4.0;
t9953 = t6302.*(t3479-t3544+t2772.*(t48-t349)+t2775.*(t48-t349)).*(-1.0./4.0);
t9960 = (t6302.*(t3479-t3544+t2772.*(t48-t349)+t2775.*(t48-t349)))./4.0;
t9962 = t5912.*(-t1476-t1540+t2091+t2165+t2579+t8.*(t260+t468+t570+t2298)).*(-1.0./4.0);
t9966 = (t5912.*(-t1476-t1540+t2091+t2165+t2579+t8.*(t260+t468+t570+t2298)))./4.0;
t9968 = (t3421.*t9310)./4.0;
t9969 = (t5277.*t8711)./4.0;
t9970 = (t3489.*t9310)./4.0;
t9972 = t6092.*(t4542-t6448).*(-1.0./4.0);
t9978 = t15.*t5628.*(t4542-t6448).*(-3.064865e-1);
t9980 = t7.*t5634.*(t4542-t6448).*(-3.064865e-1);
t9981 = (t6092.*(t4542-t6448))./4.0;
t9984 = t15.*t5628.*(t4542-t6448).*3.064865e-1;
t9986 = t7.*t5634.*(t4542-t6448).*3.064865e-1;
t9992 = t1313+t2434+t2577+t3488+t3541+t3612+t3867+t3922;
t9995 = -t9988;
t10000 = -t9993;
t10001 = (t6302.*t7980)./4.0;
t10002 = -t9994;
t10003 = -t9996;
t10005 = t16.*(-t3045-t3218+t3458+t3539+t3878+t8.*(t260+t468+t570+t2298).*1.666555).*(-2.62925e-3);
t10011 = t16.*(-t3045-t3218+t3458+t3539+t3878+t8.*(t260+t468+t570+t2298).*1.666555).*2.62925e-3;
t10013 = (t6104.*t8191)./4.0;
t10020 = t15.*t5699.*(t4542-t6448).*(-4.1663875e-1);
t10025 = t7.*t6175.*(t4542-t6448).*(-1.0./4.0);
t10028 = t15.*t5699.*(t4542-t6448).*4.1663875e-1;
t10034 = t6222.*(t4542-t6448).*(-1.0./4.0);
t10036 = (t7.*t6175.*(t4542-t6448))./4.0;
t10041 = t15.*t6196.*(t4542-t6448).*(-1.0./4.0);
t10042 = (t3752.*t9333)./4.0;
t10045 = -t10033;
t10046 = (t6222.*(t4542-t6448))./4.0;
t10048 = (t6175.*t8177)./4.0;
t10052 = -t10040;
t10053 = (t4064.*t9236)./4.0;
t10057 = -t10049;
t10061 = -t10055;
t10063 = (t7108.*t7224)./4.0;
t10066 = t6302.*(t2752+t3814-t4385-t9.*t439.*3.127439544e-3).*(-1.0./4.0);
t10067 = (t6223.*t8166)./4.0;
t10068 = (t4024.*t9269)./4.0;
t10076 = (t6196.*t8213)./4.0;
t10077 = (t6302.*(t2752+t3814-t4385-t9.*t439.*3.127439544e-3))./4.0;
t10080 = t9891.*1.666555;
t10081 = t9892.*1.666555;
t10082 = -t10070;
t10086 = (t4255.*t9209)./4.0;
t10091 = t9892.*7.35522e-1;
t10096 = t2038+t2631+t3531+t3538+t4196+t4218+t4457;
t10126 = (t6304.*t8191)./4.0;
t10138 = ((t4542-t6448).*(t985+t3399-t13.*t42.*1.01140545e-1-t7.*t223.*5.034347249e-2))./4.0;
t10144 = (t5583.*t8711)./2.0;
t10145 = (t5583.*t8711)./4.0;
t10154 = -t10150;
t10171 = (t6096.*t8477)./4.0;
t10183 = (t6190.*t8438)./4.0;
t10184 = (t5716.*t8711)./4.0;
t10194 = t2520.*(-t3045-t3218+t3458+t3539+t3878+t8.*(t260+t468+t570+t2298).*1.666555).*(-1.0./4.0);
t10200 = (t2520.*(-t3045-t3218+t3458+t3539+t3878+t8.*(t260+t468+t570+t2298).*1.666555))./4.0;
t10224 = -t10215;
t10244 = (t4837.*t9236)./4.0;
t10257 = (t6535.*t8256)./4.0;
t10263 = t5699.*(t5144-t6902).*(-1.0./4.0);
t10267 = t6.*t9828.*2.46255173325e-2;
t10273 = (t5699.*(t5144-t6902))./4.0;
t10277 = -t10269;
t10287 = t9892.*5.01208083475e-2;
t10288 = (t6190.*t8609)./2.0;
t10289 = (t5884.*t8711)./2.0;
t10298 = t9891.*1.17633784675e-2;
t10306 = (t6302.*t8547)./2.0;
t10314 = (t921+t1317-t5853).*(t2437+t2648+t3129+t3384+t3574).*(-1.0./2.0);
t10315 = t14.*t10094.*6.8635e-3;
t10324 = (t7224.*t7620)./4.0;
t10325 = t6750.*(t4542-t6448).*(-1.0./4.0);
t10332 = t6763.*(t4542-t6448).*(-1.0./4.0);
t10334 = t6767.*(t4542-t6448).*(-1.0./4.0);
t10335 = -t10327;
t10341 = (t6763.*(t4542-t6448))./4.0;
t10344 = (t6767.*(t4542-t6448))./4.0;
t10348 = -t10339;
t10354 = t6677.*(-t1476-t1540+t2091+t2165+t2579+t8.*(t260+t468+t570+t2298)).*(-1.0./4.0);
t10357 = (t6750.*t8166)./4.0;
t10358 = -t10350;
t10360 = -t10353;
t10361 = (t6677.*(-t1476-t1540+t2091+t2165+t2579+t8.*(t260+t468+t570+t2298)))./4.0;
t10363 = (t6767.*t8166)./4.0;
t10364 = (t6762.*t8166)./4.0;
t10366 = (t5095.*t9236)./4.0;
t10367 = (t6114.*t8711)./2.0;
t10368 = (t6190.*t8689)./2.0;
t10380 = (t8044.*(t921+t1317-t5853))./2.0;
t10385 = (t8047.*(t921+t1317-t5853))./4.0;
t10391 = -t10373;
t10400 = t3780.*(-t3045-t3218+t3458+t3539+t3878+t8.*(t260+t468+t570+t2298).*1.666555).*(-1.0./4.0);
t10405 = t6928.*(t4542-t6448).*(-1.0./4.0);
t10408 = t1124+t1306+t1950+t9521;
t10409 = (t6928.*(t4542-t6448))./4.0;
t10417 = (t7039.*t8053)./4.0;
t10429 = (t7039.*t8065)./2.0;
t10432 = -t10422;
t10457 = (t6966.*t8191)./4.0;
t10467 = t15.*t6589.*(t4542-t6448).*(-4.1663875e-1);
t10472 = t15.*t6589.*(t4542-t6448).*4.1663875e-1;
t10473 = t7796.*(t1468-t1988-t2498+t4565+t17.*(t208-t427)).*(-1.0./4.0);
t10479 = -t10477;
t10483 = -t10478;
t10484 = (t8285.*(t921+t1317-t5853))./2.0;
t10494 = -t10492;
t10502 = (t7039.*t8310)./2.0;
t10504 = (t7080.*t8256)./4.0;
t10505 = (t5699.*t9104)./4.0;
t10506 = (t6442.*t8711)./4.0;
t10508 = (t14.*t6430.*t8711)./4.0;
t10521 = t14.*t8711.*(t4540+t5.*(t2425-t2468)).*(-1.0./4.0);
t10531 = (t14.*t8711.*(t4540+t5.*(t2425-t2468)))./4.0;
t10535 = t8711.*(t30.*(t2425-t2468)+t68.*(t2425-t2468)).*(-1.0./4.0);
t10536 = (t5433.*t9233)./4.0;
t10539 = (t8711.*(t30.*(t2425-t2468)+t68.*(t2425-t2468)))./4.0;
t10541 = t7245.*(t4542-t6448).*(-1.0./4.0);
t10545 = (t7245.*(t4542-t6448))./4.0;
t10548 = (t7224.*t8156)./4.0;
t10553 = (t7215.*t8191)./4.0;
t10555 = t4509.*(-t3045-t3218+t3458+t3539+t3878+t8.*(t260+t468+t570+t2298).*1.666555).*(-1.0./4.0);
t10556 = -t10547;
t10562 = -t10551;
t10564 = (t4509.*(-t3045-t3218+t3458+t3539+t3878+t8.*(t260+t468+t570+t2298).*1.666555))./4.0;
t10570 = t4514.*(-t3045-t3218+t3458+t3539+t3878+t8.*(t260+t468+t570+t2298).*1.666555).*(-1.0./4.0);
t10572 = -t10558;
t10575 = t7224.*(-t3405+t4994+t5076).*(-1.0./4.0);
t10585 = (t7224.*(-t3405+t4994+t5076))./4.0;
t10594 = -t10583;
t10621 = t7.*(t4542-t6448).*(t921+t1317-t5853).*(-3.064865e-1);
t10631 = t7.*(t4542-t6448).*(t921+t1317-t5853).*3.064865e-1;
t10635 = (t7227.*t8297)./4.0;
t10640 = t7.*(t6460-t35.*(t2425-t2468)).*(t921+t1317-t5853).*3.064865e-1;
t10641 = (t5648.*t9236)./4.0;
t10648 = -t10634;
t10668 = t15.*t7039.*(t4542-t6448).*(-3.064865e-1);
t10669 = -t10647;
t10671 = -t10650;
t10689 = t15.*t7039.*(t6460-t35.*(t2425-t2468)).*3.064865e-1;
t10691 = -t10686;
t10694 = (t7797.*(t2056+t2203+t2351+t3433+t3503+t16.*t389.*(1.1e+1./1.25e+2)))./4.0;
t10696 = t10141.*(t701-t775).*(-1.0./4.0);
t10705 = (t10141.*(t701-t775))./4.0;
t10721 = (t3365.*t10141)./4.0;
t10726 = (t3455.*t10141)./4.0;
t10755 = (t7797.*t7940)./4.0;
t10758 = (t5853.*t9236)./2.0;
t10760 = (t7796.*t7949)./4.0;
t10767 = (t5860.*t9236)./2.0;
t10778 = t5050.*(-t3045-t3218+t3458+t3539+t3878+t8.*(t260+t468+t570+t2298).*1.666555).*(-1.0./4.0);
t10782 = (t5050.*(-t3045-t3218+t3458+t3539+t3878+t8.*(t260+t468+t570+t2298).*1.666555))./4.0;
t10783 = t3214+t3251+t3654+t3667+t4030+t4640+t5362;
t10790 = t7613.*(-t1476-t1540+t2091+t2165+t2579+t8.*(t260+t468+t570+t2298)).*(-1.0./4.0);
t10793 = t10567.*7.35522e-1;
t10795 = t10569.*7.35522e-1;
t10799 = (t5999.*t9236)./2.0;
t10804 = (t9884.*(t2821-t2864))./4.0;
t10821 = (t4152.*t10141)./4.0;
t10829 = (t5137.*t9828)./4.0;
t10846 = t7039.*(t5150-t6911).*(-1.0./4.0);
t10847 = t8191.*(t3479-t3544+t2772.*(t48-t349)+t2775.*(t48-t349)).*(-1.0./2.0);
t10852 = (t7.*(t4650+t34.*(t2425-t2468)).*1.225946+t47.*(t2425-t2468).*1.225946).*(t921+t1317-t5853).*(-1.0./4.0);
t10864 = (t4611.*t10094)./4.0;
t10867 = (t7039.*t8922)./4.0;
t10875 = (t7980.*t8191)./4.0;
t10878 = t7.*t8050.*(t4542-t6448).*(-1.0./4.0);
t10879 = (t6589.*t9104)./4.0;
t10882 = (t7.*t8050.*(t4542-t6448))./4.0;
t10886 = t15.*t8054.*(t4542-t6448).*(-1.0./4.0);
t10888 = -t10884;
t10890 = (t15.*t8054.*(t4542-t6448))./4.0;
t10891 = -t10887;
t10900 = -t10893;
t10902 = -t10897;
t10910 = t8191.*(t2752+t3814-t4385-t9.*t439.*3.127439544e-3).*(-1.0./2.0);
t10917 = -t10909;
t10918 = (t6302.*t9310)./4.0;
t10921 = -t10912;
t10930 = -t10922;
t10931 = t7151+t8960;
t10932 = t8062.*(-t1476-t1540+t2091+t2165+t2579+t8.*(t260+t468+t570+t2298)).*(-1.0./4.0);
t10937 = (t8062.*(-t1476-t1540+t2091+t2165+t2579+t8.*(t260+t468+t570+t2298)))./4.0;
t10943 = t10567.*3.867742437e-3;
t10951 = t10569.*1.563719772e-3;
t10959 = -t9.*(t8963+t7.*(t5026+t5.*(t2959-t2967)));
t10960 = -t17.*(t8963+t7.*(t5026+t5.*(t2959-t2967)));
t10968 = t15.*t8256.*(t4542-t6448).*(-1.0./4.0);
t10980 = (t15.*t8256.*(t4542-t6448))./4.0;
t11000 = -t10992;
t11009 = (t8213.*t8256)./4.0;
t11029 = (t6535.*t9278)./4.0;
t11034 = (t4964.*t10141)./4.0;
t11067 = t8438.*(t4542-t6448).*(-1.0./4.0);
t11070 = t8437.*(t4542-t6448).*(-1.0./4.0);
t11071 = (t8438.*(t4542-t6448))./4.0;
t11076 = (t8437.*(t4542-t6448))./4.0;
t11078 = -t11075;
t11079 = (t5755.*t9828)./4.0;
t11082 = -t11077;
t11084 = -t11080;
t11088 = (t6589.*t9333)./2.0;
t11090 = (t8166.*t8437)./4.0;
t11092 = (t6654.*t9278)./2.0;
t11105 = t5923.*(-t3045-t3218+t3458+t3539+t3878+t8.*(t260+t468+t570+t2298).*1.666555).*(-1.0./4.0);
t11110 = (t5826.*t9828)./4.0;
t11114 = t5952.*(-t3045-t3218+t3458+t3539+t3878+t8.*(t260+t468+t570+t2298).*1.666555).*(-1.0./4.0);
t11120 = (t5952.*(-t3045-t3218+t3458+t3539+t3878+t8.*(t260+t468+t570+t2298).*1.666555))./4.0;
t11121 = -t11116;
t11134 = t6014.*(-t3045-t3218+t3458+t3539+t3878+t8.*(t260+t468+t570+t2298).*1.666555).*(-1.0./4.0);
t11143 = t8609.*(t4542-t6448).*(-1.0./4.0);
t11150 = (t8609.*(t4542-t6448))./4.0;
t11151 = (t8191.*t8547)./4.0;
t11160 = (t5290.*t10141)./4.0;
t11162 = (t9209.*(t921+t1317-t5853))./2.0;
t11164 = t9.*(t8963+t7.*(t5026+t5.*(t2959-t2967))).*(-7.35522e-1);
t11165 = t17.*(t8963+t7.*(t5026+t5.*(t2959-t2967))).*(-7.35522e-1);
t11168 = -t11155;
t11185 = (t6988.*t9236)./2.0;
t11194 = -t11191;
t11207 = t14.*t10964.*6.8635e-3;
t11208 = t6.*t10966.*6.8635e-3;
t11221 = (t3424.*t10769)./4.0;
t11232 = t8689.*(t4542-t6448).*(-1.0./4.0);
t11239 = (t8689.*(t4542-t6448))./4.0;
t11251 = -t11244;
t11255 = t8711.*(t4542-t6448).*(-1.0./4.0);
t11256 = t7.*t10850.*1.059103943995e-1;
t11257 = (t7080.*t9278)./4.0;
t11268 = (t6222.*t9828)./4.0;
t11272 = (t8711.*(t6460-t35.*(t2425-t2468)))./4.0;
t11277 = -t11269;
t11287 = t15.*t10858.*1.059103943995e-1;
t11290 = (t8166.*t8711)./4.0;
t11299 = (t5524.*t10141)./4.0;
t11309 = (t5552.*t10141)./4.0;
t11336 = t2909+t2982+t3312+t3576+t9300;
t11343 = t2854+t3189+t3290+t3626+t9301;
t11358 = (t4879.*t10501)./4.0;
t11388 = t9.*(t8963+t7.*(t5026+t5.*(t2959-t2967))).*(-3.867742437e-3);
t11389 = (t4917.*t10501)./4.0;
t11393 = t15.*(t8963+t7.*(t5026+t5.*(t2959-t2967))).*(-1.059103943995e-1);
t11397 = (t10501.*(t2812-t2860))./4.0;
t11398 = t17.*(t8963+t7.*(t5026+t5.*(t2959-t2967))).*(-1.563719772e-3);
t11401 = t15.*(t8963+t7.*(t5026+t5.*(t2959-t2967))).*1.059103943995e-1;
t11408 = (t2561.*t10964)./4.0;
t11418 = (t2568.*t10966)./4.0;
t11459 = -t11458;
